simulink library "Centralized_I_Lib_Controller"  (R2024b)
(part 6 of 7)

[dq1,dq2,dq3,dq4,dq5,dq6,t10,t1001,t1002,t1003,t1004,t1005,t1006,t1007,t1009,t101,t1010,t1023,t1024,t1025,t1026,t1027,t1029,t1030,t1032,t1033,t1034,t1035,t1037,t1038,t1039,t1041,t1042,t1043,t1046,t1047,t1048,t105,t1053,t106,t1063,t1068,t1069,t107,t1070,t1071,t1073,t1074,t1075,t1076,t1077,t1078,t1079,t108,t1080,t1081,t1083,t1084,t1086,t1087,t1089,t109,t1090,t1091,t1092,t1095,t1096,t1097,t1098,t11,t110,t1100,t1103,t111,t1115,t1116,t1117,t1118,t1119,t112,t1120,t1122,t1123,t1124,t1126,t1127,t1128,t1129,t113,t1130,t1131,t1132,t1133,t1134,t114,t1148,t1149,t1150,t1151,t1152,t1153,t1155,t1156,t1157,t1158,t1159,t1160,t1162,t1163,t1164,t1166,t1169,t1170,t1171,t1172,t1173,t1174,t1179,t1180,t1182,t1183,t1186,t1187,t1188,t1189,t1191,t1192,t1193,t1194,t1195,t1196,t1198,t1199,t12,t1201,t1202,t1203,t1204,t1205,t1206,t1207,t1208,t1210,t1211,t1212,t1214,t1215,t1217,t1218,t1219,t1220,t1221,t1222,t1224,t1227,t1228,t1229,t123,t1230,t1231,t1233,t1234,t1235,t1239,t124,t1240,t1241,t1242,t1243,t1244,t1245,t1246,t1247,t125,t1250,t1251,t1252,t1253,t1254,t1256,t126,t1263,t1266,t127,t1274,t128,t1284,t1285,t1287,t1288,t1289,t129,t1290,t1291,t1293,t1295,t1296,t1297,t1298,t1299,t13,t130,t1300,t1301,t1308,t1309,t1313,t1317,t1318,t1319,t1320,t1323,t1324,t1325,t1326,t1327,t1328,t1329,t1331,t1332,t1333,t1334,t1339,t1343,t1344,t1345,t1346,t1347,t1349,t1351,t1352,t1353,t1354,t1356,t1357,t1358,t1359,t1360,t1361,t1362,t1363,t1364,t1365,t1366,t1368,t1369,t137,t1371,t1373,t1375,t1376,t1377,t1378,t1379,t1380,t1383,t1385,t1386,t1387,t1388,t1389,t1390,t1391,t1392,t1393,t1394,t1395,t1396,t1397,t1398,t1399,t140,t1405,t1406,t141,t1410,t1411,t1412,t1413,t1414,t1415,t1416,t1417,t1419,t1420,t1421,t1422,t1423,t1424,t1426,t1427,t1428,t1429,t143,t1430,t1431,t1432,t1433,t1434,t1435,t1438,t1439,t1440,t1441,t1442,t1443,t1445,t1446,t1448,t1450,t1452,t1453,t1455,t1456,t1457,t1458,t1459,t1460,t1461,t1462,t1463,t1464,t1465,t1466,t1467,t1468,t1469,t1470,t1473,t1477,t1479,t1480,t1481,t1482,t1484,t1488,t1490,t1491,t1492,t1493,t1494,t1495,t1496,t1500,t1505,t1507,t1508,t1510,t1511,t1512,t1513,t1516,t1517,t1518,t1519,t1522,t1523,t1524,t1525,t1526,t1528,t1541,t1542,t1543,t1545,t1546,t1547,t1548,t1549,t1551,t1552,t1553,t1554,t1555,t1556,t1557,t1558,t1559,t1560,t1571,t1572,t1573,t1575,t1576,t1577,t1578,t1579,t1580,t1581,t1582,t1583,t1584,t1585,t1586,t1587,t159,t1592,t1594,t1595,t1596,t1606,t1609,t1610,t1611,t1613,t1615,t1619,t162,t1620,t163,t1636,t1637,t1639,t164,t1641,t1642,t1643,t1644,t1645,t1646,t165,t1653,t1655,t1656,t1659,t166,t1660,t1661,t1662,t1663,t1664,t1665,t1666,t1668,t1669,t167,t1670,t1671,t1672,t1673,t1675,t1676,t1677,t1678,t1679,t168,t1680,t1681,t1682,t1684,t1685,t1686,t1687,t1688,t1689,t1690,t1691,t1692,t1693,t1694,t1696,t1697,t1698,t1700,t1701,t1702,t1703,t1705,t1706,t1707,t1709,t1710,t1711,t1713,t1716,t1717,t1718,t1719,t1720,t1721,t1723,t1726,t1727,t1728,t1730,t1732,t1735,t1739,t1744,t1745,t1749,t1750,t1751,t1752,t1753,t1754,t1755,t1756,t1758,t1759,t1760,t1761,t1762,t1763,t1764,t1766,t1768,t177,t1771,t1772,t1773,t1776,t1777,t1778,t1779,t178,t1785,t1787,t1789,t179,t1790,t1795,t1796,t1799,t18,t1800,t1801,t1803,t1804,t1806,t1815,t1816,t1817,t1818,t1819,t182,t1820,t1821,t1822,t1823,t1824,t1825,t1826,t1827,t1828,t1829,t183,t1830,t1831,t1832,t1833,t1835,t1836,t1837,t1839,t184,t1840,t1841,t1842,t1843,t1844,t1845,t1847,t1848,t1849,t185,t1850,t1851,t1852,t1853,t1854,t1856,t1857,t1858,t186,t1860,t1861,t1864,t1865,t1866,t1867,t1868,t1869,t187,t1874,t1876,t1877,t1878,t1879,t188,t1882,t1883,t1889,t189,t1893,t1895,t1896,t1897,t1898,t1899,t19,t1900,t1901,t1902,t1903,t1904,t1905,t1906,t1907,t1908,t1909,t191,t1911,t1912,t1913,t1914,t1917,t1919,t1920,t1921,t1922,t1925,t1926,t1928,t193,t1930,t1931,t1933,t1934,t1935,t1936,t1937,t1939,t194,t1942,t1943,t1944,t1947,t1949,t195,t1955,t1958,t1959,t1962,t1964,t1966,t1973,t1991,t1992,t1993,t1994,t1995,t1996,t1997,t1998,t2,t20,t200,t2000,t2001,t2002,t2003,t2004,t2005,t2006,t2009,t2010,t2012,t2013,t2014,t2015,t2016,t2017,t2018,t202,t2020,t2021,t2023,t2024,t2025,t2027,t2028,t2029,t203,t2030,t2034,t2036,t2037,t2038,t2039,t204,t2040,t2043,t2044,t2045,t2050,t2053,t2054,t2055,t2056,t2058,t2059,t2061,t2063,t2066,t2067,t2068,t2069,t2072,t2074,t2075,t2078,t2079,t208,t2080,t2083,t2084,t2085,t2086,t2087,t2088,t2089,t2090,t2092,t2094,t2096,t2097,t21,t210,t2103,t2107,t2109,t211,t2110,t2111,t2112,t2115,t2116,t2117,t2118,t212,t2120,t2121,t2123,t2124,t2125,t2126,t2127,t2129,t2132,t2133,t2134,t2135,t2136,t2138,t2139,t214,t2140,t2141,t2147,t2148,t2149,t215,t2150,t2151,t2152,t2157,t2158,t2159,t216,t2161,t2168,t2169,t2171,t2178,t2179,t2181,t2185,t2191,t2193,t22,t2200,t2201,t2202,t2203,t2204,t2205,t2206,t2207,t2208,t2212,t2214,t2216,t2217,t2219,t2220,t2221,t2222,t2223,t2224,t2225,t2227,t2228,t2229,t2231,t2233,t2234,t2235,t2236,t2237,t2238,t2239,t224,t2245,t2246,t2247,t2248,t2250,t2252,t2254,t2258,t2259,t2262,t227,t2271,t2272,t2273,t2274,t2276,t2277,t228,t2280,t2281,t2283,t2284,t2285,t2287,t229,t2290,t2292,t2293,t2295,t230,t2303,t2304,t2305,t2307,t2308,t231,t2310,t2314,t2318,t2319,t2320,t2322,t2323,t2324,t2325,t2326,t2327,t2336,t234,t2342,t2343,t2347,t2348,t2349,t2350,t2353,t2357,t2358,t2362,t2363,t2364,t237,t2370,t2372,t2373,t2375,t2378,t2379,t2381,t2382,t2383,t2385,t2387,t2394,t2395,t2396,t2397,t2398,t2400,t2401,t2403,t2404,t2405,t2409,t2410,t2411,t2412,t2413,t2414,t2415,t2416,t2417,t2419,t242,t2421,t2422,t2423,t2425,t2426,t243,t2430,t2431,t2432,t2433,t2436,t2437,t2438,t2439,t244,t2440,t2445,t2446,t2447,t2449,t245,t2450,t2451,t2452,t2453,t2454,t2455,t2456,t2457,t2459,t246,t2462,t2463,t2464,t2465,t2466,t2467,t2469,t247,t2470,t2471,t2472,t2473,t2474,t2475,t2477,t2478,t2479,t248,t2480,t2481,t2482,t2483,t2484,t2485,t2486,t2487,t2488,t249,t2491,t2498,t2499,t25,t250,t2500,t2501,t2504,t2506,t2507,t2508,t2509,t251,t2515,t252,t2524,t2525,t2527,t2529,t253,t2531,t2536,t2542,t2543,t2546,t255,t2551,t2552,t2553,t2555,t2559,t256,t2560,t2564,t2565,t2566,t2567,t2568,t2569,t2571,t2572,t2574,t2575,t2576,t2578,t2580,t2581,t2582,t2583,t2585,t2586,t2588,t259,t2591,t2593,t2594,t2595,t2598,t2599,t26,t260,t2600,t2601,t2603,t2604,t2605,t2607,t2608,t2609,t261,t2610,t2611,t2612,t2614,t2615,t2617,t2618,t262,t2621,t2622,t2625,t2628,t2629,t263,t2632,t2634,t2641,t2643,t2644,t2645,t2646,t2648,t2649,t265,t2650,t2651,t2652,t2655,t2656,t2657,t2658,t2659,t2660,t2661,t2662,t2663,t2667,t267,t2672,t2673,t2674,t2675,t2679,t2680,t269,t2691,t2692,t2694,t2695,t2698,t27,t2700,t2701,t2702,t2703,t2705,t2711,t2712,t2713,t2714,t2715,t2716,t2718,t2719,t2720,t2721,t2722,t2725,t2726,t2727,t2729,t2730,t2732,t2733,t2734,t2735,t2736,t2738,t2739,t274,t2740,t2741,t2743,t2747,t2748,t2749,t2752,t2753,t2755,t2756,t276,t2760,t2761,t2763,t2764,t2765,t2766,t2767,t2769,t277,t2770,t2772,t278,t2782,t2783,t2784,t2785,t2786,t2789,t279,t2792,t2793,t2794,t2795,t2796,t28,t2800,t2801,t2803,t2804,t2806,t2809,t281,t2811,t2812,t2813,t2815,t2816,t2817,t2819,t2820,t2821,t2822,t2825,t2827,t2828,t2829,t283,t2830,t2832,t2833,t2834,t2836,t2837,t2839,t2840,t2843,t2844,t2848,t2849,t285,t2850,t2852,t2854,t2855,t2856,t286,t2860,t2861,t2862,t2863,t2864,t2865,t2866,t2867,t2869,t287,t2872,t2873,t2877,t2878,t288,t2880,t2882,t2887,t2888,t2890,t2892,t2894,t2895,t2899,t29,t2900,t2901,t2902,t2903,t2904,t2905,t2906,t2910,t2911,t2912,t2915,t2916,t2917,t2919,t292,t2921,t2922,t2923,t2924,t2925,t2926,t2927,t2928,t2929,t293,t2931,t2932,t2933,t2934,t2937,t2938,t2939,t2940,t2942,t2943,t2944,t2949,t295,t2950,t2951,t2952,t2953,t2954,t2956,t2957,t2959,t296,t2960,t2962,t2964,t2965,t2968,t2969,t297,t2970,t2973,t2975,t2977,t298,t2981,t2984,t2986,t2988,t2989,t299,t2990,t2991,t2992,t2993,t2995,t2996,t2997,t3,t300,t3002,t3003,t3004,t3006,t3007,t3008,t3009,t301,t3010,t3011,t3012,t3013,t3015,t3016,t3018,t3019,t3025,t3026,t3028,t303,t3030,t3033,t3034,t3035,t3037,t3039,t304,t3040,t3043,t3045,t3046,t3047,t3049,t305,t3050,t3054,t3056,t3058,t3059,t3060,t3061,t3063,t3064,t3065,t3066,t3067,t3068,t3069,t3070,t3071,t3072,t3073,t3074,t3075,t3076,t3077,t3078,t3079,t308,t3085,t3087,t3088,t3089,t309,t3090,t3091,t3092,t3094,t3095,t3096,t3097,t3098,t3099,t3100,t3101,t3102,t3104,t3106,t3108,t3109,t311,t3110,t3111,t3112,t3119,t312,t3121,t3123,t3124,t3125,t3129,t313,t3130,t3131,t3133,t3136,t3138,t3139,t314,t3144,t3146,t3147,t3148,t3149,t3150,t3152,t3153,t3154,t3159,t3164,t3170,t3173,t3174,t3177,t3180,t3181,t3185,t3186,t3187,t3188,t3189,t3192,t3193,t3194,t3195,t3198,t3200,t3201,t3202,t3203,t3204,t3205,t3206,t3207,t3208,t3209,t3210,t3211,t3212,t3213,t3214,t3215,t3216,t3217,t3218,t3219,t3220,t3222,t3223,t3224,t3225,t3226,t3227,t3228,t3231,t3232,t3233,t3234,t3235,t3236,t3237,t3238,t3239,t3242,t3245,t3246,t3247,t3249,t3250,t3252,t3253,t3254,t3255,t3256,t3258,t3260,t3262,t3265,t3269,t3270,t3271,t3273,t3274,t3275,t328,t3280,t3281,t3282,t3283,t3284,t3286,t3287,t3288,t329,t3296,t3297,t3298,t330,t3300,t3303,t3304,t3305,t3306,t3307,t3308,t331,t3315,t3316,t3318,t332,t3322,t3323,t3324,t3326,t3327,t3328,t3329,t333,t3330,t3331,t3332,t3333,t3334,t3335,t3336,t3339,t334,t3342,t3345,t3346,t3347,t3348,t3352,t3353,t3356,t3358,t3359,t336,t3361,t3362,t3363,t3364,t3365,t3366,t3367,t337,t3372,t3374,t3375,t3377,t3378,t3379,t338,t3380,t3384,t3385,t3386,t3387,t339,t3394,t3395,t3396,t3397,t3399,t3401,t3402,t3405,t341,t3410,t3411,t3412,t3413,t3414,t3416,t3419,t342,t3421,t3422,t3424,t3425,t3426,t3427,t343,t3430,t3435,t3436,t3437,t3438,t3439,t344,t3440,t3442,t3443,t3444,t3445,t3446,t3449,t345,t3452,t3453,t3454,t3455,t3456,t3458,t3459,t346,t3463,t3466,t3467,t347,t3470,t3471,t3472,t3473,t3474,t3475,t3476,t3477,t348,t3480,t3481,t3482,t3483,t3484,t3485,t3487,t3488,t3489,t349,t3491,t3492,t3493,t3494,t3496,t3498,t3499,t350,t3501,t3502,t3504,t3506,t3507,t3508,t3509,t3511,t3512,t3513,t3515,t3516,t3519,t352,t3520,t3521,t3522,t3523,t3526,t3527,t3528,t3529,t353,t3531,t3532,t3533,t3535,t3536,t3537,t3538,t354,t3541,t3542,t3543,t3544,t3545,t3548,t3549,t355,t3552,t3553,t3554,t3555,t3559,t356,t3561,t3564,t3565,t3566,t3567,t3568,t3569,t357,t3571,t3573,t3575,t3576,t3578,t3579,t358,t3582,t3586,t3587,t3588,t3590,t3591,t3592,t3593,t3596,t3598,t3599,t360,t3600,t3601,t3602,t3603,t3604,t3606,t3608,t3609,t3610,t3611,t3612,t3613,t3614,t3615,t3617,t3620,t3621,t3622,t3623,t3626,t3627,t3628,t3629,t3630,t3631,t3632,t3633,t3634,t3636,t3638,t3639,t3640,t3641,t3642,t3643,t3645,t3646,t3648,t3649,t3650,t3652,t3653,t3654,t3655,t3656,t3657,t3658,t3660,t3663,t3667,t3668,t3670,t3671,t3673,t3674,t3675,t3676,t3677,t3679,t3680,t3681,t3682,t3683,t3684,t3686,t3687,t3688,t3689,t369,t3690,t3691,t3692,t3694,t3695,t3696,t3697,t3698,t3699,t370,t3700,t3701,t3702,t3703,t3704,t3705,t3708,t3709,t3710,t3711,t3712,t3713,t3714,t3715,t3717,t3718,t3719,t372,t3720,t3721,t3722,t3723,t3724,t3725,t3726,t3727,t3728,t3729,t373,t3730,t3732,t3733,t3734,t3735,t3736,t3737,t3738,t3739,t374,t3740,t3741,t3742,t3743,t3744,t3745,t3747,t3748,t3749,t375,t3750,t3751,t3752,t3754,t3755,t3756,t3757,t3758,t3759,t376,t3760,t3763,t3764,t3765,t3766,t3767,t3768,t3769,t3770,t3771,t3772,t3774,t3775,t3776,t3777,t3778,t3780,t3781,t3782,t3785,t3786,t3787,t3789,t379,t3790,t3792,t3793,t3794,t3796,t3798,t380,t3801,t3802,t3804,t3805,t3806,t3807,t3808,t3809,t3810,t3811,t3812,t3813,t3814,t3815,t3816,t3817,t3818,t3820,t3821,t3822,t3823,t3824,t3825,t3826,t3827,t3828,t3829,t3831,t3832,t3833,t3837,t3838,t3839,t384,t3840,t3841,t3846,t3847,t3848,t3849,t3850,t3851,t3852,t3854,t3856,t3857,t386,t3860,t3861,t3862,t3863,t3864,t3865,t3868,t3869,t387,t3871,t3872,t3874,t3875,t3876,t3878,t388,t3882,t3884,t3885,t3886,t3887,t3888,t3889,t389,t3890,t3891,t3892,t3893,t3894,t3895,t3896,t3897,t3898,t3899,t3900,t3901,t3902,t3903,t3904,t3906,t3908,t3909,t3910,t3912,t3913,t3915,t3916,t3917,t3918,t3919,t3920,t3921,t3922,t3923,t3924,t3925,t3926,t3927,t3928,t393,t3930,t3931,t3932,t3935,t3936,t3939,t3941,t3944,t3945,t3946,t3947,t3948,t3949,t395,t3950,t3951,t3953,t3954,t3955,t3956,t3957,t3959,t3960,t3964,t3965,t3966,t3967,t3968,t397,t3970,t3971,t3972,t3976,t3977,t3981,t3982,t3985,t3988,t3989,t399,t3990,t3993,t3994,t3995,t3998,t3999,t4,t400,t4000,t4001,t4002,t4003,t4005,t4006,t4007,t4009,t401,t4011,t4012,t4013,t4014,t4015,t4016,t4017,t4018,t4019,t402,t4022,t4025,t4026,t4028,t4029,t4031,t4032,t4033,t4034,t4035,t4036,t4037,t404,t4041,t4042,t4043,t4044,t4046,t4047,t4048,t405,t4053,t4055,t4056,t4057,t4058,t4059,t4060,t4061,t4062,t4063,t4064,t4065,t4066,t4067,t4068,t407,t4070,t4074,t4075,t4077,t4078,t4079,t408,t4080,t4081,t4082,t4083,t4084,t4085,t4087,t4088,t4089,t4090,t4091,t4092,t4095,t4097,t4099,t410,t4103,t4104,t4105,t4109,t4113,t4115,t4116,t4118,t4119,t4120,t4121,t4122,t4123,t4125,t4126,t4127,t4129,t413,t4131,t4132,t4133,t4134,t4136,t4137,t4138,t4139,t414,t4140,t4142,t4143,t4145,t4147,t4148,t4149,t415,t4150,t4151,t4152,t4153,t4154,t4156,t4159,t416,t4161,t4162,t4165,t4168,t4171,t4172,t4174,t4175,t4176,t4178,t418,t4183,t4185,t4186,t4188,t419,t4190,t4191,t4192,t4194,t4195,t4197,t4198,t4199,t4200,t4202,t4203,t4204,t4206,t4208,t4209,t421,t4210,t4211,t4212,t4213,t4216,t4217,t4218,t4219,t4220,t4221,t4222,t4223,t4224,t4225,t4226,t4230,t4231,t4232,t4233,t4234,t4235,t4238,t4240,t4241,t4242,t4243,t4244,t4245,t4246,t4247,t4248,t4249,t425,t4250,t4251,t4252,t4255,t4256,t4257,t4258,t4259,t4260,t4261,t4262,t4263,t4264,t4265,t4268,t4269,t4270,t4271,t4274,t4275,t4276,t4277,t4278,t4279,t4280,t4282,t4283,t4284,t4286,t4287,t4288,t4292,t4294,t4295,t4296,t4300,t4301,t4305,t4308,t4309,t4310,t4311,t4312,t4313,t4316,t4317,t4318,t4319,t432,t4320,t4323,t4324,t4325,t4326,t4327,t4328,t4329,t433,t4330,t4331,t4332,t4333,t4334,t4335,t4336,t4338,t434,t4341,t4342,t4343,t4344,t4345,t4347,t435,t4350,t4352,t4354,t436,t4361,t4362,t4364,t4365,t4366,t4367,t4368,t4369,t437,t4370,t4371,t4372,t4374,t4375,t4376,t4377,t4378,t4379,t4380,t4381,t4384,t4385,t4386,t4387,t4388,t4389,t439,t4390,t4391,t4392,t4393,t4394,t4396,t4399,t440,t4400,t4402,t4403,t4405,t4406,t4407,t4408,t4409,t441,t4410,t4414,t4415,t4416,t4417,t4418,t4419,t4420,t4421,t4422,t4423,t4424,t4426,t4428,t4429,t443,t4430,t4433,t4435,t4436,t4438,t4439,t444,t4440,t4442,t4444,t4445,t4448,t4449,t4451,t4452,t4454,t4455,t4456,t4457,t4458,t4459,t446,t4463,t4466,t4469,t4470,t4471,t4473,t4474,t4475,t4476,t4477,t4478,t4479,t4482,t4483,t4484,t4487,t4488,t4493,t4495,t4496,t4497,t4498,t4499,t4503,t4505,t4507,t4508,t4511,t4512,t4513,t4514,t4515,t4516,t4517,t4518,t4519,t4520,t4521,t4526,t4528,t4529,t453,t4531,t4532,t4533,t4534,t4535,t4536,t4537,t4538,t4539,t4540,t4541,t4542,t4543,t4544,t4545,t4546,t4547,t4549,t4550,t4551,t4554,t4555,t4556,t4557,t4558,t4559,t4561,t4562,t4563,t4564,t4565,t4566,t4567,t4568,t4569,t4570,t4571,t4572,t4573,t4574,t4575,t4576,t4578,t4579,t4580,t4581,t4582,t4584,t4585,t4589,t4590,t4592,t4593,t4594,t4595,t4597,t4598,t4599,t460,t4601,t4602,t4603,t4604,t4606,t4608,t4609,t4610,t4611,t4612,t4613,t4614,t4615,t4616,t4617,t4618,t4619,t4620,t4621,t4622,t4623,t4625,t4626,t4627,t4628,t4629,t463,t4631,t4632,t4633,t4636,t4639,t4640,t4641,t4642,t4644,t4645,t4647,t4648,t4649,t465,t4650,t4651,t4652,t4653,t4655,t4656,t4658,t4660,t4661,t4664,t4665,t4666,t4669,t4670,t4671,t4672,t4673,t4674,t4675,t4676,t4679,t4683,t4685,t4686,t4691,t4692,t4694,t4695,t4697,t4698,t4699,t4702,t4704,t4706,t4710,t4712,t4713,t4714,t4717,t4718,t4719,t472,t4720,t4722,t4723,t4726,t4729,t4730,t4731,t4732,t4733,t4735,t4736,t4737,t4738,t4739,t4740,t4742,t4743,t4744,t4746,t4747,t4749,t475,t4750,t4751,t4753,t4754,t4756,t4757,t4759,t4760,t4761,t4762,t4763,t4764,t4765,t4766,t4767,t4768,t4769,t4770,t4771,t4772,t4773,t4774,t4775,t4776,t4777,t4778,t4779,t478,t4780,t4781,t4782,t4783,t4784,t4785,t4786,t4787,t4789,t4791,t4792,t4793,t4794,t4795,t4797,t4798,t4799,t48,t4800,t4801,t4802,t4804,t4805,t4806,t4807,t4808,t4811,t4812,t4813,t4814,t4815,t4816,t4817,t4818,t4819,t4820,t4821,t4822,t4823,t4824,t4825,t4826,t4827,t4828,t4829,t4830,t4831,t4832,t4833,t4835,t4837,t4838,t4840,t4841,t4842,t4844,t4845,t4846,t4847,t4849,t4850,t4851,t4852,t4853,t4854,t4855,t4856,t4857,t4858,t4859,t4860,t4861,t4862,t4863,t4864,t4865,t4867,t4868,t4869,t4870,t4872,t4873,t4874,t4875,t4876,t4879,t488,t4880,t4881,t4883,t4884,t4885,t4886,t4887,t4888,t4889,t4892,t4895,t4896,t4898,t49,t490,t4903,t4905,t4906,t4907,t4908,t4909,t491,t4910,t4911,t4912,t4913,t4914,t4915,t4916,t4917,t4918,t4919,t4920,t4921,t4923,t4924,t4925,t4926,t4927,t4928,t4929,t4930,t4931,t4932,t4933,t4934,t4935,t4937,t4938,t494,t4940,t4942,t4943,t4946,t4948,t4949,t4950,t4953,t4955,t4957,t4958,t496,t4961,t4962,t4964,t4965,t4967,t4968,t497,t4970,t4971,t4972,t4973,t4975,t4976,t4977,t4978,t4979,t498,t4980,t4983,t4984,t4985,t4987,t4988,t499,t4990,t4991,t4992,t4995,t4996,t4998,t5,t50,t500,t5000,t5001,t5003,t5006,t5007,t5009,t501,t5010,t5012,t5014,t5015,t5016,t502,t5020,t5022,t5024,t5025,t5026,t5027,t5030,t5032,t5033,t5034,t5035,t5036,t5038,t5039,t504,t5041,t5042,t5043,t5044,t5045,t5046,t5047,t5048,t505,t5051,t5052,t5054,t5055,t5056,t5058,t5059,t5060,t5061,t5062,t5063,t5064,t5065,t5066,t5067,t5068,t5069,t5070,t5071,t5072,t5073,t5074,t5075,t5076,t5077,t5079,t508,t5080,t5081,t5082,t5083,t5084,t5085,t5086,t5087,t5089,t509,t5090,t5091,t5094,t5095,t5097,t5099,t51,t510,t5100,t5101,t5102,t5105,t5108,t5109,t511,t5111,t5114,t5115,t5116,t5117,t5118,t5119,t512,t5120,t5121,t5122,t5125,t5126,t5127,t5129,t5131,t5132,t5133,t5135,t5136,t5137,t5138,t5139,t514,t5140,t5141,t5143,t5144,t5145,t5146,t5147,t5148,t5149,t515,t5150,t5151,t5153,t5154,t5156,t5158,t516,t5161,t5163,t5164,t5165,t5166,t5167,t5168,t5169,t517,t5170,t5173,t5174,t5176,t5179,t518,t5180,t5181,t5185,t5186,t5187,t5188,t5189,t5190,t5191,t5193,t5194,t5195,t5196,t5200,t5202,t5203,t5207,t5208,t5209,t521,t5210,t5213,t5215,t5216,t5218,t5219,t5221,t5222,t5223,t5224,t5225,t5227,t5229,t523,t5231,t5235,t5236,t5239,t524,t5241,t5242,t5243,t5244,t5245,t5246,t5247,t5250,t5251,t5252,t5253,t5257,t5258,t5259,t5263,t5264,t5265,t5266,t5269,t527,t5274,t5276,t5277,t5278,t5279,t528,t5280,t5281,t5283,t5284,t5285,t5288,t5289,t529,t5290,t5291,t5292,t5293,t5294,t5295,t5296,t5297,t5298,t5299,t53,t530,t5300,t5301,t5302,t5303,t5304,t5305,t5306,t5307,t5308,t5309,t531,t5310,t5312,t5317,t5319,t5322,t5324,t5325,t5326,t5328,t5329,t5330,t5332,t5333,t5334,t5336,t5338,t5339,t534,t5340,t5341,t5342,t5343,t5344,t5345,t5348,t5349,t535,t5350,t5353,t5354,t5355,t5356,t5357,t5358,t5359,t536,t5360,t5361,t5362,t5363,t5364,t5365,t5366,t5369,t5370,t5371,t5372,t5374,t5375,t5376,t5377,t5380,t5382,t5383,t5384,t5385,t5386,t5387,t5388,t5389,t539,t5390,t5391,t5392,t5393,t5394,t5395,t5396,t5397,t5398,t5399,t54,t540,t5400,t5401,t5402,t5403,t5405,t5406,t5407,t5408,t5409,t5410,t5411,t5412,t5413,t5414,t5415,t5416,t5417,t5418,t5419,t542,t5420,t5421,t5422,t5423,t5424,t5425,t5426,t5427,t5428,t5429,t543,t5431,t5432,t5433,t5435,t5436,t5439,t5441,t5442,t5444,t5445,t5446,t5447,t5448,t5449,t5450,t5451,t5452,t5453,t5454,t5455,t5456,t5457,t5458,t5459,t5460,t5461,t5465,t5467,t5468,t5469,t547,t5471,t5472,t5473,t5474,t5475,t5476,t5477,t5478,t548,t5480,t5482,t5483,t5484,t5486,t5490,t5491,t5492,t5493,t5494,t5495,t5496,t5497,t5498,t5499,t55,t5500,t5501,t5502,t5503,t5504,t5505,t5506,t5507,t5508,t5509,t5510,t5511,t5512,t5513,t5514,t5517,t5518,t5519,t5522,t5526,t5527,t5528,t5529,t553,t5530,t5531,t5532,t5533,t5534,t5536,t5537,t5538,t5539,t5540,t5542,t5543,t5544,t5545,t5546,t5547,t5548,t5549,t555,t5550,t5551,t5552,t5553,t5554,t5556,t5557,t5559,t556,t5561,t5562,t5563,t5564,t557,t5573,t5574,t5575,t5576,t5577,t5578,t5579,t558,t5581,t5582,t5583,t5584,t5586,t5587,t5588,t5589,t559,t5590,t5591,t5592,t5593,t5594,t5595,t5596,t5597,t5598,t5599,t56,t560,t5600,t5601,t5602,t5603,t5604,t5605,t5606,t5607,t5608,t5609,t561,t5611,t5612,t5613,t5614,t5615,t5616,t5617,t5618,t5619,t562,t5620,t5621,t5622,t5625,t5627,t5628,t5629,t5630,t5631,t5632,t5634,t5635,t5636,t5637,t5638,t5639,t5644,t5646,t5647,t5648,t5649,t565,t5650,t5651,t5652,t5653,t5654,t5656,t5657,t5658,t5659,t566,t5660,t5661,t5662,t5663,t5664,t5665,t5670,t5671,t5673,t5674,t5675,t5676,t5677,t5678,t5679,t5680,t5681,t5683,t5684,t5685,t5686,t569,t5690,t5692,t5696,t5697,t5698,t5699,t57,t5701,t5702,t5703,t5704,t5705,t5706,t5710,t5711,t5713,t5715,t5716,t5717,t5718,t5719,t5720,t5722,t5723,t5724,t5725,t5726,t5727,t5728,t5729,t5730,t5731,t5732,t5733,t5734,t5735,t5736,t5737,t5741,t5744,t5745,t5747,t5748,t5749,t5750,t5752,t5753,t5755,t5756,t5757,t5759,t5761,t5762,t5763,t5764,t5766,t5767,t5770,t5771,t5773,t5774,t5775,t5776,t5777,t5778,t5779,t5780,t5781,t5783,t5784,t5785,t5786,t5788,t5789,t5792,t5796,t5797,t58,t5800,t5801,t5802,t5803,t5804,t5805,t5806,t5807,t5808,t5809,t5810,t5811,t5812,t5813,t5814,t5815,t5816,t5817,t5818,t5819,t5820,t5822,t5823,t5824,t5825,t5826,t5827,t5828,t5829,t5831,t5832,t5833,t5835,t5836,t5837,t5838,t5840,t5841,t5842,t5843,t5844,t5845,t5847,t5849,t5850,t5851,t5853,t5854,t5855,t5857,t5859,t5860,t5861,t5862,t5865,t5866,t5867,t5868,t5870,t5871,t5873,t5876,t5877,t5878,t5879,t5882,t5883,t5884,t5886,t5888,t5890,t5891,t5892,t5893,t5895,t5896,t5897,t5898,t5899,t5901,t5903,t5905,t5906,t5907,t5908,t5909,t5910,t5911,t5912,t5913,t5914,t5916,t5917,t5919,t5923,t5924,t5928,t5930,t5931,t5933,t5934,t5935,t5936,t5937,t5939,t594,t5942,t5944,t5945,t5946,t5947,t5949,t595,t5950,t5952,t5953,t5954,t5955,t5956,t5958,t5959,t596,t5960,t5961,t5962,t5963,t5964,t5965,t5966,t5967,t5968,t5969,t597,t5970,t5971,t5972,t5973,t5974,t5975,t5976,t5977,t5978,t5979,t598,t5980,t5982,t5983,t5984,t5985,t5986,t5987,t5988,t5989,t599,t5990,t5991,t5992,t5993,t5994,t5995,t5997,t5998,t5999,t6,t60,t600,t6000,t6001,t6002,t6003,t6004,t6005,t6006,t6007,t6008,t6009,t601,t6010,t6011,t6014,t6015,t6016,t6017,t6019,t602,t6020,t6021,t6022,t6023,t6024,t6025,t6026,t6027,t6028,t6029,t6030,t6031,t6033,t6038,t6039,t6042,t6043,t6044,t6045,t6046,t6047,t6048,t6049,t605,t6050,t6051,t6052,t6053,t6054,t6055,t6056,t6057,t6058,t6059,t606,t6060,t6061,t6062,t6063,t6065,t6066,t6067,t6069,t6070,t6071,t6072,t6073,t6075,t6076,t6077,t6078,t608,t6081,t6082,t6084,t6085,t6086,t6087,t6089,t609,t6090,t6091,t6092,t6093,t6094,t6096,t6097,t6098,t6099,t61,t610,t6100,t6101,t6106,t6108,t6109,t611,t6111,t6112,t6115,t6116,t6117,t6118,t6119,t6120,t6121,t6123,t6124,t6125,t6126,t6127,t6128,t6129,t6130,t6131,t6132,t6134,t6135,t6136,t6137,t6138,t6139,t614,t6140,t6141,t6145,t6146,t6147,t6148,t6149,t6150,t6151,t6152,t6153,t6154,t6155,t6156,t6157,t6159,t616,t6160,t6161,t6162,t6163,t6164,t6165,t6166,t6167,t617,t6178,t6179,t618,t6180,t6181,t6182,t6183,t6184,t6185,t6186,t6187,t6188,t6189,t619,t6190,t6191,t6192,t6193,t6195,t6196,t6197,t62,t620,t6200,t6201,t6203,t6204,t6206,t6207,t6210,t6211,t6213,t6214,t6216,t6218,t6219,t622,t6222,t6224,t6225,t6226,t6229,t6231,t6232,t6234,t6235,t6236,t6237,t6239,t6241,t6242,t6244,t6247,t6248,t6249,t625,t6252,t6253,t6254,t6255,t6256,t6257,t6258,t626,t6260,t6261,t6262,t6263,t6264,t6265,t6266,t6267,t6268,t6269,t6270,t6271,t6272,t6273,t6274,t6275,t6276,t6277,t6278,t6279,t6280,t6281,t6282,t6283,t6284,t6286,t6288,t6290,t6293,t6294,t6295,t6296,t6298,t6299,t63,t6300,t6301,t6302,t6303,t6304,t6305,t6306,t6307,t6312,t6313,t6315,t6316,t6317,t6318,t6321,t6322,t6323,t6327,t6328,t6332,t6334,t6335,t6337,t6339,t634,t6340,t6341,t6342,t6343,t6344,t6345,t6346,t6349,t635,t6350,t6351,t6352,t6353,t6354,t6355,t6356,t6357,t6359,t636,t6360,t6362,t6363,t6364,t6365,t6366,t6367,t6368,t6369,t637,t6370,t6371,t6372,t6373,t6375,t6376,t6377,t6379,t638,t6383,t6385,t6386,t6387,t6388,t6389,t639,t6390,t6391,t6395,t6397,t6399,t640,t6400,t6401,t6403,t6404,t6405,t6406,t6407,t641,t6411,t6412,t6417,t6418,t6421,t6422,t6423,t6424,t6425,t6426,t6427,t6429,t643,t6431,t6434,t6435,t6436,t6437,t6438,t6439,t6440,t6441,t6442,t6443,t6444,t6445,t6446,t6447,t645,t6452,t6453,t6454,t6455,t6456,t6457,t6458,t6460,t6461,t6465,t6467,t6468,t6469,t647,t6470,t6472,t6473,t6474,t6475,t6481,t6483,t6484,t6485,t6486,t6487,t6488,t6489,t649,t6490,t6491,t6492,t6493,t6498,t6499,t650,t6500,t6501,t6502,t6503,t6504,t6509,t651,t6510,t6513,t6516,t652,t6520,t6521,t6522,t6523,t6525,t6526,t6527,t6528,t6529,t653,t6530,t6531,t6532,t6533,t6534,t6536,t6537,t6538,t6539,t6540,t6541,t6542,t6543,t6544,t6545,t6549,t6557,t6558,t6559,t656,t6560,t6561,t6562,t6563,t6564,t6566,t6569,t657,t6570,t6574,t6575,t6579,t658,t6582,t6583,t6584,t6585,t659,t6591,t6592,t6594,t6595,t6596,t6597,t6599,t660,t6600,t6601,t6602,t6603,t6604,t6605,t6606,t6607,t6608,t6609,t661,t6610,t6611,t6612,t6613,t6616,t6618,t6619,t662,t6621,t6623,t6624,t6625,t6628,t6629,t663,t6632,t6634,t6635,t6636,t6637,t6639,t664,t6640,t6641,t6642,t6643,t6644,t6645,t6646,t6648,t6649,t6652,t6654,t6655,t6657,t6658,t6659,t666,t6661,t6662,t6663,t6664,t6665,t6667,t6668,t6669,t667,t6670,t6675,t6678,t6679,t6680,t6681,t6686,t6687,t6689,t6692,t6693,t6694,t6695,t6696,t6697,t6698,t6699,t670,t6700,t6702,t6703,t6704,t6705,t6706,t6711,t6712,t6714,t6715,t6717,t6718,t6719,t6720,t6721,t6722,t6725,t6727,t6728,t6733,t6734,t6735,t6736,t6738,t6739,t6740,t6741,t6742,t6743,t6744,t6746,t6747,t6749,t675,t6750,t6754,t6755,t6757,t6758,t6759,t676,t6760,t6763,t6764,t6766,t6767,t677,t6770,t6771,t6772,t6775,t6776,t678,t6782,t6783,t6784,t6786,t6789,t679,t6790,t6796,t6799,t680,t6800,t6804,t6805,t6806,t6807,t6808,t6809,t681,t6811,t6813,t6814,t6825,t6826,t6827,t6829,t683,t6830,t6831,t6834,t6838,t684,t6843,t685,t6851,t6853,t6856,t6857,t686,t6860,t6862,t6863,t6864,t6865,t6866,t6869,t687,t6870,t6871,t6872,t6876,t6879,t688,t6880,t6881,t6882,t6883,t6884,t6885,t6886,t6898,t690,t6902,t6903,t6905,t6906,t691,t6910,t6911,t6913,t6914,t6919,t692,t6920,t6921,t6925,t6926,t6927,t693,t6935,t6936,t6937,t6938,t6944,t6945,t6946,t6947,t6948,t6949,t6950,t6951,t6952,t6953,t6954,t6955,t6956,t696,t6966,t6967,t699,t6998,t6999,t7,t700,t7010,t7011,t7019,t702,t7020,t7023,t7026,t7027,t7028,t703,t7031,t7032,t7035,t7042,t7043,t7044,t7050,t7051,t7052,t706,t7061,t7062,t7063,t7064,t7065,t7066,t708,t7122,t7123,t7127,t7128,t7129,t7168,t7170,t7174,t7176,t7200,t7201,t7205,t7206,t7209,t721,t7210,t7212,t7213,t7224,t7225,t7229,t7230,t724,t728,t7286,t7297,t7298,t7299,t7300,t7301,t7302,t7303,t7304,t7305,t7307,t731,t7311,t7312,t7314,t7315,t7323,t7327,t7328,t7329,t7334,t7346,t7347,t735,t7353,t7357,t736,t7361,t7362,t7363,t7365,t7366,t7367,t7368,t7369,t737,t7370,t7371,t7372,t7378,t738,t7393,t7394,t7395,t7396,t7397,t7398,t7399,t740,t7400,t7401,t7402,t7403,t7404,t7405,t7406,t7410,t7412,t7413,t7417,t7420,t7422,t7423,t7425,t7428,t7429,t7430,t7433,t7434,t7438,t7442,t7459,t746,t7463,t7464,t747,t748,t7482,t752,t754,t7557,t756,t7564,t758,t759,t7600,t7602,t761,t763,t764,t7659,t766,t767,t768,t771,t772,t7721,t7725,t7727,t7729,t776,t7764,t781,t782,t7897,t7902,t793,t795,t7966,t798,t7999,t8,t8021,t8038,t8046,t823,t826,t827,t828,t829,t832,t833,t834,t835,t836,t837,t838,t839,t84,t842,t844,t847,t848,t849,t85,t850,t852,t854,t858,t859,t86,t861,t864,t868,t87,t879,t884,t885,t888,t889,t890,t891,t892,t893,t894,t896,t897,t898,t899,t9,t90,t900,t901,t902,t903,t904,t905,t906,t907,t909,t911,t912,t913,t914,t915,t916,t917,t918,t919,t92,t921,t929,t930,t931,t932,t933,t934,t936,t937,t938,t940,t941,t943,t944,t945,t947,t949,t950,t951,t952,t953,t954,t956,t957,t964,t965,t966,t967,t968,t969,t97,t970,t972,t973,t974,t975,t976,t977,t978,t98,t981,t982,t984,t986,t987,t988,t99,t990,t991,t992,t993,t994,t996,t997,t999] = ct{:};
t7466 = t2.*t6914.*(t296+t369+t397+t404-t562+t728+t738-t768+t1301+t1500-(t12.*t101)./1.0e+1-(t12.*t106)./1.0e+1).*(-3.0./2.0);
t7467 = t2.*t6914.*(t296+t369+t397+t404-t562+t728+t738-t768+t1301+t1500-(t12.*t101)./1.0e+1-(t12.*t106)./1.0e+1).*(3.0./2.0);
t7469 = (t7011.*t7362)./2.0;
t7470 = (t7010.*t7363)./2.0;
t7474 = t6999.*(t296+t369+t397+t404-t562+t728+t738-t768+t1301+t1500-(t12.*t101)./1.0e+1-(t12.*t106)./1.0e+1).*(-1.0./2.0);
t7475 = t6998.*(t304+t372+t405+t418-t566+t740+t748-t782+t1309+t1505-t12.*t101.*(3.0./1.0e+1)-t12.*t106.*(3.0./1.0e+1)).*(-1.0./2.0);
t7478 = (t6998.*(t304+t372+t405+t418-t566+t740+t748-t782+t1309+t1505-t12.*t101.*(3.0./1.0e+1)-t12.*t106.*(3.0./1.0e+1)))./2.0;
t7479 = t7020.*(t191.*(2.0./5.0)+t297+t413+t463+t504-t766-t850-t868+t1046+t1300+(t12.*t84)./1.0e+1-(t48.*t128)./1.0e+1).*(-1.0./2.0);
t7480 = t7019.*(t191.*(6.0./5.0)+t305+t425+t478+t505-t781-t793-t861-t879+t1308+t12.*t84.*(3.0./1.0e+1)-t48.*t128.*(3.0./1.0e+1)).*(-1.0./2.0);
t7481 = (t7019.*(t191.*(6.0./5.0)+t305+t425+t478+t505-t781-t793-t861-t879+t1308+t12.*t84.*(3.0./1.0e+1)-t48.*t128.*(3.0./1.0e+1)))./2.0;
t7494 = (t3.*t4.*t7482)./2.0;
t7525 = (t690.*t7482)./2.0;
t7529 = (t7225.*t7362)./2.0;
t7530 = (t7224.*t7363)./2.0;
t7532 = t7213.*(t296+t369+t397+t404-t562+t728+t738-t768+t1301+t1500-(t12.*t101)./1.0e+1-(t12.*t106)./1.0e+1).*(-1.0./2.0);
t7534 = t7210.*(t191.*(2.0./5.0)+t297+t413+t463+t504-t766-t850-t868+t1046+t1300+(t12.*t84)./1.0e+1-(t48.*t128)./1.0e+1).*(-1.0./2.0);
t7535 = t7209.*(t191.*(6.0./5.0)+t305+t425+t478+t505-t781-t793-t861-t879+t1308+t12.*t84.*(3.0./1.0e+1)-t48.*t128.*(3.0./1.0e+1)).*(-1.0./2.0);
t7541 = (t7212.*(t304+t372+t405+t418-t566+t740+t748-t782+t1309+t1505-t12.*t101.*(3.0./1.0e+1)-t12.*t106.*(3.0./1.0e+1)))./2.0;
t7542 = (t7210.*(t191.*(2.0./5.0)+t297+t413+t463+t504-t766-t850-t868+t1046+t1300+(t12.*t84)./1.0e+1-(t48.*t128)./1.0e+1))./2.0;
t7575 = (t3709.*t7557)./2.0;
t7578 = (t3755.*t7564)./2.0;
t7652 = (t688.*t7600)./2.0;
t7658 = (t1250.*t7602)./2.0;
t7663 = t521+t1721+t1723+t1966+t2239+t2277+t2281+t2459+t2698+t2761+t2770+t2924+t3300+t3634+t3650+t3790;
t7672 = (t687.*t7659)./2.0;
t7678 = (t2027.*t7659)./2.0;
t7686 = (t3060.*t7659)./2.0;
t7722 = dq2.*t7721;
t7754 = (t688.*t7729)./2.0;
t7757 = (t1250.*t7727)./2.0;
t7765 = (t3709.*t7729)./2.0;
t7766 = (t3755.*t7727)./2.0;
t8002 = dq1.*t7999;
t8051 = dq1.*t8046;
t8117 = dq1.*(t1609+t1619+t2103+t2157+t2348+t2401+t2527+t2536+t2574+t2672+t2764+t2772+t2832+t3147+t3366+t3438+t3467+t3481+t3488+t3663+t3807+t3831+t3970+t4084+t4183+t4233+t4391+t4419+t4574+t4633+t4817+t5039+t5094+t5136+t5187+t5215+t5223+t5389+t5449+t5498+t5510+t5609+t5676+t5722+t5729+t5910+t6055+t6091+t6340+t11.*t3073+t9.*t20.*t2222+t11.*t112.*t2324+t9.*t13.*t3214-t7.*t9.*t13.*t20.*5.5078125e-3+t9.*t20.*t21.*t2222-t7.*t9.*t13.*t20.*t21.*5.5078125e-3);
t2971 = -t2712;
t2972 = -t2714;
t3001 = -t2722;
t4101 = -t3804;
t4102 = -t3805;
t4169 = -t3816;
t4170 = -t3818;
t4214 = -t3847;
t4215 = -t3849;
t4596 = t3.*t3891;
t4643 = t12.*t3890;
t4646 = t12.*t3892;
t4667 = t21.*t3119;
t4668 = t18.*t3124;
t4689 = -t4255;
t4701 = -t4270;
t4982 = t19.*t3424;
t5331 = t19.*t4013;
t5430 = t54.*t3893;
t5565 = t19.*t3890;
t5566 = t18.*t3891;
t5567 = t21.*t3890;
t5568 = t20.*t3891;
t5569 = t19.*t3892;
t5570 = t18.*t3893;
t5572 = t20.*t3893;
t5623 = t20.*t3917;
t5641 = t21.*t3944;
t5642 = t21.*t3945;
t5682 = t12.*t4888;
t5758 = t19.*t4436;
t5881 = t19.*t4149;
t6036 = t99.*t3917;
t6068 = t21.*t4845;
t6114 = t18.*t4537;
t6168 = t10.*t20.*t3890;
t6170 = t18.*t4645;
t6172 = t20.*t4645;
t6173 = t56.*t4846;
t6308 = t18.*t4948;
t6309 = t26.*t4888;
t6333 = t18.*t5015;
t6358 = t6.*t5970;
t6378 = t18.*t5118;
t6398 = t19.*t5148;
t6448 = t26.*t5578;
t6449 = t27.*t5576;
t6450 = t27.*t5577;
t6451 = t18.*t5632;
t6459 = -t6280;
t6462 = t18.*t5330;
t6464 = -t6286;
t6466 = -t6288;
t6479 = t19.*t5374;
t6494 = t20.*t5427;
t6497 = t25.*t5375;
t6505 = t125.*t4845;
t6517 = t18.*t5490;
t6555 = t21.*t5574;
t6576 = t10.*t20.*t4886;
t6580 = t21.*t5699;
t6586 = t10.*t20.*t4946;
t6638 = t19.*t5956;
t6647 = t19.*t5998;
t6650 = t21.*t6014;
t6651 = t20.*t6015;
t6685 = t18.*t6197;
t6701 = t3.*t19.*t5970;
t6716 = t18.*t6637;
t6726 = t1399+t3925;
t6732 = t1606+t4256;
t6773 = t1955+t5818;
t6774 = t1973+t5828;
t6777 = t690.*t6643;
t6779 = t6.*t690.*t4014.*1.0675e-2;
t6793 = -t6782;
t6794 = t3924+t4665;
t6795 = t3201+t5477;
t6798 = t3957+t5829;
t6817 = -t6804;
t6821 = t3202+t6698;
t6823 = t4014.*t6569;
t6824 = t3955+t6591;
t6839 = t3709.*t6643;
t6840 = t3755.*t6643;
t6841 = t6.*t3709.*t4014.*1.0675e-2;
t6842 = t6.*t3755.*t4014.*1.0675e-2;
t6845 = t3606+t6714;
t6849 = t4269+t6661;
t6867 = -t3026.*(t1387-t3956);
t6868 = t416+t555+t2716+t2722;
t6874 = -t6864;
t6875 = -t6720.*(t97-t1942);
t6877 = t12.*t690.*t6740.*1.35e-3;
t6878 = t4014.*t6728;
t6887 = -t6869;
t6889 = t6.*t690.*t6741.*1.0675e-2;
t6896 = (t97-t1942).*(t1387-t3956);
t6897 = -t12.*t3755.*(t1387-t3956);
t6900 = -t6882;
t6901 = -t6883;
t6904 = -t6886;
t6922 = -t6913;
t6933 = t3756.*(t1777-t5476);
t6939 = (t189-t2612).*(t1387-t3956);
t6940 = (t97-t1942).*(t1761-t5472);
t6941 = (t193-t2663).*(t1387-t3956);
t6942 = (t97-t1942).*(t1777-t5476);
t6960 = t6276.*t6740;
t6965 = -t1705.*(t3923-t6597);
t6972 = -t6950;
t6973 = -t6952;
t6974 = -t6954;
t6975 = -t6955;
t6976 = -t6956;
t6977 = t6456.*t6740;
t6983 = t6569.*t6741;
t6985 = t6570.*t6741;
t6987 = t12.*t3709.*t6740.*1.35e-3;
t6988 = t165+t299+t419+t472+t2307+t2447;
t6989 = t12.*t3755.*t6740.*1.35e-3;
t6990 = -t6717.*(t1387-t3956);
t6991 = -t6718.*(t1387-t3956);
t7000 = t6.*t3709.*t6741.*1.0675e-2;
t7001 = t6.*t3755.*t6741.*1.0675e-2;
t7012 = t6151.*t6786;
t7016 = t6100.*t6786;
t7021 = t1663.*(t3626-t6712);
t7022 = t2028.*(t3923-t6597);
t7037 = t6720.*t6740;
t7048 = t6717.*t6760;
t7049 = t6718.*t6760;
t7069 = t3026.*(t3923-t6597);
t7070 = t6728.*t6741;
t7074 = t3061.*(t3923-t6597);
t7083 = t6720.*(t1928-t4165);
t7090 = (t1387-t3956).*(t1552-t4983);
t7093 = (t1387-t3956).*(t1928-t4165);
t7094 = (t97-t1942).*(t3923-t6597);
t7095 = (t126-t1522).*(t3626-t6712);
t7097 = -t6741.*(t1592-t4271);
t7101 = t3756.*(t3242-t6692);
t7102 = -t3756.*(t3626-t6712);
t7115 = -t6.*t3755.*(t3626-t6712);
t7116 = (t1592-t4271).*(t1552-t4983);
t7117 = t12.*t3709.*(t3923-t6597);
t7119 = t6728.*(t1552-t4983);
t7130 = t6740.*t6749;
t7134 = -t6740.*(t1777-t5476);
t7136 = t6740.*t6757;
t7137 = t6740.*t6760;
t7138 = t6741.*t6760;
t7152 = (t189-t2612).*(t3923-t6597);
t7153 = (t1928-t4165).*(t1761-t5472);
t7155 = (t1928-t4165).*(t1777-t5476);
t7156 = (t193-t2663).*(t3923-t6597);
t7164 = t6740.*t6786;
t7165 = t6741.*t6786;
t7166 = t6741.*t6789;
t7167 = t6741.*t6790;
t7169 = t276+t277+t616+t6281+t6465;
t7171 = t269+t446+t562+t6282+t6458;
t7185 = -t6717.*(t3923-t6597);
t7186 = -t6718.*(t3923-t6597);
t7216 = (t1939-t2220).*(t3626-t6712);
t7217 = (t1551-t2621).*(t3626-t6712);
t7220 = t2272+t2462+t6280+t6286;
t7221 = t2274+t2463+t6283+t6288;
t7250 = -t6740.*(t3626-t6712);
t7253 = (t1552-t4983).*(t3923-t6597);
t7254 = (t1928-t4165).*(t3242-t6692);
t7256 = (t1928-t4165).*(t3923-t6597);
t7272 = (t1552-t4983).*(t3626-t6712);
t7275 = (t1928-t4165).*(t3626-t6712);
t7287 = t297+t540+t2713+t2719+t3180+t3515;
t7313 = -t7312;
t7316 = -t7314;
t7332 = t285+t286+t379+t617+t622+t859+t6284+t6467;
t7335 = -t7328;
t7341 = t293+t370+t842+t2712+t2718+t5819+t6098;
t7344 = t305+t505+t543+t1048+t2715+t2721+t3181+t3516;
t7348 = -t7347;
t7358 = -t7353;
t7407 = -t7404;
t7408 = t7402./2.0;
t7409 = -t7406;
t7411 = -t7410;
t7415 = t243+t301+t374+t410+t414+t848+t921+t2714+t2720+t5820+t6099;
t7426 = t6733+t6921+t6945;
t7441 = dq3.*t7434;
t7446 = t2.*t7019.*t7299.*(3.0./2.0);
t7447 = t8.*t7026.*t7299.*(3.0./2.0);
t7457 = t2.*t7200.*t7299.*(3.0./2.0);
t7460 = t8.*t7299.*(t208.*(2.0./5.0)-t295-t402-t736+t772+t1274+(t12.*t105)./1.0e+1-(t12.*t200)./1.0e+1).*(3.0./2.0);
t7461 = -t7459;
t7465 = -t7463;
t7471 = -t7470;
t7472 = (t7027.*t7370)./2.0;
t7473 = (t7026.*t7372)./2.0;
t7518 = (t7206.*t7370)./2.0;
t7519 = (t7205.*t7372)./2.0;
t7526 = t964+t1889+t2058+t2233+t2262+t2572+t3216+t3252+t3356+t3636+t3718+t4616;
t7537 = -t7529;
t7579 = -t7578;
t7595 = t1191+t1889+t2058+t2066+t2262+t2425+t2860+t3063+t3216+t3252+t3356+t3444+t3636+t4616;
t7654 = t5454+t6721+t6814+t6827+t6876+t6881;
t7655 = -t7652;
t7660 = -t7658;
t7673 = (t1251.*t7663)./2.0;
t7675 = (t1662.*t7663)./2.0;
t7687 = -t7686;
t7690 = (t3754.*t7663)./2.0;
t7756 = -t7754;
t7769 = -t7766;
t7793 = t1169+t1869+t2150+t2222+t2342+t2652+t2849+t2997+t3090+t3375+t3541+t3555+t3579+t3871+t4012+t4161+t4378+t4436+t5016;
t8050 = t954+t1410+t1861+t2040+t2191+t2214+t2258+t2372+t2385+t2617+t2646+t2680+t2816+t2916+t3076+t3189+t3288+t3352+t3374+t3615+t3827+t3869+t3915+t4259+t4312+t4372+t4396+t4400+t4558+t4717+t4825+t4926+t4931+t5167+t5395+t5451+t5914;
t8090 = t1164+t1653+t1861+t2040+t2191+t2258+t2385+t2396+t2416+t2646+t2680+t2915+t2916+t3028+t3189+t3288+t3352+t3437+t3466+t3615+t3732+t3827+t3869+t3915+t4028+t4259+t4312+t4372+t4396+t4400+t4445+t4497+t4558+t4717+t4926+t4931+t5167+t5395+t5451+t5914;
t8126 = t1609+t1803+t2103+t2169+t2181+t2336+t2501+t2515+t2574+t2600+t2783+t2789+t2793+t2942+t3108+t3121+t3154+t3414+t3467+t3499+t3576+t3763+t3878+t4122+t4127+t4151+t4186+t4206+t4279+t4318+t4338+t4402+t4422+t4440+t4544+t4585+t4628+t4706+t4723+t4732+t4806+t4943+t5009+t5052+t5083+t5111+t5154+t5196+t5245+t5325+t5554+t5594+t5611+t5750+t5796+t5993+t6028+t6159+t6503;
t8129 = t162+t184+t188+t328+t333+t342+t345+t348+t515+t611+t645+t656+t675+t761+t896+t951+t965+t996+t1156+t1224+t1354+t1512+t2092+t2121+t2149+t2370+t2465+t2506+t2564+t2599+t2749+t2840+t2882+t3015+t3054+t3089+t3123+t3318+t3372+t3380+t3452+t3453+t3536+t3537+t3561+t3582+t3765+t3768+t3823+t3995+t4041+t4077+t4136+t4153+t4251+t4300+t4342+t4433+t4498+t4599+t4642+t4660+t4881+t5003+t5045+t5090+t5114+t5387+t5431+t5562+t5812+t5855+t6351;
t8130 = t256+t388+t508+t835+t892+t903+t932+t952+t977+t1029+t1070+t1091+t1119+t1134+t1155+t1202+t1297+t1558+t1560+t1831+t2030+t2310+t2567+t2618+t2675+t2736+t2766+t2827+t2867+t2962+t3069+t3097+t3188+t3304+t3358+t3401+t3459+t3528+t3622+t3660+t3696+t3713+t3851+t4194+t4288+t4296+t4394+t4414+t4482+t4563+t4580+t4598+t4602+t4821+t4827+t4867+t4928+t4938+t4975+t5076+t5089+t5139+t5236+t5383+t5432+t5542+t5813+t5945+t6045+t6273;
t8184 = t1610+t1611+t1991+t2158+t2159+t2252+t2349+t2350+t2542+t2575+t2576+t2673+t2834+t2855+t2944+t3035+t3112+t3146+t3148+t3164+t3282+t3339+t3367+t3487+t3489+t3564+t3569+t3642+t3743+t3832+t3833+t3927+t3960+t3971+t4065+t4234+t4235+t4274+t4392+t4421+t4516+t4576+t4626+t4666+t4714+t4800+t4808+t4916+t5006+t5007+t5068+t5132+t5137+t5186+t5188+t5216+t5218+t5361+t5391+t5509+t5511+t5538+t5548+t5606+t5650+t5653+t5662+t5713+t5717+t5723+t5727+t5731+t5792+t5857+t5912+t6023+t6059+t6090+t6108+t6155+t6304+t6318+t6341+t6399+t6498+t6623;
t8202 = t1789+t1790+t2123+t2158+t2159+t2252+t2349+t2350+t2542+t2595+t2673+t2855+t2872+t2894+t2895+t2944+t3146+t3148+t3164+t3282+t3339+t3482+t3487+t3489+t3564+t3569+t3642+t3760+t3832+t3833+t3927+t3960+t3971+t3999+t4002+t4053+t4065+t4234+t4235+t4274+t4392+t4487+t4516+t4576+t4626+t4666+t4760+t4800+t4808+t4842+t4865+t4916+t5006+t5007+t5068+t5132+t5137+t5186+t5188+t5216+t5218+t5251+t5283+t5361+t5391+t5509+t5511+t5538+t5548+t5650+t5653+t5662+t5713+t5717+t5723+t5727+t5731+t5792+t5857+t5912+t6023+t6059+t6090+t6108+t6155+t6304+t6318+t6341+t6399+t6498+t6623;
t6142 = t20.*t4596;
t6169 = t19.*t4643;
t6175 = t19.*t4646;
t6176 = t6.*t5623;
t6319 = t18.*t4982;
t6546 = t20.*t5565;
t6547 = t20.*t5566;
t6548 = t18.*t5569;
t6588 = t18.*t5758;
t6589 = t26.*t5682;
t6614 = t18.*t5881;
t6673 = t20.*t6170;
t6674 = t18.*t6173;
t6682 = t10.*t27.*t5567;
t6690 = t18.*t6398;
t6710 = t19.*t20.*t5570;
t6792 = -t6777;
t6797 = t4701+t5051;
t6810 = t6.*t690.*t6732;
t6822 = t1663.*t6732;
t6859 = t4689+t6663;
t6890 = t4014.*t6732;
t6891 = -t6732.*(t126-t1522);
t6908 = t6.*t3709.*t6732;
t6909 = t6.*t3755.*t6732;
t6924 = t3710.*t6774;
t6928 = t6100.*t6732;
t6929 = t4014.*t6773;
t6930 = t3710.*t6773;
t6931 = t6151.*t6732;
t6932 = t4014.*t6774;
t6934 = t12.*t690.*t6821;
t6959 = t1705.*t6821;
t6961 = t6.*t690.*t6849;
t6978 = t3756.*t6794;
t6979 = t3756.*t6795;
t6981 = t2028.*t6821;
t6982 = t1663.*t6849;
t6984 = t1664.*t6849;
t7002 = -t6794.*(t97-t1942);
t7003 = -t6795.*(t97-t1942);
t7013 = -t7000;
t7018 = t4014.*t6798;
t7025 = t3710.*t6798;
t7029 = t137+t281+t380+t416+t2716+t3001;
t7033 = -t6732.*(t1939-t2220);
t7034 = -t6732.*(t1551-t2621);
t7036 = t3026.*t6821;
t7039 = t3061.*t6821;
t7054 = t6726.*t6740;
t7056 = -t7037;
t7057 = t3710.*t6821;
t7059 = t3756.*t6821;
t7060 = t3756.*t6824;
t7075 = t12.*t3709.*t6821;
t7077 = t6732.*t6740;
t7078 = t12.*t3755.*t6821;
t7080 = t6732.*t6741;
t7081 = t4014.*t6849;
t7082 = t3710.*t6845;
t7086 = t3710.*t6849;
t7088 = t3756.*t6849;
t7089 = t3757.*t6849;
t7100 = -t7070;
t7105 = t6.*t3709.*t6849;
t7108 = t6.*t3755.*t6849;
t7109 = -t6732.*(t1928-t4165);
t7111 = t6849.*(t126-t1522);
t7118 = -t7095;
t7124 = t3755.*t6868;
t7131 = t3709.*t6868;
t7135 = -t7116;
t7143 = t6100.*t6849;
t7144 = t6741.*t6773;
t7146 = t6741.*t6774;
t7147 = t6151.*t6849;
t7163 = -t6774.*(t1552-t4983);
t7173 = -t7164;
t7178 = -t7167;
t7179 = t292+t539+t706+t721+t3801+t4101;
t7180 = t6740.*t6794;
t7181 = t6740.*t6795;
t7182 = t6717.*t6821;
t7183 = t6718.*t6821;
t7184 = t234+t548+t724+t776+t3815+t4214;
t7193 = -t6794.*(t1928-t4165);
t7194 = -t6795.*(t1928-t4165);
t7199 = t6741.*t6798;
t7207 = -t6849.*(t1939-t2220);
t7208 = -t6849.*(t1551-t2621);
t7222 = t2718+t2971+t5819+t5826;
t7223 = t2720+t2972+t5820+t5827;
t7226 = t6740.*t6821;
t7227 = t6740.*t6824;
t7228 = t6741.*t6821;
t7231 = t6798.*(t1552-t4983);
t7232 = -t7217;
t7233 = t3709.*t6988;
t7235 = t3755.*t6988;
t7243 = t6740.*t6849;
t7244 = t6741.*t6845;
t7246 = t6741.*t6849;
t7263 = -t6845.*(t1552-t4983);
t7267 = -t6849.*(t1928-t4165);
t7276 = -t7256;
t7278 = t690.*t7169;
t7281 = t690.*t7171;
t7285 = -t7275;
t7291 = t278+t764+t2271+t2303+t3848+t4169;
t7306 = t690.*t7220;
t7317 = t690.*t7287;
t7331 = t375+t618+t849+t7169;
t7336 = t242+t300+t407+t542+t708+t731+t1047+t3802+t4102;
t7337 = t237+t259+t465+t553+t737+t795+t1103+t3817+t4215;
t7340 = t393+t395+t547+t2272+t2304+t6286+t6459;
t7342 = t504+t1043+t7287;
t7345 = t287+t625+t771+t858+t2273+t2305+t3850+t4170;
t7349 = t4.*t49.*t7341;
t7373 = t690.*t7341;
t7384 = t1252.*t7341;
t7385 = t1253.*t7341;
t7414 = t168+t400+t401+t919+t7341;
t7416 = t159+t274+t279+t373+t620+t763+t844+t2445+t2462+t6280+t6464;
t7419 = t227+t283+t288+t376+t626+t767+t854+t2446+t2463+t6283+t6466;
t7431 = t3.*t7426;
t7432 = t9.*t7426;
t7443 = t4.*t49.*t7426;
t7449 = -t7446;
t7450 = t690.*t7426;
t7451 = t1252.*t7426;
t7452 = t1253.*t7426;
t7477 = -t7472;
t7500 = -t9.*(-t6799+t7137+t6786.*(t1552-t4983));
t7505 = t3.*(-t6799+t7137+t6786.*(t1552-t4983));
t7507 = t1661.*(-t6799+t6740.*(t1387-t3956)+t6732.*(t1552-t4983)).*(-1.0./2.0);
t7511 = t9.*(t6813+t7165+t6760.*(t1928-t4165));
t7513 = (t1662.*(-t6799+t6740.*(t1387-t3956)+t6732.*(t1552-t4983)))./2.0;
t7516 = t3.*t10.*(t6813+t7165+t6760.*(t1928-t4165));
t7524 = -t7518;
t7536 = t4.*t49.*(t6813+t7165+t6760.*(t1928-t4165));
t7547 = t1661.*(-t6862+t6821.*(t97-t1942)+t4014.*(t3626-t6712)).*(-1.0./2.0);
t7549 = t3754.*(-t6799+t6740.*(t1387-t3956)+t6732.*(t1552-t4983)).*(-1.0./2.0);
t7550 = (t1662.*(-t6862+t6821.*(t97-t1942)+t4014.*(t3626-t6712)))./2.0;
t7554 = -t690.*(-t6799+t7137+t6786.*(t1552-t4983));
t7555 = -t690.*(t6813+t7165+t6760.*(t1928-t4165));
t7559 = -t1253.*(-t6799+t7137+t6786.*(t1552-t4983));
t7566 = t1253.*(t6813+t7165+t6760.*(t1928-t4165));
t7571 = t3754.*(-t6862+t6821.*(t97-t1942)+t4014.*(t3626-t6712)).*(-1.0./2.0);
t7589 = -t2.*t3.*(t6949+t6821.*(t1928-t4165)+t6741.*(t3626-t6712));
t7590 = -t2.*t9.*(t6949+t6821.*(t1928-t4165)+t6741.*(t3626-t6712));
t7594 = -t8.*t9.*(t6947+t6849.*(t1552-t4983)+t6740.*(t3923-t6597));
t7596 = -t3.*t48.*(t6949+t6821.*(t1928-t4165)+t6741.*(t3626-t6712));
t7597 = -t3.*t53.*(t6947+t6849.*(t1552-t4983)+t6740.*(t3923-t6597));
t7598 = t3.*t8.*(t6949+t6821.*(t1928-t4165)+t6741.*(t3626-t6712));
t7599 = dq3.*t7595;
t7601 = t6919+t6920+t6972+t6973;
t7607 = -t687.*(t6947+t6849.*(t1552-t4983)+t6740.*(t3923-t6597));
t7608 = -t688.*(t6947+t6849.*(t1552-t4983)+t6740.*(t3923-t6597));
t7620 = -t1250.*(t6949+t6821.*(t1928-t4165)+t6741.*(t3626-t6712));
t7621 = -t1251.*(t6949+t6821.*(t1928-t4165)+t6741.*(t3626-t6712));
t7634 = -t1703.*(t6947+t6849.*(t1552-t4983)+t6740.*(t3923-t6597));
t7636 = t1662.*(t6949+t6821.*(t1928-t4165)+t6741.*(t3626-t6712));
t7644 = -t3060.*(t6947+t6849.*(t1552-t4983)+t6740.*(t3923-t6597));
t7649 = -t3754.*(t6949+t6821.*(t1928-t4165)+t6741.*(t3626-t6712));
t7651 = -t3755.*(t6949+t6821.*(t1928-t4165)+t6741.*(t3626-t6712));
t7656 = t3709.*(t6949+t6821.*(t1928-t4165)+t6741.*(t3626-t6712));
t7657 = t3755.*(t6947+t6849.*(t1552-t4983)+t6740.*(t3923-t6597));
t7661 = t9.*t7654;
t7664 = t3.*t4.*t7654;
t7667 = t690.*t7654;
t7674 = t6739+t6747+t6811+t6851+t6865+t6900;
t7735 = t6738+t6746+t6922+t6926+t6951+t6953;
t7751 = -t690.*(t7138-t7166+t7176+t6757.*(t1928-t4165));
t7788 = -t3.*t4.*(t6796-t6808-t6936+t6967-t6985+t6276.*(t1928-t4165));
t7790 = t9.*(t6796-t6808-t6936+t6967-t6985+t6276.*(t1928-t4165));
t7795 = t9.*(t6725+t6783+t6977+t7035-t7048+t7122);
t7802 = dq3.*t7793;
t7807 = t3.*t4.*(t6727+t6793+t6983+t7023-t7049+t7123);
t7810 = t3.*t4.*(t6800+t6805+t6935-t6960-t6966+t6570.*(t1552-t4983));
t7825 = -t690.*(t6725+t6783+t6977+t7035-t7048+t7122);
t7827 = t690.*(t6796-t6808-t6936+t6967-t6985+t6276.*(t1928-t4165));
t7833 = -t690.*(t6727+t6793+t6983+t7023-t7049+t7123);
t7872 = t9.*(t6766+t6817+t7016-t7130+t6760.*(t189-t2612)+t6790.*(t1552-t4983));
t7877 = t3.*t4.*(t6766+t6817+t7016-t7130+t6760.*(t189-t2612)+t6790.*(t1552-t4983));
t7904 = -t2.*t3.*(-t6825-t6879+t6821.*(t189-t2612)+t6773.*(t1552-t4983)+t6740.*(t1761-t5472)+t6100.*(t3626-t6712));
t7914 = t688.*(-t6825-t6879+t6821.*(t189-t2612)+t6773.*(t1552-t4983)+t6740.*(t1761-t5472)+t6100.*(t3626-t6712));
t7924 = -t3709.*(-t6825-t6879+t6821.*(t189-t2612)+t6773.*(t1552-t4983)+t6740.*(t1761-t5472)+t6100.*(t3626-t6712));
t7961 = -t2.*t3.*(t6947+t6949+t6821.*(t1928-t4165)+t6849.*(t1552-t4983)+t6741.*(t3626-t6712)+t6740.*(t3923-t6597));
t7962 = -t3.*t8.*(t6947+t6949+t6821.*(t1928-t4165)+t6849.*(t1552-t4983)+t6741.*(t3626-t6712)+t6740.*(t3923-t6597));
t7971 = t1250.*(t6947+t6949+t6821.*(t1928-t4165)+t6849.*(t1552-t4983)+t6741.*(t3626-t6712)+t6740.*(t3923-t6597));
t7976 = -t3709.*(t6947+t6949+t6821.*(t1928-t4165)+t6849.*(t1552-t4983)+t6741.*(t3626-t6712)+t6740.*(t3923-t6597));
t7983 = t3755.*(t6947+t6949+t6821.*(t1928-t4165)+t6849.*(t1552-t4983)+t6741.*(t3626-t6712)+t6740.*(t3923-t6597));
t8052 = dq2.*t8050;
t8096 = t1867+t2500+t2650+t2782+t2865+t2929+t2995+t3096+t3124+t3385+t3501+t3509+t3865+t3951+t4017+t4126+t4133+t4174+t4376+t4613+t4627+t4730+t4771+t4864+t4948+t5115+t5119+t5195+t5330+t5448+t5503+t5556+t5593+t5638+t5706+t5758+t5788+t5892+t6334+t7396;
t8182 = t534+t597+t643+t679+t699+t823+t975+t987+t991+t1187+t1233+t1240+t1246+t1289+t1296+t1363+t1458+t1554+t1689+t1822+t1864+t1935+t2063+t2378+t2382+t2509+t2643+t2786+t2926+t2986+t2989+t3102+t3153+t3204+t3205+t3246+t3473+t3494+t3521+t3571+t3573+t3686+t3828+t3910+t3947+t4139+t4156+t4209+t4242+t4364+t4366+t4451+t4531+t4537+t4632+t4664+t4750+t4767+t4769+t4854+t4908+t4933+t5012+t5015+t5058+t5118+t5140+t5194+t5202+t5396+t5471+t5484+t5531+t5563+t5568+t5597+t5618+t5632+t5673+t5702+t5780+t5928+t5968+t6148+t6172+t6190+t6197+t6359+t6397+t6636+t6743;
t8206 = dq1.*t8202;
t8231 = t177+t343+t347+t433+t502+t561+t937+t978+t990+t1069+t1071+t1097+t1126+t1151+t1152+t1206+t1290+t1298+t1324+t1356+t1391+t1396+t1413+t1421+t1463+t1482+t1559+t1594+t1693+t1763+t1895+t1907+t1925+t2436+t2449+t2470+t2472+t2475+t2498+t2667+t2674+t3034+t3064+t3094+t3185+t3233+t3253+t3274+t3362+t3455+t3632+t3649+t3695+t3699+t3723+t3724+t3758+t3786+t3917+t3988+t4015+t4042+t4064+t4113+t4116+t4171+t4191+t4197+t4386+t4393+t4438+t4483+t4555+t4567+t4713+t4719+t4761+t4862+t4906+t4927+t5000+t5126+t5135+t5138+t5173+t5281+t5305+t5333+t5336+t5386+t5400+t5428+t5458+t5468+t5502+t5540+t5649+t5660+t5785+t5853+t5867+t5970+t5986+t6049+t6068+t6077+t6165+t6315+t6605+t6735;
t8232 = t601+t899+t941+t1160+t1192+t1214+t1288+t1328+t1353+t1362+t1414+t1428+t1431+t1461+t1580+t1677+t1682+t1688+t1698+t1718+t1795+t1817+t1843+t1858+t1897+t1912+t1934+t2005+t2021+t2025+t2037+t2050+t2135+t2410+t2581+t2656+t2658+t2711+t2902+t2950+t3003+t3211+t3218+t3322+t3347+t3427+t3493+t3512+t3611+t3643+t3654+t3771+t3886+t3895+t3954+t3966+t4082+t4120+t4213+t4257+t4283+t4326+t4458+t4534+t4651+t4746+t4779+t4781+t4783+t4853+t4870+t4874+t4884+t4923+t5022+t5033+t5102+t5165+t5297+t5299+t5324+t5362+t5363+t5409+t5414+t5415+t5444+t5483+t5491+t5530+t5574+t5596+t5677+t5680+t5718+t5748+t5779+t5789+t5838+t5898+t5960+t5972+t5984+t6011+t6050+t6057+t6123+t6137+t6181+t6189+t6206+t6249+t6260+t6271+t6322+t6343+t6367+t6387+t6406+t6439+t6444+t6450+t6468+t6472+t6474+t6504+t6559+t6601+t6641+t6652+t6654;
t8239 = t314+t491+t559+t601+t602+t662+t666+t909+t941+t970+t1116+t1124+t1148+t1217+t1353+t1438+t1448+t1455+t1510+t1575+t1582+t1636+t1655+t1665+t1668+t1700+t1709+t1728+t1766+t1830+t1849+t1852+t1893+t1992+t2010+t2020+t2025+t2037+t2080+t2139+t2204+t2357+t2381+t2454+t2607+t2658+t2691+t2702+t2755+t2800+t2837+t2873+t2902+t2937+t2969+t2984+t3009+t3133+t3218+t3245+t3281+t3306+t3315+t3347+t3427+t3456+t3611+t3631+t3673+t3688+t3742+t3749+t3810+t3811+t3846+t3895+t3928+t3976+t4003+t4022+t4058+t4087+t4240+t4268+t4275+t4326+t4328+t4424+t4463+t4470+t4488+t4513+t4543+t4561+t4572+t4593+t4622+t4651+t4783+t4835+t4837+t4911+t4913+t4968+t4976+t4978+t4991+t4998+t5024+t5027+t5077+t5129+t5165+t5222+t5227+t5264+t5274+t5276+t5285+t5338+t5339+t5370+t5456+t5496+t5605+t5625+t5654+t5728+t5744+t5752+t5802+t5825+t5844+t5849+t5877+t5939+t5958+t5960+t5994+t5997+t6024+t6031+t6053+t6065+t6075+t6084+t6085+t6118+t6121+t6200+t6210+t6232+t6239+t6247+t6279+t6290+t6295+t6301+t6345+t6362+t6371+t6431+t6453+t6479+t6489+t6536+t6555+t6566+t6584+t6694;
t6676 = t18.*t6175;
t6707 = t21.*t6546;
t7017 = t4014.*t6797;
t7024 = t3710.*t6797;
t7055 = -t7036;
t7104 = t3710.*t6859;
t7107 = -t7077;
t7110 = -t7082;
t7113 = -t7089;
t7125 = -t7105;
t7132 = t7124.*3.0;
t7141 = t7131.*3.0;
t7188 = t1661.*t7029;
t7189 = t1662.*t7029;
t7190 = t1703.*t7029;
t7191 = -t7181;
t7192 = -t7183;
t7198 = t6741.*t6797;
t7203 = t2027.*t7029;
t7238 = t3060.*t7029;
t7239 = t7233.*3.0;
t7241 = t7235.*3.0;
t7251 = -t7235;
t7257 = t6741.*t6859;
t7258 = t3709.*t7029;
t7259 = t3754.*t7029;
t7260 = t3755.*t7029;
t7265 = -t7243;
t7266 = -t7244;
t7268 = -t7246;
t7282 = t7278.*3.0;
t7283 = t690.*t7179;
t7284 = t6859.*(t1552-t4983);
t7288 = t7281.*3.0;
t7289 = t690.*t7184;
t7292 = -t7281;
t7308 = t690.*t7222;
t7309 = t7306.*3.0;
t7318 = t690.*t7291;
t7319 = t7317.*3.0;
t7320 = -t7317;
t7330 = t167+t399+t1042+t7179;
t7333 = t179+t453+t1100+t7184;
t7343 = t619+t847+t7291;
tau = ft_13({dq1,dq2,dq3,dq4,dq5,dq6,t10,t1001,t1002,t1003,t1004,t1005,t1006,t1007,t1009,t101,t1010,t1023,t1024,t1025,t1026,t1027,t1030,t1032,t1033,t1034,t1035,t1037,t1038,t1039,t1041,t1046,t105,t1053,t106,t1063,t1068,t107,t1073,t1074,t1075,t1076,t1077,t1078,t1079,t108,t1080,t1081,t1083,t1084,t1086,t1087,t1089,t109,t1090,t1092,t1095,t1096,t1097,t1098,t11,t110,t111,t1115,t1117,t1118,t112,t1120,t1122,t1123,t1127,t1128,t1129,t113,t1130,t1131,t1132,t1133,t114,t1149,t1150,t1153,t1156,t1157,t1158,t1159,t1162,t1163,t1166,t1170,t1171,t1172,t1173,t1174,t1179,t1180,t1182,t1183,t1186,t1188,t1189,t1193,t1194,t1195,t1196,t1198,t1199,t12,t1201,t1203,t1204,t1205,t1207,t1208,t1210,t1211,t1212,t1215,t1218,t1219,t1220,t1221,t1222,t1227,t1228,t1229,t123,t1230,t1231,t1234,t1235,t1239,t124,t1241,t1242,t1243,t1244,t1245,t1247,t125,t1250,t1251,t1252,t1253,t1254,t1256,t126,t1263,t1266,t127,t1274,t128,t1284,t1285,t1287,t129,t1291,t1293,t1295,t1298,t1299,t13,t130,t1300,t1301,t1308,t1309,t1313,t1317,t1318,t1319,t1320,t1323,t1325,t1326,t1327,t1329,t1331,t1332,t1333,t1334,t1339,t1343,t1344,t1345,t1346,t1347,t1349,t1351,t1352,t1354,t1357,t1358,t1359,t1360,t1361,t1364,t1365,t1366,t1368,t1369,t1371,t1373,t1375,t1376,t1377,t1378,t1379,t1380,t1383,t1385,t1386,t1387,t1388,t1389,t1390,t1392,t1393,t1394,t1395,t1397,t1398,t140,t1405,t1406,t141,t1411,t1412,t1415,t1416,t1417,t1419,t1420,t1422,t1423,t1424,t1426,t1427,t1429,t143,t1430,t1432,t1433,t1434,t1435,t1439,t1440,t1441,t1442,t1443,t1445,t1446,t1450,t1452,t1453,t1456,t1457,t1459,t1460,t1462,t1464,t1465,t1466,t1467,t1468,t1469,t1470,t1473,t1477,t1479,t1480,t1481,t1482,t1484,t1488,t1490,t1491,t1492,t1493,t1494,t1495,t1496,t1500,t1505,t1507,t1508,t1511,t1513,t1516,t1517,t1518,t1519,t1522,t1523,t1524,t1525,t1526,t1528,t1541,t1542,t1543,t1545,t1546,t1547,t1548,t1549,t1552,t1553,t1555,t1556,t1557,t1571,t1572,t1573,t1576,t1577,t1578,t1579,t1581,t1583,t1584,t1585,t1586,t1587,t1592,t1594,t1595,t1596,t1609,t1613,t1615,t1619,t1620,t163,t1637,t1639,t164,t1641,t1642,t1643,t1644,t1645,t1646,t1656,t1659,t166,t1660,t1661,t1662,t1663,t1664,t1666,t1669,t1670,t1671,t1672,t1673,t1675,t1676,t1678,t1679,t1680,t1681,t1684,t1685,t1686,t1687,t1690,t1691,t1692,t1694,t1696,t1697,t1701,t1702,t1703,t1706,t1707,t1710,t1711,t1713,t1716,t1717,t1719,t1720,t1726,t1727,t1730,t1732,t1735,t1739,t1744,t1745,t1749,t1750,t1751,t1752,t1753,t1754,t1755,t1756,t1758,t1759,t1760,t1761,t1762,t1763,t1764,t1768,t1771,t1772,t1773,t1776,t1778,t1779,t178,t1785,t1787,t1796,t1799,t18,t1800,t1801,t1803,t1804,t1806,t1815,t1816,t1818,t1819,t182,t1820,t1821,t1823,t1824,t1825,t1826,t1827,t1828,t1829,t183,t1832,t1833,t1835,t1836,t1837,t1839,t1840,t1841,t1842,t1844,t1845,t1847,t1848,t185,t1850,t1851,t1853,t1854,t1856,t1857,t186,t1860,t1865,t1866,t1868,t1869,t187,t1874,t1876,t1877,t1878,t1879,t1882,t1883,t189,t1895,t1896,t1898,t1899,t19,t1900,t1901,t1902,t1903,t1904,t1905,t1906,t1908,t1909,t191,t1911,t1913,t1914,t1917,t1919,t1920,t1921,t1922,t1925,t1926,t1928,t193,t1930,t1931,t1933,t1936,t1937,t194,t1942,t1943,t1944,t1947,t1949,t195,t1958,t1959,t1962,t1964,t1993,t1994,t1995,t1996,t1997,t1998,t2,t20,t200,t2000,t2001,t2002,t2003,t2004,t2006,t2009,t2012,t2013,t2014,t2015,t2016,t2017,t2018,t202,t2023,t2024,t2027,t2028,t2029,t203,t2034,t2036,t2038,t2039,t204,t2043,t2044,t2045,t2053,t2054,t2055,t2056,t2059,t2061,t2067,t2068,t2069,t2072,t2074,t2075,t2078,t2079,t208,t2083,t2084,t2085,t2086,t2087,t2088,t2089,t2090,t2094,t2096,t2097,t21,t210,t2103,t2107,t2109,t211,t2110,t2111,t2112,t2115,t2116,t2117,t2118,t212,t2120,t2124,t2125,t2126,t2127,t2129,t2132,t2133,t2134,t2136,t2138,t214,t2140,t2141,t2147,t2148,t215,t2151,t2152,t2157,t216,t2161,t2168,t2171,t2178,t2179,t2185,t2193,t22,t2200,t2201,t2202,t2203,t2205,t2206,t2207,t2208,t2212,t2216,t2217,t2219,t2221,t2222,t2223,t2224,t2225,t2227,t2228,t2229,t2231,t2234,t2235,t2236,t2237,t2238,t224,t2245,t2246,t2247,t2248,t2250,t2254,t2259,t2276,t228,t2280,t2283,t2284,t2285,t2287,t229,t2290,t2292,t2293,t2295,t230,t2308,t231,t2314,t2318,t2319,t2320,t2322,t2323,t2324,t2325,t2326,t2327,t2343,t2347,t2348,t2353,t2358,t2362,t2363,t2364,t2373,t2375,t2379,t2383,t2387,t2394,t2395,t2397,t2398,t2400,t2401,t2403,t2404,t2405,t2409,t2411,t2412,t2413,t2414,t2415,t2417,t2419,t2421,t2422,t2423,t2426,t2430,t2431,t2432,t2433,t2437,t2438,t2439,t244,t2440,t245,t2450,t2451,t2452,t2453,t2455,t2456,t2457,t246,t2464,t2466,t2467,t2469,t247,t2471,t2472,t2473,t2474,t2477,t2478,t2479,t248,t2480,t2481,t2482,t2483,t2484,t2485,t2486,t2487,t2488,t249,t2491,t2499,t250,t2504,t2507,t2508,t251,t252,t2524,t2525,t2527,t2529,t253,t2531,t2536,t2543,t2546,t255,t2551,t2552,t2553,t2555,t2559,t2560,t2565,t2566,t2568,t2569,t2571,t2574,t2578,t2580,t2582,t2583,t2585,t2586,t2588,t2591,t2593,t2594,t2598,t260,t2601,t2603,t2604,t2605,t2608,t2609,t261,t2610,t2611,t2612,t2614,t2615,t262,t2622,t2625,t2628,t2629,t263,t2632,t2634,t2641,t2644,t2645,t2648,t2649,t265,t2651,t2655,t2657,t2659,t2660,t2661,t2662,t2663,t267,t2672,t2679,t2692,t2694,t2695,t2700,t2701,t2703,t2705,t2725,t2726,t2727,t2729,t2730,t2732,t2733,t2734,t2735,t2738,t2739,t2740,t2741,t2743,t2747,t2748,t2752,t2753,t2756,t2760,t2763,t2764,t2765,t2767,t2769,t2772,t2784,t2785,t2792,t2794,t2795,t2796,t28,t2801,t2803,t2804,t2806,t2809,t2811,t2812,t2813,t2815,t2817,t2819,t2820,t2821,t2822,t2825,t2828,t2829,t2830,t2832,t2833,t2836,t2839,t2843,t2844,t2848,t2850,t2852,t2854,t2856,t2861,t2862,t2863,t2864,t2866,t2869,t2877,t2878,t2880,t2887,t2888,t2890,t2892,t2899,t29,t2900,t2901,t2903,t2904,t2905,t2906,t2910,t2911,t2912,t2917,t2919,t2921,t2922,t2923,t2925,t2927,t2928,t2931,t2932,t2933,t2934,t2938,t2939,t2940,t2943,t2949,t295,t2951,t2952,t2953,t2954,t2956,t2957,t2959,t296,t2960,t2964,t2965,t2968,t297,t2970,t2973,t2975,t2977,t298,t2981,t2988,t2990,t2991,t2992,t2993,t2996,t3,t3002,t3004,t3006,t3007,t3008,t3010,t3011,t3012,t3013,t3016,t3018,t3019,t3025,t3026,t303,t3030,t3033,t3037,t3039,t304,t3040,t3043,t3045,t3046,t3047,t3049,t305,t3050,t3056,t3058,t3059,t3060,t3065,t3066,t3067,t3068,t3070,t3071,t3072,t3073,t3074,t3075,t3077,t3078,t3079,t308,t3085,t3087,t3088,t309,t3091,t3092,t3095,t3098,t3099,t3100,t3101,t3104,t3106,t3109,t311,t3110,t3111,t3119,t312,t3125,t3129,t313,t3130,t3131,t3136,t3138,t3139,t3144,t3147,t3149,t3150,t3152,t3159,t3170,t3173,t3174,t3177,t3186,t3187,t3192,t3193,t3194,t3195,t3198,t3200,t3203,t3206,t3207,t3208,t3209,t3210,t3211,t3212,t3213,t3214,t3215,t3217,t3219,t3220,t3222,t3223,t3224,t3225,t3226,t3227,t3228,t3231,t3232,t3233,t3234,t3235,t3236,t3237,t3238,t3239,t3242,t3247,t3249,t3250,t3253,t3254,t3255,t3256,t3258,t3260,t3262,t3265,t3269,t3270,t3271,t3273,t3274,t3275,t3280,t3283,t3284,t3286,t3287,t329,t3296,t3297,t3298,t330,t3303,t3305,t3307,t3308,t331,t3316,t332,t3323,t3324,t3326,t3327,t3328,t3329,t3330,t3331,t3332,t3333,t3334,t3335,t3336,t334,t3342,t3345,t3346,t3348,t3353,t3359,t336,t3361,t3363,t3364,t3365,t3366,t337,t3377,t3378,t3379,t338,t3384,t3386,t3387,t339,t3394,t3395,t3396,t3397,t3399,t3402,t3405,t341,t3410,t3411,t3412,t3413,t3416,t3419,t342,t3421,t3422,t3424,t3425,t3426,t3430,t3435,t3436,t3438,t3439,t344,t3440,t3442,t3443,t3444,t3445,t3446,t3449,t3454,t3458,t346,t3463,t3467,t3470,t3471,t3472,t3474,t3475,t3476,t3477,t348,t3480,t3481,t3483,t3484,t3485,t3488,t349,t3491,t3492,t3496,t3498,t350,t3502,t3504,t3506,t3507,t3508,t3511,t3513,t3519,t352,t3520,t3522,t3523,t3526,t3527,t3529,t353,t3531,t3532,t3533,t3535,t3538,t354,t3542,t3543,t3544,t3545,t3548,t3549,t355,t3552,t3553,t3554,t3559,t356,t3565,t3566,t3567,t3568,t357,t3575,t3578,t358,t3586,t3587,t3588,t3590,t3591,t3592,t3593,t3596,t3598,t3599,t360,t3600,t3601,t3602,t3603,t3604,t3608,t3609,t3610,t3612,t3613,t3614,t3617,t3620,t3621,t3623,t3626,t3627,t3628,t3629,t3630,t3633,t3638,t3639,t3640,t3641,t3645,t3646,t3648,t3652,t3653,t3655,t3656,t3657,t3658,t3663,t3667,t3668,t3670,t3671,t3674,t3675,t3676,t3677,t3679,t3680,t3681,t3682,t3683,t3684,t3687,t3689,t369,t3690,t3691,t3692,t3694,t3697,t3698,t370,t3700,t3701,t3702,t3703,t3704,t3705,t3708,t3709,t3710,t3711,t3712,t3713,t3714,t3715,t3717,t3719,t372,t3720,t3721,t3722,t3725,t3726,t3727,t3728,t3729,t3730,t3733,t3734,t3735,t3736,t3737,t3738,t3739,t374,t3740,t3741,t3744,t3745,t3747,t3748,t3750,t3751,t3752,t3754,t3755,t3756,t3757,t3759,t3764,t3766,t3767,t3769,t3770,t3772,t3774,t3775,t3776,t3777,t3778,t3780,t3781,t3782,t3785,t3787,t3789,t3792,t3793,t3794,t3796,t3798,t3806,t3807,t3808,t3809,t3812,t3813,t3814,t3820,t3821,t3822,t3824,t3825,t3826,t3829,t3831,t3837,t3838,t3839,t384,t3840,t3841,t3852,t3854,t3856,t3857,t386,t3860,t3861,t3862,t3863,t3864,t3868,t387,t3872,t3874,t3875,t3876,t3882,t3884,t3885,t3887,t3888,t3889,t389,t3892,t3894,t3896,t3897,t3898,t3899,t3900,t3901,t3902,t3903,t3904,t3906,t3908,t3909,t3912,t3913,t3916,t3918,t3919,t3920,t3921,t3922,t3923,t3926,t3930,t3931,t3932,t3935,t3936,t3939,t3941,t3944,t3945,t3946,t3948,t3949,t3950,t3953,t3956,t3959,t3964,t3965,t3967,t3968,t397,t3970,t3972,t3977,t3981,t3982,t3985,t3989,t3990,t3993,t3994,t3998,t4,t4000,t4001,t4005,t4006,t4007,t4009,t401,t4011,t4013,t4014,t4016,t4018,t4019,t402,t4025,t4026,t4029,t4031,t4032,t4033,t4034,t4035,t4036,t4037,t404,t4043,t4044,t4046,t4047,t4048,t405,t4055,t4056,t4057,t4059,t4060,t4061,t4062,t4063,t4066,t4067,t4068,t4070,t4074,t4075,t4078,t4079,t408,t4080,t4081,t4083,t4084,t4085,t4088,t4089,t4090,t4091,t4092,t4095,t4097,t4099,t4103,t4104,t4105,t4109,t4115,t4118,t4119,t4121,t4123,t4125,t4129,t413,t4131,t4132,t4134,t4137,t4138,t414,t4140,t4142,t4143,t4145,t4147,t4148,t4149,t415,t4150,t4152,t4154,t4159,t4162,t4165,t4168,t4172,t4175,t4176,t4178,t418,t4183,t4185,t4188,t4190,t4192,t4195,t4198,t4199,t4200,t4202,t4203,t4204,t4208,t421,t4210,t4211,t4212,t4216,t4217,t4218,t4219,t4220,t4221,t4222,t4223,t4224,t4225,t4226,t4230,t4231,t4232,t4233,t4238,t4241,t4243,t4244,t4245,t4246,t4247,t4248,t4249,t425,t4250,t4252,t4258,t4260,t4261,t4262,t4263,t4264,t4265,t4271,t4276,t4277,t4278,t4280,t4282,t4284,t4286,t4287,t4292,t4294,t4295,t4301,t4305,t4308,t4309,t4310,t4311,t4313,t4316,t4317,t4319,t432,t4320,t4323,t4324,t4325,t4327,t4329,t4330,t4331,t4332,t4333,t4334,t4335,t4336,t434,t4341,t4343,t4344,t4345,t4347,t435,t4350,t4352,t4354,t436,t4361,t4362,t4365,t4367,t4368,t4369,t437,t4370,t4371,t4374,t4375,t4377,t4379,t4380,t4381,t4384,t4385,t4387,t4388,t4389,t439,t4390,t4391,t4399,t440,t4403,t4405,t4406,t4407,t4408,t4409,t441,t4410,t4415,t4416,t4417,t4418,t4419,t4420,t4423,t4426,t4428,t4429,t443,t4430,t4435,t4439,t444,t4442,t4444,t4448,t4449,t4452,t4454,t4455,t4456,t4457,t4459,t4466,t4469,t4471,t4473,t4474,t4475,t4476,t4477,t4478,t4479,t4484,t4493,t4495,t4496,t4499,t4503,t4505,t4507,t4508,t4511,t4512,t4514,t4515,t4517,t4518,t4519,t4520,t4521,t4526,t4528,t4529,t4532,t4533,t4535,t4536,t4538,t4539,t4540,t4541,t4542,t4545,t4546,t4547,t4549,t4550,t4551,t4554,t4556,t4557,t4559,t4562,t4564,t4565,t4566,t4568,t4569,t4570,t4571,t4573,t4574,t4575,t4578,t4579,t4581,t4582,t4584,t4589,t4590,t4592,t4594,t4595,t4597,t460,t4601,t4603,t4604,t4606,t4608,t4609,t4610,t4611,t4612,t4614,t4615,t4617,t4618,t4619,t4620,t4621,t4623,t4625,t4629,t463,t4631,t4633,t4636,t4639,t4640,t4641,t4644,t4646,t4647,t4648,t4649,t4650,t4652,t4653,t4655,t4656,t4658,t4661,t4667,t4668,t4669,t4670,t4671,t4672,t4673,t4674,t4675,t4676,t4679,t4683,t4685,t4686,t4691,t4692,t4694,t4695,t4697,t4698,t4699,t4702,t4704,t4710,t4712,t4718,t4720,t4722,t4726,t4729,t4731,t4733,t4735,t4736,t4737,t4738,t4739,t4740,t4742,t4743,t4744,t4747,t4749,t475,t4751,t4753,t4754,t4756,t4757,t4759,t4762,t4763,t4764,t4765,t4766,t4768,t4770,t4772,t4773,t4774,t4775,t4776,t4777,t4778,t478,t4780,t4782,t4784,t4785,t4786,t4787,t4789,t4791,t4792,t4793,t4794,t4795,t4797,t4798,t4799,t48,t4801,t4802,t4804,t4805,t4807,t4811,t4812,t4813,t4814,t4815,t4816,t4817,t4818,t4819,t4820,t4822,t4823,t4824,t4826,t4828,t4829,t4830,t4831,t4832,t4833,t4838,t4840,t4841,t4844,t4847,t4849,t4850,t4851,t4852,t4855,t4856,t4857,t4858,t4859,t4860,t4861,t4863,t4868,t4869,t4872,t4873,t4875,t4876,t4879,t488,t4880,t4883,t4885,t4887,t4888,t4889,t4892,t4895,t4896,t4898,t49,t490,t4903,t4905,t4907,t4909,t4910,t4912,t4914,t4915,t4917,t4918,t4919,t4920,t4921,t4924,t4925,t4929,t4930,t4932,t4934,t4935,t4937,t494,t4940,t4942,t4946,t4949,t4950,t4953,t4955,t4957,t4958,t496,t4961,t4962,t4964,t4965,t4967,t497,t4970,t4971,t4972,t4973,t4977,t4979,t498,t4980,t4983,t4984,t4985,t4987,t4988,t499,t4990,t4992,t4995,t4996,t5,t50,t500,t5001,t501,t5010,t5014,t5020,t5025,t5026,t5030,t5032,t5034,t5035,t5036,t5038,t5039,t504,t5041,t5042,t5043,t5044,t5046,t5047,t5048,t505,t5054,t5055,t5056,t5059,t5060,t5061,t5062,t5063,t5064,t5065,t5066,t5067,t5069,t5070,t5071,t5072,t5073,t5074,t5075,t5079,t5080,t5081,t5082,t5084,t5085,t5086,t5087,t509,t5091,t5094,t5095,t5097,t5099,t51,t510,t5100,t5101,t5105,t5108,t5109,t511,t5116,t5117,t512,t5120,t5121,t5122,t5125,t5127,t5131,t5133,t5136,t514,t5141,t5143,t5144,t5145,t5146,t5147,t5148,t5149,t515,t5150,t5151,t5153,t5156,t5158,t516,t5161,t5163,t5164,t5166,t5168,t5169,t517,t5170,t5174,t5176,t5179,t518,t5180,t5181,t5185,t5187,t5189,t5190,t5191,t5193,t5200,t5203,t5207,t5208,t5209,t5210,t5213,t5215,t5219,t5221,t5223,t5224,t5225,t5229,t523,t5231,t5235,t5239,t524,t5241,t5242,t5243,t5244,t5246,t5247,t5250,t5252,t5253,t5257,t5258,t5259,t5263,t5265,t5266,t5269,t527,t5277,t5278,t5279,t528,t5280,t5284,t5288,t5289,t529,t5290,t5291,t5292,t5293,t5294,t5295,t5296,t5298,t53,t530,t5300,t5301,t5302,t5303,t5304,t5305,t5306,t5307,t5308,t5309,t531,t5310,t5312,t5317,t5319,t5322,t5326,t5328,t5329,t5331,t5332,t5334,t5340,t5341,t5342,t5343,t5344,t5345,t5348,t5349,t535,t5350,t5353,t5354,t5355,t5356,t5357,t5358,t5359,t536,t5360,t5364,t5365,t5366,t5369,t5371,t5372,t5375,t5376,t5377,t5380,t5382,t5384,t5385,t5388,t5389,t5390,t5392,t5393,t5394,t5397,t5398,t5399,t54,t5401,t5402,t5403,t5405,t5406,t5407,t5408,t5410,t5411,t5412,t5413,t5416,t5417,t5418,t5419,t5420,t5421,t5422,t5423,t5424,t5425,t5426,t5429,t5430,t5433,t5435,t5436,t5439,t5441,t5442,t5445,t5446,t5447,t5449,t5450,t5452,t5453,t5454,t5455,t5457,t5459,t5460,t5461,t5465,t5467,t5469,t5472,t5473,t5474,t5475,t5478,t5480,t5482,t5486,t5490,t5492,t5493,t5494,t5495,t5497,t5498,t5499,t55,t5500,t5501,t5504,t5505,t5506,t5507,t5508,t5510,t5512,t5513,t5514,t5517,t5518,t5519,t5522,t5526,t5527,t5528,t5529,t5532,t5533,t5534,t5536,t5537,t5539,t5543,t5544,t5545,t5546,t5547,t5549,t5550,t5551,t5552,t5553,t5557,t5559,t556,t5561,t5564,t5565,t5567,t5569,t557,t5570,t5572,t5573,t5575,t5576,t5578,t5579,t558,t5581,t5582,t5583,t5584,t5586,t5587,t5588,t5589,t5590,t5591,t5592,t5595,t5598,t5599,t56,t560,t5600,t5601,t5602,t5603,t5604,t5607,t5608,t5609,t5612,t5613,t5614,t5615,t5616,t5617,t5619,t562,t5620,t5621,t5622,t5627,t5628,t5629,t5630,t5631,t5634,t5635,t5636,t5637,t5639,t5641,t5642,t5644,t5646,t5647,t5648,t565,t5651,t5652,t5656,t5657,t5658,t5659,t566,t5661,t5663,t5664,t5665,t5670,t5671,t5674,t5675,t5676,t5678,t5679,t5681,t5682,t5683,t5684,t5685,t5686,t569,t5690,t5692,t5696,t5697,t5698,t5699,t57,t5701,t5703,t5704,t5705,t5710,t5711,t5715,t5716,t5719,t5720,t5722,t5724,t5725,t5726,t5729,t5730,t5732,t5733,t5734,t5735,t5736,t5737,t5741,t5745,t5747,t5749,t5753,t5755,t5756,t5757,t5759,t5761,t5762,t5763,t5764,t5766,t5767,t5770,t5771,t5773,t5774,t5775,t5776,t5777,t5778,t5781,t5783,t5784,t5786,t5797,t58,t5800,t5801,t5803,t5804,t5805,t5806,t5807,t5808,t5809,t5810,t5811,t5814,t5815,t5816,t5817,t5822,t5823,t5824,t5831,t5832,t5833,t5835,t5836,t5837,t5840,t5841,t5842,t5843,t5845,t5847,t5850,t5851,t5854,t5859,t5860,t5861,t5862,t5865,t5866,t5868,t5870,t5871,t5873,t5876,t5878,t5879,t5882,t5883,t5884,t5886,t5888,t5890,t5891,t5893,t5895,t5896,t5897,t5899,t5901,t5903,t5905,t5906,t5907,t5908,t5909,t5910,t5911,t5913,t5916,t5917,t5919,t5923,t5924,t5930,t5931,t5933,t5934,t5935,t5936,t5937,t594,t5942,t5944,t5946,t5947,t5949,t595,t5950,t5952,t5953,t5954,t5955,t5956,t5959,t596,t5961,t5962,t5963,t5964,t5965,t5966,t5967,t5969,t5971,t5973,t5974,t5975,t5976,t5977,t5978,t5979,t598,t5980,t5982,t5983,t5985,t5987,t5988,t5989,t599,t5990,t5991,t5992,t5995,t5998,t5999,t6,t60,t600,t6000,t6001,t6002,t6003,t6004,t6005,t6006,t6007,t6008,t6009,t6010,t6016,t6017,t6019,t6020,t6021,t6022,t6025,t6026,t6027,t6029,t6030,t6033,t6036,t6038,t6039,t6042,t6043,t6044,t6046,t6047,t6048,t605,t6051,t6052,t6054,t6055,t6056,t6058,t606,t6060,t6061,t6062,t6063,t6066,t6067,t6068,t6069,t6070,t6071,t6072,t6073,t6076,t6078,t608,t6081,t6082,t6086,t6087,t6089,t609,t6091,t6092,t6093,t6094,t6096,t6097,t61,t610,t6101,t6106,t6109,t611,t6111,t6112,t6114,t6115,t6116,t6117,t6119,t6120,t6124,t6125,t6126,t6127,t6128,t6129,t6130,t6131,t6132,t6134,t6135,t6136,t6138,t6139,t614,t6140,t6141,t6142,t6145,t6146,t6147,t6149,t6150,t6151,t6152,t6153,t6154,t6156,t6157,t6160,t6161,t6162,t6163,t6164,t6166,t6167,t6168,t6169,t6175,t6176,t6178,t6179,t6180,t6182,t6183,t6184,t6185,t6186,t6187,t6188,t6191,t6192,t6193,t6195,t6196,t62,t6201,t6203,t6204,t6207,t6211,t6213,t6214,t6216,t6218,t6219,t6222,t6224,t6225,t6226,t6229,t6231,t6234,t6235,t6236,t6237,t6241,t6242,t6244,t6248,t6252,t6253,t6254,t6255,t6256,t6257,t6258,t6261,t6262,t6263,t6264,t6265,t6266,t6267,t6268,t6269,t6270,t6272,t6274,t6275,t6277,t6278,t6293,t6294,t6296,t6298,t6299,t63,t6300,t6302,t6303,t6305,t6306,t6307,t6308,t6309,t6312,t6313,t6316,t6317,t6319,t6321,t6323,t6327,t6328,t6332,t6333,t6335,t6337,t6339,t634,t6340,t6342,t6344,t6346,t6349,t635,t6350,t6352,t6353,t6354,t6355,t6356,t6357,t6358,t636,t6360,t6363,t6364,t6365,t6366,t6368,t6369,t637,t6370,t6372,t6373,t6375,t6376,t6377,t6378,t6379,t638,t6383,t6385,t6386,t6388,t6389,t639,t6390,t6391,t6395,t6398,t640,t6400,t6401,t6403,t6404,t6405,t6407,t641,t6411,t6412,t6417,t6418,t6421,t6422,t6423,t6424,t6425,t6426,t6427,t6429,t6434,t6435,t6436,t6437,t6438,t6440,t6441,t6442,t6443,t6445,t6446,t6447,t6448,t6449,t6451,t6452,t6454,t6455,t6456,t6457,t6460,t6461,t6462,t6469,t647,t6470,t6473,t6475,t6481,t6483,t6484,t6485,t6486,t6487,t6488,t649,t6490,t6491,t6492,t6493,t6494,t6497,t6499,t650,t6500,t6501,t6502,t6505,t6509,t651,t6510,t6513,t6516,t6517,t652,t6520,t6521,t6522,t6523,t6525,t6526,t6527,t6528,t6529,t653,t6530,t6531,t6532,t6533,t6534,t6537,t6538,t6539,t6540,t6541,t6542,t6543,t6544,t6545,t6547,t6548,t6549,t6557,t6558,t6560,t6561,t6562,t6563,t6564,t657,t6570,t6574,t6575,t6576,t6579,t658,t6580,t6582,t6583,t6585,t6586,t6588,t6589,t659,t6592,t6594,t6595,t6596,t6597,t6599,t660,t6600,t6602,t6603,t6604,t6606,t6607,t6608,t6609,t661,t6610,t6611,t6612,t6613,t6614,t6616,t6618,t6619,t6621,t6624,t6625,t6628,t6629,t663,t6632,t6634,t6635,t6637,t6638,t6639,t664,t6640,t6642,t6644,t6645,t6646,t6647,t6648,t6649,t6650,t6651,t6655,t6657,t6658,t6659,t6662,t6664,t6665,t6667,t6668,t6669,t667,t6670,t6673,t6674,t6675,t6676,t6678,t6679,t6680,t6681,t6682,t6685,t6686,t6687,t6689,t6690,t6692,t6693,t6695,t6696,t6697,t6699,t670,t6700,t6701,t6702,t6703,t6704,t6705,t6706,t6707,t6710,t6711,t6712,t6715,t6716,t6719,t6721,t6722,t6725,t6726,t6727,t6732,t6733,t6734,t6736,t6738,t6739,t6740,t6741,t6742,t6744,t6746,t6747,t6750,t6754,t6755,t6757,t6758,t6759,t676,t6760,t6763,t6764,t6766,t6767,t677,t6770,t6771,t6772,t6775,t6776,t6779,t678,t6783,t6784,t6786,t6790,t6792,t6793,t6796,t6797,t6799,t680,t6800,t6805,t6806,t6807,t6808,t6809,t681,t6810,t6813,t6817,t6821,t6822,t6823,t6824,t6826,t6829,t683,t6830,t6831,t6834,t6838,t6839,t684,t6840,t6841,t6842,t6843,t6845,t6849,t685,t6853,t6856,t6857,t6859,t686,t6860,t6862,t6863,t6866,t6867,t687,t6870,t6871,t6872,t6874,t6875,t6877,t6878,t688,t6880,t6884,t6885,t6887,t6889,t6890,t6891,t6896,t6897,t6898,t690,t6901,t6902,t6903,t6904,t6905,t6906,t6908,t6909,t691,t6910,t6911,t6914,t692,t6924,t6925,t6927,t6928,t6929,t693,t6930,t6931,t6932,t6933,t6934,t6935,t6937,t6938,t6939,t6940,t6941,t6942,t6944,t6946,t6947,t6948,t6949,t6956,t6959,t696,t6960,t6961,t6965,t6966,t6974,t6975,t6976,t6977,t6978,t6979,t6981,t6982,t6983,t6984,t6987,t6989,t6990,t6991,t6998,t6999,t7,t700,t7001,t7002,t7003,t7010,t7011,t7012,t7013,t7016,t7017,t7018,t7019,t702,t7020,t7021,t7022,t7023,t7024,t7025,t7026,t7027,t7028,t703,t7031,t7032,t7033,t7034,t7035,t7039,t7042,t7043,t7044,t7048,t7049,t7050,t7051,t7052,t7054,t7055,t7056,t7057,t7059,t7060,t7061,t7062,t7063,t7064,t7065,t7066,t7069,t7074,t7075,t7078,t7080,t7081,t7083,t7086,t7088,t7090,t7093,t7094,t7097,t7100,t7101,t7102,t7104,t7107,t7108,t7109,t7110,t7111,t7113,t7115,t7117,t7118,t7119,t7122,t7123,t7124,t7125,t7127,t7128,t7129,t7130,t7131,t7132,t7134,t7135,t7136,t7137,t7138,t7141,t7143,t7144,t7146,t7147,t7152,t7153,t7155,t7156,t7163,t7165,t7166,t7168,t7170,t7173,t7174,t7176,t7178,t7180,t7182,t7185,t7186,t7188,t7189,t7190,t7191,t7192,t7193,t7194,t7198,t7199,t7200,t7201,t7203,t7205,t7206,t7207,t7208,t7209,t7210,t7212,t7213,t7216,t7220,t7221,t7222,t7223,t7224,t7225,t7226,t7227,t7228,t7229,t7230,t7231,t7232,t7233,t7238,t7239,t7241,t7246,t7250,t7251,t7253,t7254,t7256,t7257,t7258,t7259,t7260,t7263,t7265,t7266,t7267,t7268,t7272,t7276,t7278,t728,t7282,t7283,t7284,t7285,t7286,t7288,t7289,t7292,t7297,t7298,t7299,t7300,t7301,t7302,t7303,t7304,t7305,t7306,t7307,t7308,t7309,t7311,t7313,t7315,t7316,t7318,t7319,t7320,t7323,t7327,t7329,t7330,t7331,t7332,t7333,t7334,t7335,t7336,t7337,t7340,t7342,t7343,t7344,t7345,t7346,t7348,t7349,t735,t7357,t7358,t736,t7361,t7362,t7363,t7365,t7366,t7367,t7368,t7369,t7370,t7371,t7372,t7373,t7378,t738,t7384,t7385,t7393,t7394,t7395,t7396,t7397,t7398,t7399,t740,t7400,t7401,t7402,t7403,t7405,t7407,t7408,t7409,t7411,t7412,t7413,t7414,t7415,t7416,t7417,t7419,t7420,t7422,t7423,t7425,t7428,t7429,t7430,t7431,t7432,t7433,t7434,t7438,t7441,t7442,t7443,t7446,t7447,t7449,t7450,t7451,t7452,t7457,t746,t7460,t7461,t7463,t7464,t7465,t7466,t7467,t7469,t747,t7470,t7471,t7473,t7474,t7475,t7477,t7478,t7479,t748,t7480,t7481,t7494,t7500,t7505,t7507,t7511,t7513,t7516,t7518,t7519,t752,t7524,t7525,t7526,t7529,t7530,t7532,t7534,t7535,t7536,t7537,t754,t7541,t7542,t7547,t7549,t7550,t7554,t7555,t7557,t7559,t756,t7564,t7566,t7571,t7575,t7578,t7579,t758,t7589,t759,t7590,t7594,t7595,t7596,t7597,t7598,t7599,t7600,t7601,t7602,t7607,t7608,t7620,t7621,t7634,t7636,t7644,t7649,t7651,t7652,t7655,t7656,t7657,t7658,t7659,t766,t7660,t7661,t7663,t7664,t7667,t7672,t7673,t7674,t7675,t7678,t768,t7686,t7687,t7690,t772,t7721,t7722,t7725,t7735,t7751,t7756,t7757,t7764,t7765,t7769,t7788,t7790,t7793,t7795,t7802,t7807,t781,t7810,t782,t7825,t7827,t7833,t7872,t7877,t7897,t7902,t7904,t7914,t7924,t793,t7961,t7962,t7966,t7971,t7976,t798,t7983,t7999,t8,t8002,t8021,t8038,t8046,t8050,t8051,t8052,t8090,t8096,t8117,t8126,t8129,t8130,t8182,t8184,t8202,t8206,t8231,t8232,t8239,t826,t827,t828,t829,t832,t833,t834,t836,t837,t838,t839,t84,t85,t850,t852,t86,t861,t864,t868,t87,t879,t884,t885,t888,t889,t890,t891,t892,t893,t894,t897,t898,t9,t90,t900,t901,t902,t904,t905,t906,t907,t911,t912,t913,t914,t915,t916,t917,t918,t92,t929,t930,t931,t933,t934,t936,t938,t940,t943,t944,t945,t947,t949,t950,t951,t953,t956,t957,t966,t967,t968,t969,t97,t972,t973,t974,t976,t98,t981,t982,t984,t986,t988,t99,t992,t993,t994,t997,t999});
end
function tau = ft_13(ct)
[dq1,dq2,dq3,dq4,dq5,dq6,t10,t1001,t1002,t1003,t1004,t1005,t1006,t1007,t1009,t101,t1010,t1023,t1024,t1025,t1026,t1027,t1030,t1032,t1033,t1034,t1035,t1037,t1038,t1039,t1041,t1046,t105,t1053,t106,t1063,t1068,t107,t1073,t1074,t1075,t1076,t1077,t1078,t1079,t108,t1080,t1081,t1083,t1084,t1086,t1087,t1089,t109,t1090,t1092,t1095,t1096,t1097,t1098,t11,t110,t111,t1115,t1117,t1118,t112,t1120,t1122,t1123,t1127,t1128,t1129,t113,t1130,t1131,t1132,t1133,t114,t1149,t1150,t1153,t1156,t1157,t1158,t1159,t1162,t1163,t1166,t1170,t1171,t1172,t1173,t1174,t1179,t1180,t1182,t1183,t1186,t1188,t1189,t1193,t1194,t1195,t1196,t1198,t1199,t12,t1201,t1203,t1204,t1205,t1207,t1208,t1210,t1211,t1212,t1215,t1218,t1219,t1220,t1221,t1222,t1227,t1228,t1229,t123,t1230,t1231,t1234,t1235,t1239,t124,t1241,t1242,t1243,t1244,t1245,t1247,t125,t1250,t1251,t1252,t1253,t1254,t1256,t126,t1263,t1266,t127,t1274,t128,t1284,t1285,t1287,t129,t1291,t1293,t1295,t1298,t1299,t13,t130,t1300,t1301,t1308,t1309,t1313,t1317,t1318,t1319,t1320,t1323,t1325,t1326,t1327,t1329,t1331,t1332,t1333,t1334,t1339,t1343,t1344,t1345,t1346,t1347,t1349,t1351,t1352,t1354,t1357,t1358,t1359,t1360,t1361,t1364,t1365,t1366,t1368,t1369,t1371,t1373,t1375,t1376,t1377,t1378,t1379,t1380,t1383,t1385,t1386,t1387,t1388,t1389,t1390,t1392,t1393,t1394,t1395,t1397,t1398,t140,t1405,t1406,t141,t1411,t1412,t1415,t1416,t1417,t1419,t1420,t1422,t1423,t1424,t1426,t1427,t1429,t143,t1430,t1432,t1433,t1434,t1435,t1439,t1440,t1441,t1442,t1443,t1445,t1446,t1450,t1452,t1453,t1456,t1457,t1459,t1460,t1462,t1464,t1465,t1466,t1467,t1468,t1469,t1470,t1473,t1477,t1479,t1480,t1481,t1482,t1484,t1488,t1490,t1491,t1492,t1493,t1494,t1495,t1496,t1500,t1505,t1507,t1508,t1511,t1513,t1516,t1517,t1518,t1519,t1522,t1523,t1524,t1525,t1526,t1528,t1541,t1542,t1543,t1545,t1546,t1547,t1548,t1549,t1552,t1553,t1555,t1556,t1557,t1571,t1572,t1573,t1576,t1577,t1578,t1579,t1581,t1583,t1584,t1585,t1586,t1587,t1592,t1594,t1595,t1596,t1609,t1613,t1615,t1619,t1620,t163,t1637,t1639,t164,t1641,t1642,t1643,t1644,t1645,t1646,t1656,t1659,t166,t1660,t1661,t1662,t1663,t1664,t1666,t1669,t1670,t1671,t1672,t1673,t1675,t1676,t1678,t1679,t1680,t1681,t1684,t1685,t1686,t1687,t1690,t1691,t1692,t1694,t1696,t1697,t1701,t1702,t1703,t1706,t1707,t1710,t1711,t1713,t1716,t1717,t1719,t1720,t1726,t1727,t1730,t1732,t1735,t1739,t1744,t1745,t1749,t1750,t1751,t1752,t1753,t1754,t1755,t1756,t1758,t1759,t1760,t1761,t1762,t1763,t1764,t1768,t1771,t1772,t1773,t1776,t1778,t1779,t178,t1785,t1787,t1796,t1799,t18,t1800,t1801,t1803,t1804,t1806,t1815,t1816,t1818,t1819,t182,t1820,t1821,t1823,t1824,t1825,t1826,t1827,t1828,t1829,t183,t1832,t1833,t1835,t1836,t1837,t1839,t1840,t1841,t1842,t1844,t1845,t1847,t1848,t185,t1850,t1851,t1853,t1854,t1856,t1857,t186,t1860,t1865,t1866,t1868,t1869,t187,t1874,t1876,t1877,t1878,t1879,t1882,t1883,t189,t1895,t1896,t1898,t1899,t19,t1900,t1901,t1902,t1903,t1904,t1905,t1906,t1908,t1909,t191,t1911,t1913,t1914,t1917,t1919,t1920,t1921,t1922,t1925,t1926,t1928,t193,t1930,t1931,t1933,t1936,t1937,t194,t1942,t1943,t1944,t1947,t1949,t195,t1958,t1959,t1962,t1964,t1993,t1994,t1995,t1996,t1997,t1998,t2,t20,t200,t2000,t2001,t2002,t2003,t2004,t2006,t2009,t2012,t2013,t2014,t2015,t2016,t2017,t2018,t202,t2023,t2024,t2027,t2028,t2029,t203,t2034,t2036,t2038,t2039,t204,t2043,t2044,t2045,t2053,t2054,t2055,t2056,t2059,t2061,t2067,t2068,t2069,t2072,t2074,t2075,t2078,t2079,t208,t2083,t2084,t2085,t2086,t2087,t2088,t2089,t2090,t2094,t2096,t2097,t21,t210,t2103,t2107,t2109,t211,t2110,t2111,t2112,t2115,t2116,t2117,t2118,t212,t2120,t2124,t2125,t2126,t2127,t2129,t2132,t2133,t2134,t2136,t2138,t214,t2140,t2141,t2147,t2148,t215,t2151,t2152,t2157,t216,t2161,t2168,t2171,t2178,t2179,t2185,t2193,t22,t2200,t2201,t2202,t2203,t2205,t2206,t2207,t2208,t2212,t2216,t2217,t2219,t2221,t2222,t2223,t2224,t2225,t2227,t2228,t2229,t2231,t2234,t2235,t2236,t2237,t2238,t224,t2245,t2246,t2247,t2248,t2250,t2254,t2259,t2276,t228,t2280,t2283,t2284,t2285,t2287,t229,t2290,t2292,t2293,t2295,t230,t2308,t231,t2314,t2318,t2319,t2320,t2322,t2323,t2324,t2325,t2326,t2327,t2343,t2347,t2348,t2353,t2358,t2362,t2363,t2364,t2373,t2375,t2379,t2383,t2387,t2394,t2395,t2397,t2398,t2400,t2401,t2403,t2404,t2405,t2409,t2411,t2412,t2413,t2414,t2415,t2417,t2419,t2421,t2422,t2423,t2426,t2430,t2431,t2432,t2433,t2437,t2438,t2439,t244,t2440,t245,t2450,t2451,t2452,t2453,t2455,t2456,t2457,t246,t2464,t2466,t2467,t2469,t247,t2471,t2472,t2473,t2474,t2477,t2478,t2479,t248,t2480,t2481,t2482,t2483,t2484,t2485,t2486,t2487,t2488,t249,t2491,t2499,t250,t2504,t2507,t2508,t251,t252,t2524,t2525,t2527,t2529,t253,t2531,t2536,t2543,t2546,t255,t2551,t2552,t2553,t2555,t2559,t2560,t2565,t2566,t2568,t2569,t2571,t2574,t2578,t2580,t2582,t2583,t2585,t2586,t2588,t2591,t2593,t2594,t2598,t260,t2601,t2603,t2604,t2605,t2608,t2609,t261,t2610,t2611,t2612,t2614,t2615,t262,t2622,t2625,t2628,t2629,t263,t2632,t2634,t2641,t2644,t2645,t2648,t2649,t265,t2651,t2655,t2657,t2659,t2660,t2661,t2662,t2663,t267,t2672,t2679,t2692,t2694,t2695,t2700,t2701,t2703,t2705,t2725,t2726,t2727,t2729,t2730,t2732,t2733,t2734,t2735,t2738,t2739,t2740,t2741,t2743,t2747,t2748,t2752,t2753,t2756,t2760,t2763,t2764,t2765,t2767,t2769,t2772,t2784,t2785,t2792,t2794,t2795,t2796,t28,t2801,t2803,t2804,t2806,t2809,t2811,t2812,t2813,t2815,t2817,t2819,t2820,t2821,t2822,t2825,t2828,t2829,t2830,t2832,t2833,t2836,t2839,t2843,t2844,t2848,t2850,t2852,t2854,t2856,t2861,t2862,t2863,t2864,t2866,t2869,t2877,t2878,t2880,t2887,t2888,t2890,t2892,t2899,t29,t2900,t2901,t2903,t2904,t2905,t2906,t2910,t2911,t2912,t2917,t2919,t2921,t2922,t2923,t2925,t2927,t2928,t2931,t2932,t2933,t2934,t2938,t2939,t2940,t2943,t2949,t295,t2951,t2952,t2953,t2954,t2956,t2957,t2959,t296,t2960,t2964,t2965,t2968,t297,t2970,t2973,t2975,t2977,t298,t2981,t2988,t2990,t2991,t2992,t2993,t2996,t3,t3002,t3004,t3006,t3007,t3008,t3010,t3011,t3012,t3013,t3016,t3018,t3019,t3025,t3026,t303,t3030,t3033,t3037,t3039,t304,t3040,t3043,t3045,t3046,t3047,t3049,t305,t3050,t3056,t3058,t3059,t3060,t3065,t3066,t3067,t3068,t3070,t3071,t3072,t3073,t3074,t3075,t3077,t3078,t3079,t308,t3085,t3087,t3088,t309,t3091,t3092,t3095,t3098,t3099,t3100,t3101,t3104,t3106,t3109,t311,t3110,t3111,t3119,t312,t3125,t3129,t313,t3130,t3131,t3136,t3138,t3139,t3144,t3147,t3149,t3150,t3152,t3159,t3170,t3173,t3174,t3177,t3186,t3187,t3192,t3193,t3194,t3195,t3198,t3200,t3203,t3206,t3207,t3208,t3209,t3210,t3211,t3212,t3213,t3214,t3215,t3217,t3219,t3220,t3222,t3223,t3224,t3225,t3226,t3227,t3228,t3231,t3232,t3233,t3234,t3235,t3236,t3237,t3238,t3239,t3242,t3247,t3249,t3250,t3253,t3254,t3255,t3256,t3258,t3260,t3262,t3265,t3269,t3270,t3271,t3273,t3274,t3275,t3280,t3283,t3284,t3286,t3287,t329,t3296,t3297,t3298,t330,t3303,t3305,t3307,t3308,t331,t3316,t332,t3323,t3324,t3326,t3327,t3328,t3329,t3330,t3331,t3332,t3333,t3334,t3335,t3336,t334,t3342,t3345,t3346,t3348,t3353,t3359,t336,t3361,t3363,t3364,t3365,t3366,t337,t3377,t3378,t3379,t338,t3384,t3386,t3387,t339,t3394,t3395,t3396,t3397,t3399,t3402,t3405,t341,t3410,t3411,t3412,t3413,t3416,t3419,t342,t3421,t3422,t3424,t3425,t3426,t3430,t3435,t3436,t3438,t3439,t344,t3440,t3442,t3443,t3444,t3445,t3446,t3449,t3454,t3458,t346,t3463,t3467,t3470,t3471,t3472,t3474,t3475,t3476,t3477,t348,t3480,t3481,t3483,t3484,t3485,t3488,t349,t3491,t3492,t3496,t3498,t350,t3502,t3504,t3506,t3507,t3508,t3511,t3513,t3519,t352,t3520,t3522,t3523,t3526,t3527,t3529,t353,t3531,t3532,t3533,t3535,t3538,t354,t3542,t3543,t3544,t3545,t3548,t3549,t355,t3552,t3553,t3554,t3559,t356,t3565,t3566,t3567,t3568,t357,t3575,t3578,t358,t3586,t3587,t3588,t3590,t3591,t3592,t3593,t3596,t3598,t3599,t360,t3600,t3601,t3602,t3603,t3604,t3608,t3609,t3610,t3612,t3613,t3614,t3617,t3620,t3621,t3623,t3626,t3627,t3628,t3629,t3630,t3633,t3638,t3639,t3640,t3641,t3645,t3646,t3648,t3652,t3653,t3655,t3656,t3657,t3658,t3663,t3667,t3668,t3670,t3671,t3674,t3675,t3676,t3677,t3679,t3680,t3681,t3682,t3683,t3684,t3687,t3689,t369,t3690,t3691,t3692,t3694,t3697,t3698,t370,t3700,t3701,t3702,t3703,t3704,t3705,t3708,t3709,t3710,t3711,t3712,t3713,t3714,t3715,t3717,t3719,t372,t3720,t3721,t3722,t3725,t3726,t3727,t3728,t3729,t3730,t3733,t3734,t3735,t3736,t3737,t3738,t3739,t374,t3740,t3741,t3744,t3745,t3747,t3748,t3750,t3751,t3752,t3754,t3755,t3756,t3757,t3759,t3764,t3766,t3767,t3769,t3770,t3772,t3774,t3775,t3776,t3777,t3778,t3780,t3781,t3782,t3785,t3787,t3789,t3792,t3793,t3794,t3796,t3798,t3806,t3807,t3808,t3809,t3812,t3813,t3814,t3820,t3821,t3822,t3824,t3825,t3826,t3829,t3831,t3837,t3838,t3839,t384,t3840,t3841,t3852,t3854,t3856,t3857,t386,t3860,t3861,t3862,t3863,t3864,t3868,t387,t3872,t3874,t3875,t3876,t3882,t3884,t3885,t3887,t3888,t3889,t389,t3892,t3894,t3896,t3897,t3898,t3899,t3900,t3901,t3902,t3903,t3904,t3906,t3908,t3909,t3912,t3913,t3916,t3918,t3919,t3920,t3921,t3922,t3923,t3926,t3930,t3931,t3932,t3935,t3936,t3939,t3941,t3944,t3945,t3946,t3948,t3949,t3950,t3953,t3956,t3959,t3964,t3965,t3967,t3968,t397,t3970,t3972,t3977,t3981,t3982,t3985,t3989,t3990,t3993,t3994,t3998,t4,t4000,t4001,t4005,t4006,t4007,t4009,t401,t4011,t4013,t4014,t4016,t4018,t4019,t402,t4025,t4026,t4029,t4031,t4032,t4033,t4034,t4035,t4036,t4037,t404,t4043,t4044,t4046,t4047,t4048,t405,t4055,t4056,t4057,t4059,t4060,t4061,t4062,t4063,t4066,t4067,t4068,t4070,t4074,t4075,t4078,t4079,t408,t4080,t4081,t4083,t4084,t4085,t4088,t4089,t4090,t4091,t4092,t4095,t4097,t4099,t4103,t4104,t4105,t4109,t4115,t4118,t4119,t4121,t4123,t4125,t4129,t413,t4131,t4132,t4134,t4137,t4138,t414,t4140,t4142,t4143,t4145,t4147,t4148,t4149,t415,t4150,t4152,t4154,t4159,t4162,t4165,t4168,t4172,t4175,t4176,t4178,t418,t4183,t4185,t4188,t4190,t4192,t4195,t4198,t4199,t4200,t4202,t4203,t4204,t4208,t421,t4210,t4211,t4212,t4216,t4217,t4218,t4219,t4220,t4221,t4222,t4223,t4224,t4225,t4226,t4230,t4231,t4232,t4233,t4238,t4241,t4243,t4244,t4245,t4246,t4247,t4248,t4249,t425,t4250,t4252,t4258,t4260,t4261,t4262,t4263,t4264,t4265,t4271,t4276,t4277,t4278,t4280,t4282,t4284,t4286,t4287,t4292,t4294,t4295,t4301,t4305,t4308,t4309,t4310,t4311,t4313,t4316,t4317,t4319,t432,t4320,t4323,t4324,t4325,t4327,t4329,t4330,t4331,t4332,t4333,t4334,t4335,t4336,t434,t4341,t4343,t4344,t4345,t4347,t435,t4350,t4352,t4354,t436,t4361,t4362,t4365,t4367,t4368,t4369,t437,t4370,t4371,t4374,t4375,t4377,t4379,t4380,t4381,t4384,t4385,t4387,t4388,t4389,t439,t4390,t4391,t4399,t440,t4403,t4405,t4406,t4407,t4408,t4409,t441,t4410,t4415,t4416,t4417,t4418,t4419,t4420,t4423,t4426,t4428,t4429,t443,t4430,t4435,t4439,t444,t4442,t4444,t4448,t4449,t4452,t4454,t4455,t4456,t4457,t4459,t4466,t4469,t4471,t4473,t4474,t4475,t4476,t4477,t4478,t4479,t4484,t4493,t4495,t4496,t4499,t4503,t4505,t4507,t4508,t4511,t4512,t4514,t4515,t4517,t4518,t4519,t4520,t4521,t4526,t4528,t4529,t4532,t4533,t4535,t4536,t4538,t4539,t4540,t4541,t4542,t4545,t4546,t4547,t4549,t4550,t4551,t4554,t4556,t4557,t4559,t4562,t4564,t4565,t4566,t4568,t4569,t4570,t4571,t4573,t4574,t4575,t4578,t4579,t4581,t4582,t4584,t4589,t4590,t4592,t4594,t4595,t4597,t460,t4601,t4603,t4604,t4606,t4608,t4609,t4610,t4611,t4612,t4614,t4615,t4617,t4618,t4619,t4620,t4621,t4623,t4625,t4629,t463,t4631,t4633,t4636,t4639,t4640,t4641,t4644,t4646,t4647,t4648,t4649,t4650,t4652,t4653,t4655,t4656,t4658,t4661,t4667,t4668,t4669,t4670,t4671,t4672,t4673,t4674,t4675,t4676,t4679,t4683,t4685,t4686,t4691,t4692,t4694,t4695,t4697,t4698,t4699,t4702,t4704,t4710,t4712,t4718,t4720,t4722,t4726,t4729,t4731,t4733,t4735,t4736,t4737,t4738,t4739,t4740,t4742,t4743,t4744,t4747,t4749,t475,t4751,t4753,t4754,t4756,t4757,t4759,t4762,t4763,t4764,t4765,t4766,t4768,t4770,t4772,t4773,t4774,t4775,t4776,t4777,t4778,t478,t4780,t4782,t4784,t4785,t4786,t4787,t4789,t4791,t4792,t4793,t4794,t4795,t4797,t4798,t4799,t48,t4801,t4802,t4804,t4805,t4807,t4811,t4812,t4813,t4814,t4815,t4816,t4817,t4818,t4819,t4820,t4822,t4823,t4824,t4826,t4828,t4829,t4830,t4831,t4832,t4833,t4838,t4840,t4841,t4844,t4847,t4849,t4850,t4851,t4852,t4855,t4856,t4857,t4858,t4859,t4860,t4861,t4863,t4868,t4869,t4872,t4873,t4875,t4876,t4879,t488,t4880,t4883,t4885,t4887,t4888,t4889,t4892,t4895,t4896,t4898,t49,t490,t4903,t4905,t4907,t4909,t4910,t4912,t4914,t4915,t4917,t4918,t4919,t4920,t4921,t4924,t4925,t4929,t4930,t4932,t4934,t4935,t4937,t494,t4940,t4942,t4946,t4949,t4950,t4953,t4955,t4957,t4958,t496,t4961,t4962,t4964,t4965,t4967,t497,t4970,t4971,t4972,t4973,t4977,t4979,t498,t4980,t4983,t4984,t4985,t4987,t4988,t499,t4990,t4992,t4995,t4996,t5,t50,t500,t5001,t501,t5010,t5014,t5020,t5025,t5026,t5030,t5032,t5034,t5035,t5036,t5038,t5039,t504,t5041,t5042,t5043,t5044,t5046,t5047,t5048,t505,t5054,t5055,t5056,t5059,t5060,t5061,t5062,t5063,t5064,t5065,t5066,t5067,t5069,t5070,t5071,t5072,t5073,t5074,t5075,t5079,t5080,t5081,t5082,t5084,t5085,t5086,t5087,t509,t5091,t5094,t5095,t5097,t5099,t51,t510,t5100,t5101,t5105,t5108,t5109,t511,t5116,t5117,t512,t5120,t5121,t5122,t5125,t5127,t5131,t5133,t5136,t514,t5141,t5143,t5144,t5145,t5146,t5147,t5148,t5149,t515,t5150,t5151,t5153,t5156,t5158,t516,t5161,t5163,t5164,t5166,t5168,t5169,t517,t5170,t5174,t5176,t5179,t518,t5180,t5181,t5185,t5187,t5189,t5190,t5191,t5193,t5200,t5203,t5207,t5208,t5209,t5210,t5213,t5215,t5219,t5221,t5223,t5224,t5225,t5229,t523,t5231,t5235,t5239,t524,t5241,t5242,t5243,t5244,t5246,t5247,t5250,t5252,t5253,t5257,t5258,t5259,t5263,t5265,t5266,t5269,t527,t5277,t5278,t5279,t528,t5280,t5284,t5288,t5289,t529,t5290,t5291,t5292,t5293,t5294,t5295,t5296,t5298,t53,t530,t5300,t5301,t5302,t5303,t5304,t5305,t5306,t5307,t5308,t5309,t531,t5310,t5312,t5317,t5319,t5322,t5326,t5328,t5329,t5331,t5332,t5334,t5340,t5341,t5342,t5343,t5344,t5345,t5348,t5349,t535,t5350,t5353,t5354,t5355,t5356,t5357,t5358,t5359,t536,t5360,t5364,t5365,t5366,t5369,t5371,t5372,t5375,t5376,t5377,t5380,t5382,t5384,t5385,t5388,t5389,t5390,t5392,t5393,t5394,t5397,t5398,t5399,t54,t5401,t5402,t5403,t5405,t5406,t5407,t5408,t5410,t5411,t5412,t5413,t5416,t5417,t5418,t5419,t5420,t5421,t5422,t5423,t5424,t5425,t5426,t5429,t5430,t5433,t5435,t5436,t5439,t5441,t5442,t5445,t5446,t5447,t5449,t5450,t5452,t5453,t5454,t5455,t5457,t5459,t5460,t5461,t5465,t5467,t5469,t5472,t5473,t5474,t5475,t5478,t5480,t5482,t5486,t5490,t5492,t5493,t5494,t5495,t5497,t5498,t5499,t55,t5500,t5501,t5504,t5505,t5506,t5507,t5508,t5510,t5512,t5513,t5514,t5517,t5518,t5519,t5522,t5526,t5527,t5528,t5529,t5532,t5533,t5534,t5536,t5537,t5539,t5543,t5544,t5545,t5546,t5547,t5549,t5550,t5551,t5552,t5553,t5557,t5559,t556,t5561,t5564,t5565,t5567,t5569,t557,t5570,t5572,t5573,t5575,t5576,t5578,t5579,t558,t5581,t5582,t5583,t5584,t5586,t5587,t5588,t5589,t5590,t5591,t5592,t5595,t5598,t5599,t56,t560,t5600,t5601,t5602,t5603,t5604,t5607,t5608,t5609,t5612,t5613,t5614,t5615,t5616,t5617,t5619,t562,t5620,t5621,t5622,t5627,t5628,t5629,t5630,t5631,t5634,t5635,t5636,t5637,t5639,t5641,t5642,t5644,t5646,t5647,t5648,t565,t5651,t5652,t5656,t5657,t5658,t5659,t566,t5661,t5663,t5664,t5665,t5670,t5671,t5674,t5675,t5676,t5678,t5679,t5681,t5682,t5683,t5684,t5685,t5686,t569,t5690,t5692,t5696,t5697,t5698,t5699,t57,t5701,t5703,t5704,t5705,t5710,t5711,t5715,t5716,t5719,t5720,t5722,t5724,t5725,t5726,t5729,t5730,t5732,t5733,t5734,t5735,t5736,t5737,t5741,t5745,t5747,t5749,t5753,t5755,t5756,t5757,t5759,t5761,t5762,t5763,t5764,t5766,t5767,t5770,t5771,t5773,t5774,t5775,t5776,t5777,t5778,t5781,t5783,t5784,t5786,t5797,t58,t5800,t5801,t5803,t5804,t5805,t5806,t5807,t5808,t5809,t5810,t5811,t5814,t5815,t5816,t5817,t5822,t5823,t5824,t5831,t5832,t5833,t5835,t5836,t5837,t5840,t5841,t5842,t5843,t5845,t5847,t5850,t5851,t5854,t5859,t5860,t5861,t5862,t5865,t5866,t5868,t5870,t5871,t5873,t5876,t5878,t5879,t5882,t5883,t5884,t5886,t5888,t5890,t5891,t5893,t5895,t5896,t5897,t5899,t5901,t5903,t5905,t5906,t5907,t5908,t5909,t5910,t5911,t5913,t5916,t5917,t5919,t5923,t5924,t5930,t5931,t5933,t5934,t5935,t5936,t5937,t594,t5942,t5944,t5946,t5947,t5949,t595,t5950,t5952,t5953,t5954,t5955,t5956,t5959,t596,t5961,t5962,t5963,t5964,t5965,t5966,t5967,t5969,t5971,t5973,t5974,t5975,t5976,t5977,t5978,t5979,t598,t5980,t5982,t5983,t5985,t5987,t5988,t5989,t599,t5990,t5991,t5992,t5995,t5998,t5999,t6,t60,t600,t6000,t6001,t6002,t6003,t6004,t6005,t6006,t6007,t6008,t6009,t6010,t6016,t6017,t6019,t6020,t6021,t6022,t6025,t6026,t6027,t6029,t6030,t6033,t6036,t6038,t6039,t6042,t6043,t6044,t6046,t6047,t6048,t605,t6051,t6052,t6054,t6055,t6056,t6058,t606,t6060,t6061,t6062,t6063,t6066,t6067,t6068,t6069,t6070,t6071,t6072,t6073,t6076,t6078,t608,t6081,t6082,t6086,t6087,t6089,t609,t6091,t6092,t6093,t6094,t6096,t6097,t61,t610,t6101,t6106,t6109,t611,t6111,t6112,t6114,t6115,t6116,t6117,t6119,t6120,t6124,t6125,t6126,t6127,t6128,t6129,t6130,t6131,t6132,t6134,t6135,t6136,t6138,t6139,t614,t6140,t6141,t6142,t6145,t6146,t6147,t6149,t6150,t6151,t6152,t6153,t6154,t6156,t6157,t6160,t6161,t6162,t6163,t6164,t6166,t6167,t6168,t6169,t6175,t6176,t6178,t6179,t6180,t6182,t6183,t6184,t6185,t6186,t6187,t6188,t6191,t6192,t6193,t6195,t6196,t62,t6201,t6203,t6204,t6207,t6211,t6213,t6214,t6216,t6218,t6219,t6222,t6224,t6225,t6226,t6229,t6231,t6234,t6235,t6236,t6237,t6241,t6242,t6244,t6248,t6252,t6253,t6254,t6255,t6256,t6257,t6258,t6261,t6262,t6263,t6264,t6265,t6266,t6267,t6268,t6269,t6270,t6272,t6274,t6275,t6277,t6278,t6293,t6294,t6296,t6298,t6299,t63,t6300,t6302,t6303,t6305,t6306,t6307,t6308,t6309,t6312,t6313,t6316,t6317,t6319,t6321,t6323,t6327,t6328,t6332,t6333,t6335,t6337,t6339,t634,t6340,t6342,t6344,t6346,t6349,t635,t6350,t6352,t6353,t6354,t6355,t6356,t6357,t6358,t636,t6360,t6363,t6364,t6365,t6366,t6368,t6369,t637,t6370,t6372,t6373,t6375,t6376,t6377,t6378,t6379,t638,t6383,t6385,t6386,t6388,t6389,t639,t6390,t6391,t6395,t6398,t640,t6400,t6401,t6403,t6404,t6405,t6407,t641,t6411,t6412,t6417,t6418,t6421,t6422,t6423,t6424,t6425,t6426,t6427,t6429,t6434,t6435,t6436,t6437,t6438,t6440,t6441,t6442,t6443,t6445,t6446,t6447,t6448,t6449,t6451,t6452,t6454,t6455,t6456,t6457,t6460,t6461,t6462,t6469,t647,t6470,t6473,t6475,t6481,t6483,t6484,t6485,t6486,t6487,t6488,t649,t6490,t6491,t6492,t6493,t6494,t6497,t6499,t650,t6500,t6501,t6502,t6505,t6509,t651,t6510,t6513,t6516,t6517,t652,t6520,t6521,t6522,t6523,t6525,t6526,t6527,t6528,t6529,t653,t6530,t6531,t6532,t6533,t6534,t6537,t6538,t6539,t6540,t6541,t6542,t6543,t6544,t6545,t6547,t6548,t6549,t6557,t6558,t6560,t6561,t6562,t6563,t6564,t657,t6570,t6574,t6575,t6576,t6579,t658,t6580,t6582,t6583,t6585,t6586,t6588,t6589,t659,t6592,t6594,t6595,t6596,t6597,t6599,t660,t6600,t6602,t6603,t6604,t6606,t6607,t6608,t6609,t661,t6610,t6611,t6612,t6613,t6614,t6616,t6618,t6619,t6621,t6624,t6625,t6628,t6629,t663,t6632,t6634,t6635,t6637,t6638,t6639,t664,t6640,t6642,t6644,t6645,t6646,t6647,t6648,t6649,t6650,t6651,t6655,t6657,t6658,t6659,t6662,t6664,t6665,t6667,t6668,t6669,t667,t6670,t6673,t6674,t6675,t6676,t6678,t6679,t6680,t6681,t6682,t6685,t6686,t6687,t6689,t6690,t6692,t6693,t6695,t6696,t6697,t6699,t670,t6700,t6701,t6702,t6703,t6704,t6705,t6706,t6707,t6710,t6711,t6712,t6715,t6716,t6719,t6721,t6722,t6725,t6726,t6727,t6732,t6733,t6734,t6736,t6738,t6739,t6740,t6741,t6742,t6744,t6746,t6747,t6750,t6754,t6755,t6757,t6758,t6759,t676,t6760,t6763,t6764,t6766,t6767,t677,t6770,t6771,t6772,t6775,t6776,t6779,t678,t6783,t6784,t6786,t6790,t6792,t6793,t6796,t6797,t6799,t680,t6800,t6805,t6806,t6807,t6808,t6809,t681,t6810,t6813,t6817,t6821,t6822,t6823,t6824,t6826,t6829,t683,t6830,t6831,t6834,t6838,t6839,t684,t6840,t6841,t6842,t6843,t6845,t6849,t685,t6853,t6856,t6857,t6859,t686,t6860,t6862,t6863,t6866,t6867,t687,t6870,t6871,t6872,t6874,t6875,t6877,t6878,t688,t6880,t6884,t6885,t6887,t6889,t6890,t6891,t6896,t6897,t6898,t690,t6901,t6902,t6903,t6904,t6905,t6906,t6908,t6909,t691,t6910,t6911,t6914,t692,t6924,t6925,t6927,t6928,t6929,t693,t6930,t6931,t6932,t6933,t6934,t6935,t6937,t6938,t6939,t6940,t6941,t6942,t6944,t6946,t6947,t6948,t6949,t6956,t6959,t696,t6960,t6961,t6965,t6966,t6974,t6975,t6976,t6977,t6978,t6979,t6981,t6982,t6983,t6984,t6987,t6989,t6990,t6991,t6998,t6999,t7,t700,t7001,t7002,t7003,t7010,t7011,t7012,t7013,t7016,t7017,t7018,t7019,t702,t7020,t7021,t7022,t7023,t7024,t7025,t7026,t7027,t7028,t703,t7031,t7032,t7033,t7034,t7035,t7039,t7042,t7043,t7044,t7048,t7049,t7050,t7051,t7052,t7054,t7055,t7056,t7057,t7059,t7060,t7061,t7062,t7063,t7064,t7065,t7066,t7069,t7074,t7075,t7078,t7080,t7081,t7083,t7086,t7088,t7090,t7093,t7094,t7097,t7100,t7101,t7102,t7104,t7107,t7108,t7109,t7110,t7111,t7113,t7115,t7117,t7118,t7119,t7122,t7123,t7124,t7125,t7127,t7128,t7129,t7130,t7131,t7132,t7134,t7135,t7136,t7137,t7138,t7141,t7143,t7144,t7146,t7147,t7152,t7153,t7155,t7156,t7163,t7165,t7166,t7168,t7170,t7173,t7174,t7176,t7178,t7180,t7182,t7185,t7186,t7188,t7189,t7190,t7191,t7192,t7193,t7194,t7198,t7199,t7200,t7201,t7203,t7205,t7206,t7207,t7208,t7209,t7210,t7212,t7213,t7216,t7220,t7221,t7222,t7223,t7224,t7225,t7226,t7227,t7228,t7229,t7230,t7231,t7232,t7233,t7238,t7239,t7241,t7246,t7250,t7251,t7253,t7254,t7256,t7257,t7258,t7259,t7260,t7263,t7265,t7266,t7267,t7268,t7272,t7276,t7278,t728,t7282,t7283,t7284,t7285,t7286,t7288,t7289,t7292,t7297,t7298,t7299,t7300,t7301,t7302,t7303,t7304,t7305,t7306,t7307,t7308,t7309,t7311,t7313,t7315,t7316,t7318,t7319,t7320,t7323,t7327,t7329,t7330,t7331,t7332,t7333,t7334,t7335,t7336,t7337,t7340,t7342,t7343,t7344,t7345,t7346,t7348,t7349,t735,t7357,t7358,t736,t7361,t7362,t7363,t7365,t7366,t7367,t7368,t7369,t7370,t7371,t7372,t7373,t7378,t738,t7384,t7385,t7393,t7394,t7395,t7396,t7397,t7398,t7399,t740,t7400,t7401,t7402,t7403,t7405,t7407,t7408,t7409,t7411,t7412,t7413,t7414,t7415,t7416,t7417,t7419,t7420,t7422,t7423,t7425,t7428,t7429,t7430,t7431,t7432,t7433,t7434,t7438,t7441,t7442,t7443,t7446,t7447,t7449,t7450,t7451,t7452,t7457,t746,t7460,t7461,t7463,t7464,t7465,t7466,t7467,t7469,t747,t7470,t7471,t7473,t7474,t7475,t7477,t7478,t7479,t748,t7480,t7481,t7494,t7500,t7505,t7507,t7511,t7513,t7516,t7518,t7519,t752,t7524,t7525,t7526,t7529,t7530,t7532,t7534,t7535,t7536,t7537,t754,t7541,t7542,t7547,t7549,t7550,t7554,t7555,t7557,t7559,t756,t7564,t7566,t7571,t7575,t7578,t7579,t758,t7589,t759,t7590,t7594,t7595,t7596,t7597,t7598,t7599,t7600,t7601,t7602,t7607,t7608,t7620,t7621,t7634,t7636,t7644,t7649,t7651,t7652,t7655,t7656,t7657,t7658,t7659,t766,t7660,t7661,t7663,t7664,t7667,t7672,t7673,t7674,t7675,t7678,t768,t7686,t7687,t7690,t772,t7721,t7722,t7725,t7735,t7751,t7756,t7757,t7764,t7765,t7769,t7788,t7790,t7793,t7795,t7802,t7807,t781,t7810,t782,t7825,t7827,t7833,t7872,t7877,t7897,t7902,t7904,t7914,t7924,t793,t7961,t7962,t7966,t7971,t7976,t798,t7983,t7999,t8,t8002,t8021,t8038,t8046,t8050,t8051,t8052,t8090,t8096,t8117,t8126,t8129,t8130,t8182,t8184,t8202,t8206,t8231,t8232,t8239,t826,t827,t828,t829,t832,t833,t834,t836,t837,t838,t839,t84,t85,t850,t852,t86,t861,t864,t868,t87,t879,t884,t885,t888,t889,t890,t891,t892,t893,t894,t897,t898,t9,t90,t900,t901,t902,t904,t905,t906,t907,t911,t912,t913,t914,t915,t916,t917,t918,t92,t929,t930,t931,t933,t934,t936,t938,t940,t943,t944,t945,t947,t949,t950,t951,t953,t956,t957,t966,t967,t968,t969,t97,t972,t973,t974,t976,t98,t981,t982,t984,t986,t988,t99,t992,t993,t994,t997,t999] = ct{:};
t7350 = t4.*t49.*t7340;
t7351 = t7349.*3.0;
t7355 = -t7349;
t7376 = t690.*t7340;
t7377 = t7373.*3.0;
t7386 = t1252.*t7340;
t7387 = t1253.*t7340;
t7388 = t7384.*3.0;
t7389 = t7385.*3.0;
t7418 = t6733+t6890+t6896;
t7435 = t4.*t7431;
t7436 = t10.*t7431;
t7437 = t4.*t7432;
t7476 = t6813+t7080+t7093;
t7486 = t6874+t7081+t7094;
t7489 = -t8.*t9.*(t6874+t7086+t3756.*(t3923-t6597));
t7490 = -t2.*t3.*(-t6862+t7059+t3710.*(t3626-t6712));
t7491 = t2.*t9.*(-t6862+t7059+t3710.*(t3626-t6712));
t7493 = t3.*t8.*(t6874+t7086+t3756.*(t3923-t6597));
t7495 = -t3.*t48.*(-t6862+t7059+t3710.*(t3626-t6712));
t7498 = t3.*t53.*(t6874+t7086+t3756.*(t3923-t6597));
t7504 = t4.*t7500;
t7515 = -t687.*(t6874+t7086+t3756.*(t3923-t6597));
t7517 = t4.*t7511;
t7522 = t4.*t7505;
t7527 = -t1251.*(-t6862+t7059+t3710.*(t3626-t6712));
t7540 = -t1703.*(t6874+t7086+t3756.*(t3923-t6597));
t7544 = t1661.*(-t6862+t7059+t3710.*(t3626-t6712));
t7568 = -t3754.*(-t6862+t7059+t3710.*(t3626-t6712));
t7570 = t3060.*(t6874+t7086+t3756.*(t3923-t6597));
t7573 = t6944+t7226+t7272;
t7574 = t6956+t7246+t7256;
t7606 = t9.*t7601;
t7615 = t3.*t4.*t7601;
t7639 = t690.*t7601;
t7662 = t690.*(t6739+t6747-t6779-t6810+t12.*t690.*(t97-t1942).*1.35e-3+t12.*t690.*(t1387-t3956)).*(-1.0./2.0);
t7665 = (t690.*(t6739+t6747-t6779-t6810+t12.*t690.*(t97-t1942).*1.35e-3+t12.*t690.*(t1387-t3956)))./2.0;
t7666 = t690.*(t5454+t6721+t6822+t6823+t2028.*(t1387-t3956)+t6456.*(t97-t1942)).*(-1.0./2.0);
t7682 = t9.*t7674;
t7684 = t3.*t4.*t7674;
t7697 = t690.*t7674;
t7701 = t6738+t6746+t6867+t6875+t6878+t6891;
t7728 = t7136+t7170+t7173+t7174;
t7736 = t9.*t7735;
t7738 = t3.*t4.*t7735;
t7760 = t690.*t7735;
t7762 = t6838+t6857+t6866+t6872+t6965+t6984;
t7767 = t6725+t6783+t6977+t6990+t7033+t7035;
t7771 = t6727+t6793+t6983+t6991+t7023+t7034;
t7773 = t3709.*(t6800+t6805-t6877-t6908+t6.*t690.*(t1552-t4983).*1.0675e-2+t12.*t3709.*(t1387-t3956)).*(-1.0./2.0);
t7774 = t3755.*(t6796-t6808-t6889+t6897+t6909+t12.*t690.*(t1928-t4165).*1.35e-3).*(-1.0./2.0);
t7775 = (t3709.*(t6800+t6805-t6877-t6908+t6.*t690.*(t1552-t4983).*1.0675e-2+t12.*t3709.*(t1387-t3956)))./2.0;
t7786 = t6758+t6807+t6931+t6941+t7083+t7100;
t7791 = t6792+t6809+t6982+t7003+t7018+t7022;
t7792 = t6766+t6817+t6928+t6939+t7056+t7119;
t7811 = t3.*t8.*(t6792+t6809-t6979+t6982+t7022+t7025);
t7812 = -t2.*t3.*(t7250+t7263+t6821.*(t1552-t4983)+t6740.*(t3242-t6692));
t7817 = t3755.*(t6842+t6856+t6860-t6872-t6961+t12.*t690.*(t3923-t6597)).*(-1.0./2.0);
t7818 = t6759+t6871+t6932+t6942+t7069+t7111;
t7822 = (t3709.*(-t6841+t6863+t6870-t6934+t12.*t3709.*(t97-t1942).*1.35e-3+t6.*t690.*(t3626-t6712)))./2.0;
t7824 = t3709.*(t6834-t6843+t6863+t6870-t6959+t1664.*(t3626-t6712));
t7826 = -t2.*t3.*(t6767+t6887+t6930-t7039+t3756.*(t1761-t5472)+t3757.*(t3626-t6712));
t7840 = t1250.*(t6792+t6809-t6979+t6982+t7022+t7025);
t7844 = t688.*(t7250+t7263+t6821.*(t1552-t4983)+t6740.*(t3242-t6692));
t7845 = -t688.*(t6767+t6887+t6930-t7039+t3756.*(t1761-t5472)+t3757.*(t3626-t6712));
t7867 = t6758+t6807+t7012+t7028+t7168+t7178;
t7871 = -t3709.*(t6767+t6887+t6930-t7039+t3756.*(t1761-t5472)+t3757.*(t3626-t6712));
t7888 = t6925+t6975+t7013+t7032+t7078+t7115;
t7891 = -t3.*t8.*(t6927+t6938-t7001-t7108+t12.*t3755.*(t1928-t4165).*1.35e-3+t12.*t3755.*(t3923-t6597));
t7900 = t6831+t6901+t7134+t7143+t7152+t7163;
t7903 = t6853+t6904+t7146+t7147+t7155+t7156;
t7908 = -t2.*t3.*(t6829-t6885-t7144-t7153+t6821.*(t193-t2663)+t6151.*(t3626-t6712));
t7909 = -t688.*(t6946+t6948-t6987-t7075+t6.*t3709.*(t1552-t4983).*1.0675e-2+t6.*t3709.*(t3626-t6712));
t7910 = t1250.*(t6927+t6938-t7001-t7108+t12.*t3755.*(t1928-t4165).*1.35e-3+t12.*t3755.*(t3923-t6597));
t7918 = t688.*(t6829-t6885-t7144-t7153+t6821.*(t193-t2663)+t6151.*(t3626-t6712));
t7920 = t3755.*(t6927+t6938-t7001-t7108+t12.*t3755.*(t1928-t4165).*1.35e-3+t12.*t3755.*(t3923-t6597));
t7928 = t6840+t6902+t7186+t7194+t7199+t7208;
t7935 = -t2.*t3.*(t6826+t6880-t7180-t7182-t7216+t6797.*(t1552-t4983));
t8035 = t3.*(-t7450+t3755.*(t6874+t7086+t3756.*(t3923-t6597))+t3709.*(-t6862+t7059+t3710.*(t3626-t6712))).*(-1.0./2.0);
t8037 = t4.*t9.*(-t7450+t3755.*(t6874+t7086+t3756.*(t3923-t6597))+t3709.*(-t6862+t7059+t3710.*(t3626-t6712))).*(-1.0./2.0);
t8097 = dq2.*t8096;
t8131 = t187+t332+t355+t518+t888+t918+t1037+t1084+t1186+t1188+t1293+t1377+t1385+t1493+t1571+t1691+t1759+t1823+t1944+t2379+t2645+t2801+t2864+t2959+t3125+t3206+t3286+t3342+t3387+t3412+t3504+t3601+t3921+t3949+t4210+t4325+t4367+t4369+t4455+t4532+t4542+t4731+t4859+t4872+t4909+t4924+t5116+t5164+t5207+t5243+t5425+t5490+t5559+t5569+t5634+t5674+t5704+t5800+t5806+t5842+t5931+t5992+t6066+t6175+t6203+t6264+t6398+t6637;
t8183 = dq2.*t8182;
t8233 = dq1.*t8232;
t8234 = t1866+t2524+t2644+t2649+t2763+t2927+t2991+t3138+t3303+t3332+t3484+t3508+t3554+t3575+t3670+t3737+t3778+t3781+t3785+t3948+t4066+t4067+t4154+t4175+t4262+t4263+t4368+t4375+t4566+t4569+t4619+t4623+t4668+t4702+t4739+t4768+t4813+t4964+t4967+t5014+t5071+t5073+t5074+t5149+t5170+t5176+t5219+t5246+t5332+t5357+t5385+t5397+t5455+t5495+t5507+t5518+t5549+t5550+t5592+t5600+t5644+t5703+t5726+t5734+t5845+t5861+t5866+t5870+t5907+t5916+t5980+t5982+t6004+t6005+t6048+t6086+t6127+t6147+t6149+t6162+t6163+t6187+t6192+t6229+t6308+t6376+t6379+t6412+t6425+t6426+t6454+t6462+t6499+t6500+t6501+t6520+t6527+t6539+t6582+t6588+t6595+t6616+t6664+t6699+t7793;
t8237 = t229+t334+t967+t984+t993+t1024+t1133+t1204+t1207+t1219+t1228+t1317+t1364+t1375+t1427+t1433+t1477+t1508+t1513+t1637+t1639+t1701+t1853+t1901+t1902+t1920+t1993+t2013+t2055+t2059+t2083+t2085+t2140+t2202+t2283+t2415+t2430+t2431+t2466+t2628+t2729+t2740+t2965+t3010+t3131+t3192+t3231+t3232+t3236+t3265+t3296+t3324+t3410+t3590+t3638+t3639+t3648+t3674+t3681+t3682+t3721+t3722+t3727+t3857+t3898+t3930+t3959+t4075+t4150+t4278+t4308+t4381+t4417+t4474+t4475+t4476+t4520+t4545+t4565+t4718+t4736+t4792+t4873+t4887+t4892+t4972+t5086+t5125+t5141+t5241+t5280+t5289+t5308+t5341+t5353+t5392+t5399+t5401+t5402+t5423+t5457+t5499+t5575+t5656+t5657+t5671+t5711+t5745+t5773+t5774+t5775+t5847+t5871+t5884+t5901+t5961+t5973+t5998+t6016+t6027+t6047+t6067+t6069+t6087+t6119+t6125+t6211+t6236+t6252+t6254+t6261+t6309+t6346+t6372+t6388+t6427+t6448+t6455+t6470+t6485+t6491+t6589+t6592+t6639+t6647+t6650+t6697+t6734+t6744+t6750;
t8238 = t255+t344+t349+t434+t435+t657+t838+t902+t929+t931+t938+t947+t953+t976+t1027+t1079+t1092+t1120+t1153+t1201+t1203+t1227+t1285+t1291+t1357+t1395+t1397+t1420+t1422+t1429+t1464+t1595+t1694+t1726+t1730+t1752+t1764+t1799+t1835+t1908+t2000+t2147+t2234+t2319+t2364+t2437+t2438+t2471+t2499+t2566+t2735+t2765+t2803+t2812+t2813+t2828+t2973+t3065+t3067+t3095+t3119+t3273+t3275+t3305+t3402+t3458+t3483+t3526+t3527+t3532+t3623+t3700+t3701+t3704+t3712+t3759+t3782+t3787+t3821+t3822+t3989+t3990+t4043+t4059+t4104+t4115+t4118+t4172+t4192+t4327+t4415+t4439+t4505+t4511+t4541+t4549+t4564+t4578+t4601+t4667+t4720+t4735+t4791+t4819+t4863+t4905+t4907+t4935+t4937+t4977+t5001+t5020+t5043+t5065+t5108+t5109+t5127+t5174+t5239+t5284+t5319+t5429+t5430+t5459+t5469+t5500+t5505+t5506+t5591+t5652+t5659+t5661+t5737+t5786+t5811+t5814+t5841+t5851+t5854+t5862+t5868+t5882+t5991+t6046+t6078+t6096+t6124+t6142+t6154+t6166+t6222+t6274+t6306+t6316+t6350+t6373+t6375+t6492+t6494+t6502+t6606+t6613+t6700+t6754;
t8240 = t752+t914+t944+t1344+t1359+t1368+t1380+t1389+t1424+t1445+t1517+t1547+t1556+t1576+t1641+t1645+t1727+t1739+t1750+t1760+t1771+t1776+t1847+t1899+t1903+t1914+t1936+t1994+t2006+t2009+t2044+t2075+t2079+t2084+t2089+t2107+t2110+t2203+t2219+t2323+t2413+t2552+t2641+t2747+t2919+t2968+t2981+t3280+t3334+t3523+t3544+t3548+t3687+t3736+t3789+t3926+t3944+t3965+t4068+t4221+t4260+t4362+t4365+t4388+t4466+t4512+t4639+t4683+t4695+t4740+t4762+t4763+t4812+t4832+t4910+t4912+t4962+t4985+t5042+t5067+t5080+t5151+t5169+t5185+t5189+t5247+t5263+t5354+t5359+t5494+t5512+t5519+t5599+t5616+t5636+t5641+t5651+t5696+t5697+t5716+t5733+t5761+t5815+t5843+t5859+t5873+t5888+t5909+t5934+t5942+t5954+t5988+t6001+t6002+t6030+t6072+t6076+t6081+t6111+t6114+t6164+t6185+t6226+t6267+t6294+t6298+t6300+t6305+t6332+t6333+t6354+t6370+t6378+t6389+t6411+t6417+t6429+t6438+t6446+t6451+t6483+t6488+t6510+t6516+t6525+t6529+t6541+t6547+t6561+t6574+t6579+t6583+t6594+t6624+t6642+t6667+t6673+t6681+t6685+t6689+t6693+t6703+t6715+t6772;
t8243 = t141+t143+t636+t683+t685+t691+t693+t884+t1095+t1096+t1132+t1198+t1211+t1222+t1284+t1295+t1325+t1345+t1346+t1368+t1492+t1494+t1495+t1524+t1576+t1673+t1745+t1753+t1771+t1779+t1796+t1800+t1801+t1832+t1833+t1836+t1844+t1896+t1911+t1936+t2001+t2117+t2118+t2133+t2136+t2206+t2295+t2325+t2469+t2479+t2559+t2583+t2585+t2593+t2822+t2863+t2933+t2934+t2956+t3077+t3213+t3214+t3399+t3424+t3496+t3621+t3653+t3683+t3684+t3705+t3725+t3726+t3769+t3839+t3840+t3939+t3941+t3977+t4061+t4078+t4109+t4149+t4258+t4352+t4354+t4408+t4456+t4521+t4568+t4589+t4612+t4617+t4621+t4686+t4691+t4722+t4776+t4777+t4795+t4799+t4826+t4855+t4856+t4955+t4957+t4958+t5054+t5069+t5081+t5097+t5121+t5122+t5210+t5231+t5257+t5322+t5343+t5344+t5407+t5408+t5410+t5421+t5439+t5486+t5517+t5533+t5551+t5570+t5572+t5589+t5590+t5690+t5692+t5741+t5766+t5770+t5781+t5833+t5835+t5886+t5890+t5944+t5947+t5979+t5985+t6008+t6020+t6021+t6039+t6097+t6129+t6131+t6135+t6191+t6207+t6219+t6224+t6241+t6253+t6255+t6275+t6293+t6319+t6321+t6323+t6337+t6421+t6422+t6437+t6440+t6484+t6493+t6521+t6522+t6532+t6537+t6544+t6545+t6558+t6585+t6599+t6609+t6614+t6619+t6628+t6649+t6651+t6658+t6668+t6669+t6674+t6679+t6687+t6704+t6710+t6711;
et1 = t249+t308+t352+t490+t514+t614+t658+t754+t915+t956+t967+t968+t993+t1115+t1129+t1150+t1204+t1219+t1228+t1229+t1317+t1318+t1331+t1351+t1364+t1390+t1405+t1426+t1427+t1441+t1470+t1508+t1513+t1581+t1583+t1615+t1637+t1639+t1669+t1701+t1707+t1716+t1778+t1853+t1901+t1902+t1917+t1920+t1922+t1993+t2013+t2059+t2083+t2140+t2202+t2216+t2245+t2283+t2415+t2430+t2453+t2481+t2525+t2701+t2725+t2740+t2923+t2965+t3010+t3011+t3049+t3092+t3109+t3131+t3198+t3231+t3232+t3265+t3269+t3296+t3298+t3324+t3590+t3591+t3620+t3638+t3645+t3648+t3681+t3682+t3694+t3721+t3722+t3727+t3741+t3744+t3748+t3774+t3798+t3806+t3857+t3930+t3959+t4001+t4025+t4031+t4032+t4057+t4074+t4075+t4088+t4176+t4178+t4216+t4224+t4246+t4278+t4381+t4469+t4474+t4503+t4517+t4520+t4565+t4608+t4699+t4718+t4736+t4744+t4753+t4789+t4792+t4793+t4815+t4828+t4873+t4887+t4888+t4892+t4965+t4972+t4990+t4992+t5034+t5125+t5141+t5213+t5221+t5253+t5280+t5308+t5348+t5353+t5369+t5380+t5392+t5399+t5401+t5402+t5457+t5460+t5473+t5499+t5544+t5575+t5578+t5604+t5607+t5656+t5657+t5670+t5671+t5682+t5711+t5725+t5745+t5773+t5774+t5810+t5847+t5871+t5884+t5901+t5903+t5919+t5973+t6027+t6036+t6047+t6067+t6069+t6087+t6094+t6119+t6125+t6193+t6211+t6236+t6252+t6254;
et2 = t6256+t6261+t6309+t6339+t6346+t6372+t6388+t6427+t6448+t6455+t6470+t6485+t6491+t6589+t6592+t6607+t6639+t6647+t6650+t6697+t6742+t6744+t6750;
t8245 = et1+et2;
t7195 = t7188.*3.0;
t7196 = t7189.*3.0;
t7197 = t7190.*3.0;
t7211 = t7203.*3.0;
t7249 = t7238.*3.0;
t7252 = -t7241;
t7269 = t7258.*3.0;
t7270 = t7259.*3.0;
t7271 = t7260.*3.0;
t7290 = t7283.*3.0;
t7293 = -t7288;
t7294 = t7289.*3.0;
t7295 = -t7289;
t7310 = t7308.*3.0;
t7321 = -t7319;
t7322 = t7318.*3.0;
t7324 = -t7318;
t7354 = t7350.*3.0;
t7356 = -t7351;
t7359 = -t7350;
t7383 = t7376.*3.0;
t7390 = t7386.*3.0;
t7391 = t7387.*3.0;
t7424 = (t4.*t49.*t7418)./2.0;
t7427 = t690.*t7418;
t7439 = (t1252.*t7418)./2.0;
t7440 = (t1253.*t7418)./2.0;
t7453 = t7124+t7308;
t7520 = (t1703.*t7476)./2.0;
t7531 = (t2027.*t7476)./2.0;
t7543 = t7258+t7376;
t7545 = t7260+t7373;
t7552 = (t3060.*t7476)./2.0;
t7556 = (t1703.*t7486)./2.0;
t7562 = (t2027.*t7486)./2.0;
t7572 = (t3060.*t7486)./2.0;
t7580 = t2.*t3.*t7573;
t7581 = t2.*t9.*t7573;
t7582 = t3.*t8.*t7573;
t7583 = t2.*t3.*t7574;
t7584 = t3.*t8.*t7574;
t7585 = t8.*t9.*t7574;
t7586 = t3.*t48.*t7573;
t7593 = t3.*t53.*t7574;
t7603 = t687.*t7574;
t7604 = t688.*t7574;
t7605 = t688.*t7573;
t7610 = t1250.*t7574;
t7612 = t1250.*t7573;
t7613 = t1251.*t7573;
t7618 = t1703.*t7574;
t7625 = t1661.*t7573;
t7626 = t1662.*t7573;
t7629 = t2027.*t7574;
t7638 = t3060.*t7574;
t7640 = t3755.*t7574;
t7641 = t3709.*t7573;
t7642 = t3754.*t7573;
t7643 = t3755.*t7573;
t7645 = t3709.*t7574;
t7692 = t7057+t7101+t7102+t7110;
t7698 = t7054+t7090+t7107+t7135;
t7718 = t1250.*(t7060-t7088+t7104+t3710.*(t3923-t6597));
t7719 = (t690.*t7701)./2.0;
t7732 = t9.*t7728;
t7734 = t3.*t4.*t7728;
t7744 = -t7738;
t7749 = t690.*t7728;
t7770 = t3.*t8.*t7762;
t7777 = t1250.*t7762;
t7783 = t6784+t6806+t6981+t7002+t7017+t7021;
t7799 = t7227+t7253+t7265+t7284;
t7800 = t7228+t7254+t7266+t7285;
t7805 = -t2.*t3.*(t6784+t6806-t6978+t6981+t7021+t7024);
t7808 = t3755.*t7762;
t7815 = t6759+t6871+t6924+t6933+t7074+t7113;
t7823 = t6767+t6887+t6929+t6940+t7055+t7118;
t7828 = (t3709.*t7767)./2.0;
t7834 = (t3755.*t7771)./2.0;
t7836 = t688.*(t6784+t6806-t6978+t6981+t7021+t7024);
t7851 = t7044+t7259+t7292+t7387;
t7853 = (t3755.*t7786)./2.0;
t7856 = (t3755.*t7791)./2.0;
t7864 = (t3709.*t7792)./2.0;
t7865 = t3755.*(t7257+t7267+t6824.*(t1928-t4165)+t6741.*(t3923-t6597));
t7873 = t9.*t7867;
t7876 = t3.*t4.*t7867;
t7878 = (t3755.*t7818)./2.0;
t7884 = t690.*t7867;
t7890 = t6937+t6974+t6989+t7031+t7117+t7125;
t7892 = t2.*t3.*t7888;
t7905 = t688.*t7888;
t7906 = t3.*t8.*t7900;
t7911 = t3.*t8.*t7903;
t7917 = t1250.*t7900;
t7919 = t3709.*t7888;
t7921 = t1250.*t7903;
t7926 = t3755.*t7900;
t7929 = t3755.*t7903;
t7932 = t6839+t6884+t7185+t7191+t7207+t7231;
t7933 = t6830+t6898+t7192+t7193+t7198+t7232;
t7934 = t3.*t8.*t7928;
t7940 = t1250.*t7928;
t7944 = t3755.*t7928;
t7949 = t2.*t7299.*(t7238-t7278-t7385+t3755.*(t166+t298+t2276-t2308)).*(-3.0./2.0);
t7960 = t6976+t7268+t7276+t7573;
t7973 = ((t7238-t7278-t7385+t3755.*(t166+t298+t2276-t2308)).*(t191.*(6.0./5.0)+t305+t425+t478+t505-t781-t793-t861-t879+t1308+t12.*t84.*(3.0./1.0e+1)-t48.*t128.*(3.0./1.0e+1)))./2.0;
t7989 = t7363.*(t7188+t7233-t7283-t7386).*(-1.0./2.0);
t7990 = (t7363.*(t7188+t7233-t7283-t7386))./2.0;
t7994 = (t7372.*(t7188+t7233-t7283-t7386))./2.0;
t8003 = t7415.*(t7238-t7278-t7385+t3755.*(t166+t298+t2276-t2308)).*(-1.0./2.0);
t8019 = t7419.*(t7188+t7233-t7283-t7386).*(-1.0./2.0);
t8022 = t7432+t7490+t7493;
t8028 = t3.*(t7435+t1250.*(t6874+t7086+t3756.*(t3923-t6597))+t688.*(-t6862+t7059+t3710.*(t3626-t6712))).*(-1.0./2.0);
t8029 = (t3.*(t7435+t1250.*(t6874+t7086+t3756.*(t3923-t6597))+t688.*(-t6862+t7059+t3710.*(t3626-t6712))))./2.0;
t8031 = (t4.*t49.*(t7435+t1250.*(t6874+t7086+t3756.*(t3923-t6597))+t688.*(-t6862+t7059+t3710.*(t3626-t6712))))./2.0;
t8032 = t1252.*(t7435+t1250.*(t6874+t7086+t3756.*(t3923-t6597))+t688.*(-t6862+t7059+t3710.*(t3626-t6712))).*(-1.0./2.0);
t8033 = (t1252.*(t7435+t1250.*(t6874+t7086+t3756.*(t3923-t6597))+t688.*(-t6862+t7059+t3710.*(t3626-t6712))))./2.0;
t8036 = t10.*t8035;
t8137 = t3.*t4.*(t7443-t7667+t3709.*(t6784+t6806-t6978+t6981+t7021+t7024)+t3755.*(t6792+t6809-t6979+t6982+t7022+t7025)+t2027.*(t6874+t7086+t3756.*(t3923-t6597))+t1662.*(-t6862+t7059+t3710.*(t3626-t6712))).*(-1.0./2.0);
t8235 = dq1.*t8234;
t8241 = dq1.*t8240;
t8244 = dq1.*t8243;
t8246 = dq1.*t8245;
et3 = t358+t444+t523+t535+t696+t933+t997+t1001+t1007+t1077+t1205+t1242+t1266+t1347+t1360+t1379+t1419+t1462+t1507+t1516+t1523+t1545+t1546+t1587+t1596+t1643+t1644+t1646+t1656+t1660+t1684+t1751+t1773+t1825+t1837+t1854+t1865+t1906+t1921+t1931+t1937+t1996+t2012+t2015+t2016+t2043+t2045+t2088+t2109+t2129+t2152+t2193+t2221+t2314+t2322+t2327+t2343+t2414+t2480+t2553+t2560+t2648+t2748+t2854+t2899+t2925+t2975+t2988+t2990+t3007+t3039+t3136+t3139+t3144+t3262+t3330+t3333+t3485+t3519+t3543+t3545+t3549+t3587+t3593+t3792+t3809+t3862+t3872+t3892+t3922+t3945+t3964+t4044+t4080+t4095+t4203+t4220+t4261+t4286+t4316+t4374+t4387+t4508+t4515+t4618+t4636+t4646+t4669+t4675+t4679+t4738+t4764+t4765+t4766+t4830+t4844+t4915+t4970+t4996+t5041+t5072+t5079+t5133+t5148+t5150+t5179+t5180+t5181+t5266+t5269+t5350+t5356+t5358+t5398+t5478+t5508+t5564+t5587+t5614+t5615+t5635+t5639+t5642+t5658+t5663+t5675+t5698+t5699+t5710+t5715+t5763+t5764+t5809+t5850+t5860+t5883+t5908+t5935+t5936+t5950+t5955+t5977+t5983+t6003+t6071+t6073+t6082+t6092+t6093+t6106+t6112+t6116+t6126+t6152+t6167+t6168+t6184+t6234+t6248+t6266+t6299+t6303+t6349+t6364+t6377+t6391+t6395+t6401+t6407+t6418+t6423+t6436+t6445+t6452+t6490+t6505+t6517+t6528+t6540+t6548;
et4 = t6560+t6575+t6580+t6596+t6604+t6610+t6611+t6621+t6625+t6645+t6659+t6676+t6680+t6682+t6686+t6690+t6696+t6702+t6716;
t8247 = et3+et4;
et5 = t595+t598+t641+t677+t686+t702+t827+t972+t988+t1002+t1003+t1030+t1078+t1158+t1174+t1179+t1195+t1210+t1215+t1221+t1241+t1247+t1415+t1432+t1443+t1459+t1465+t1466+t1468+t1469+t1480+t1511+t1572+t1659+t1675+t1680+t1685+t1687+t1706+t1710+t1713+t1719+t1732+t1744+t1758+t1762+t1768+t1818+t1819+t1821+t1841+t1845+t1856+t1857+t1882+t1900+t1905+t1909+t1913+t1943+t2029+t2034+t2061+t2090+t2116+t2120+t2134+t2200+t2207+t2228+t2235+t2318+t2326+t2353+t2363+t2488+t2504+t2546+t2582+t2632+t2784+t2887+t2931+t2932+t3130+t3170+t3177+t3203+t3208+t3210+t3212+t3316+t3425+t3498+t3513+t3559+t3596+t3657+t3690+t3708+t3772+t3793+t3796+t3825+t3837+t3838+t3908+t3931+t3935+t3936+t4060+t4062+t4083+t4125+t4131+t4199+t4241+t4264+t4344+t4345+t4347+t4350+t4380+t4459+t4529+t4535+t4570+t4590+t4620+t4625+t4629+t4673+t4676+t4685+t4692+t4749+t4772+t4774+t4851+t4861+t4885+t4895+t4896+t4929+t4953+t5025+t5035+t5038+t5055+t5056+t5070+t5091+t5105+t5200+t5209+t5225+t5258+t5259+t5288+t5294+t5317+t5329+t5390+t5405+t5418+t5435+t5452+t5453+t5474+t5480+t5492+t5514+t5527+t5528+t5534+t5552+t5553+t5565+t5567+t5586+t5613+t5621+t5664+t5681+t5685+t5686+t5755+t5767+t5771+t5777+t5783+t5784+t5797+t5840+t5895+t5899+t5917+t5923+t5924+t5937;
et6 = t5946+t5949+t5978+t6006+t6007+t6019+t6022+t6056+t6062+t6089+t6101+t6128+t6132+t6140+t6146+t6169+t6183+t6195+t6204+t6213+t6214+t6218+t6225+t6231+t6242+t6244+t6307+t6312+t6327+t6328+t6335+t6344+t6353+t6355+t6369+t6383+t6385+t6457+t6469+t6473+t6486+t6497+t6509+t6513+t6530+t6538+t6542+t6543+t6557+t6602+t6608+t6612+t6618+t6629+t6632+t6634+t6644+t6648+t6662+t6670+t6675+t6678+t6701+t6705+t6706+t6707+t6755;
t8249 = et5+et6;
t7296 = -t7294;
t7325 = -t7322;
t7360 = -t7354;
t7445 = -t7439;
t7455 = t7132+t7310;
t7551 = t7269+t7383;
t7553 = t7271+t7377;
t7611 = -t7603;
t7668 = t8.*t6903.*t7543.*(3.0./2.0);
t7669 = t2.*t6903.*t7545.*(3.0./2.0);
t7676 = (t6999.*t7545)./2.0;
t7677 = (t7011.*t7543)./2.0;
t7688 = t8.*t7062.*t7543.*(3.0./2.0);
t7689 = t2.*t7062.*t7545.*(3.0./2.0);
t7702 = t2.*t3.*t7692;
t7704 = (t7201.*t7545)./2.0;
t7706 = (t7210.*t7545)./2.0;
t7707 = (t7206.*t7543)./2.0;
t7708 = t688.*t7692;
t7709 = t7543.*(t200.*(3.0./1.0e+1)+t208.*(6.0./5.0)-t303-t415-t747-t1313+t12.*t105.*(3.0./1.0e+1)+t9.*t748).*(-1.0./2.0);
t7720 = -t7719;
t7723 = t3709.*t7692;
t7739 = (t7332.*t7545)./2.0;
t7741 = (t7337.*t7545)./2.0;
t7742 = (t7336.*t7543)./2.0;
t7743 = (t7543.*(t304+t372+t405+t418-t566-t782+t6278+t6461))./2.0;
t7753 = (t7345.*t7545)./2.0;
t7755 = (t7344.*t7543)./2.0;
t7813 = t2.*t3.*t7800;
t7814 = t3.*t8.*t7799;
t7829 = t3.*t8.*t7815;
t7838 = t688.*t7800;
t7841 = t1250.*t7799;
t7846 = t1250.*t7815;
t7850 = t7042+t7189+t7320+t7359;
t7852 = (t3709.*t7783)./2.0;
t7858 = -t7853;
t7859 = t3709.*t7800;
t7861 = t3755.*t7799;
t7863 = t7043+t7203+t7324+t7355;
t7866 = t7052+t7270+t7293+t7391;
t7875 = t3755.*t7815;
t7879 = -t7878;
t7880 = (t3709.*t7823)./2.0;
t7882 = t7190+t7251+t7295+t7384;
t7896 = t3.*t8.*t7890;
t7912 = t1250.*t7890;
t7923 = t3755.*t7890;
t7937 = t3.*t8.*t7932;
t7938 = t2.*t3.*t7933;
t7941 = t688.*t7933;
t7942 = t1250.*t7932;
t7946 = t3755.*t7932;
t7947 = t3709.*t7933;
t7951 = t8.*t7299.*t7851.*(3.0./2.0);
t7954 = (t2.*t7299.*(t7249-t7282-t7389+t3755.*(t166+t298+t2276-t2308).*3.0))./2.0;
t7963 = t2.*t3.*t7960;
t7965 = t3.*t8.*t7960;
t7968 = t688.*t7960;
t7970 = t1250.*t7960;
t7974 = (t7372.*t7851)./2.0;
t7979 = t3709.*t7960;
t7981 = ((t7249-t7282-t7389+t3755.*(t166+t298+t2276-t2308).*3.0).*(t191.*(2.0./5.0)+t297+t413+t463+t504-t766-t850-t868+t1046+t1300+(t12.*t84)./1.0e+1-(t48.*t128)./1.0e+1))./2.0;
t7982 = t3755.*t7960;
t7993 = t7362.*(t7195+t7239-t7290-t7390).*(-1.0./2.0);
t7997 = t7370.*(t7195+t7239-t7290-t7390).*(-1.0./2.0);
t8004 = t7414.*(t7249-t7282-t7389+t3755.*(t166+t298+t2276-t2308).*3.0).*(-1.0./2.0);
t8007 = (t7419.*t7851)./2.0;
t8020 = t7416.*(t7195+t7239-t7290-t7390).*(-1.0./2.0);
t8023 = (t4.*t9.*t8022)./2.0;
t8024 = (t1252.*t8022)./2.0;
t8025 = (t1253.*t8022)./2.0;
t8040 = t7511+t7584+t7589;
t8041 = t3.*t48.*(-t7580+t9.*(-t6799+t7137+t6786.*(t1552-t4983))+t3.*t8.*(t6947+t6849.*(t1552-t4983)+t6740.*(t3923-t6597))).*(-1.0./2.0);
t8043 = t1250.*(-t7580+t9.*(-t6799+t7137+t6786.*(t1552-t4983))+t3.*t8.*(t6947+t6849.*(t1552-t4983)+t6740.*(t3923-t6597))).*(-1.0./2.0);
t8045 = t1661.*(-t7580+t9.*(-t6799+t7137+t6786.*(t1552-t4983))+t3.*t8.*(t6947+t6849.*(t1552-t4983)+t6740.*(t3923-t6597))).*(-1.0./2.0);
t8054 = t3754.*(-t7580+t9.*(-t6799+t7137+t6786.*(t1552-t4983))+t3.*t8.*(t6947+t6849.*(t1552-t4983)+t6740.*(t3923-t6597))).*(-1.0./2.0);
t8055 = t3755.*(-t7580+t9.*(-t6799+t7137+t6786.*(t1552-t4983))+t3.*t8.*(t6947+t6849.*(t1552-t4983)+t6740.*(t3923-t6597))).*(-1.0./2.0);
t8056 = t2.*t3.*(t7610+t688.*(t6949+t6821.*(t1928-t4165)+t6741.*(t3626-t6712))+t3.*t4.*(t6813+t7165+t6760.*(t1928-t4165))).*(-1.0./2.0);
t8058 = t8.*t9.*(t7610+t688.*(t6949+t6821.*(t1928-t4165)+t6741.*(t3626-t6712))+t3.*t4.*(t6813+t7165+t6760.*(t1928-t4165))).*(-1.0./2.0);
t8059 = t2.*t9.*(t7522+t7605+t1250.*(t6947+t6849.*(t1552-t4983)+t6740.*(t3923-t6597))).*(-1.0./2.0);
t8060 = t3.*t8.*(t7522+t7605+t1250.*(t6947+t6849.*(t1552-t4983)+t6740.*(t3923-t6597))).*(-1.0./2.0);
t8061 = (t2.*t9.*(t7522+t7605+t1250.*(t6947+t6849.*(t1552-t4983)+t6740.*(t3923-t6597))))./2.0;
t8062 = t1703.*(t7610+t688.*(t6949+t6821.*(t1928-t4165)+t6741.*(t3626-t6712))+t3.*t4.*(t6813+t7165+t6760.*(t1928-t4165))).*(-1.0./2.0);
t8063 = t1661.*(t7522+t7605+t1250.*(t6947+t6849.*(t1552-t4983)+t6740.*(t3923-t6597))).*(-1.0./2.0);
t8065 = (t1661.*(t7522+t7605+t1250.*(t6947+t6849.*(t1552-t4983)+t6740.*(t3923-t6597))))./2.0;
t8066 = (t1662.*(t7522+t7605+t1250.*(t6947+t6849.*(t1552-t4983)+t6740.*(t3923-t6597))))./2.0;
t8068 = (t2027.*(t7610+t688.*(t6949+t6821.*(t1928-t4165)+t6741.*(t3626-t6712))+t3.*t4.*(t6813+t7165+t6760.*(t1928-t4165))))./2.0;
t8069 = t3709.*(t7610+t688.*(t6949+t6821.*(t1928-t4165)+t6741.*(t3626-t6712))+t3.*t4.*(t6813+t7165+t6760.*(t1928-t4165))).*(-1.0./2.0);
t8070 = t3755.*(t7522+t7605+t1250.*(t6947+t6849.*(t1552-t4983)+t6740.*(t3923-t6597))).*(-1.0./2.0);
t8071 = (t3755.*(t7522+t7605+t1250.*(t6947+t6849.*(t1552-t4983)+t6740.*(t3923-t6597))))./2.0;
t8072 = t7555+t7640+t7656;
t8073 = t7554+t7641+t7657;
t8099 = t7661+t7805+t7811;
t8101 = (t690.*(t7682-t7770+t2.*t3.*(t6834-t6843+t6863+t6870-t6959+t1664.*(t3626-t6712))))./2.0;
t8118 = t7790+t7891+t7892;
t8120 = t7788+t7905+t7910;
t8132 = t7436+t7515+t7527+t7664+t7836+t7840;
t8140 = t7452+t7568+t7570+t7697+t7808+t7824;
t8185 = t7505+t7581+t7594+t7872+t7904+t7906;
t8189 = (t1250.*(t7585+t7590+t7873+t7908+t7911-t3.*(t6813+t7165+t6760.*(t1928-t4165))))./2.0;
t8190 = t7504+t7586+t7597+t7877+t7914+t7917;
t8192 = (t3755.*(t7585+t7590+t7873+t7908+t7911-t3.*(t6813+t7165+t6760.*(t1928-t4165))))./2.0;
t8194 = t7517+t7593+t7596+t7876+t7918+t7921;
t8199 = t7566+t7638+t7649+t7827+t7919+t7920;
t8216 = t2.*t3.*(t7625+t7634+t7924-t7926+t690.*(t6766+t6817+t7016-t7130+t6760.*(t189-t2612)+t6790.*(t1552-t4983))+t1252.*(-t6799+t7137+t6786.*(t1552-t4983))).*(-1.0./2.0);
t8218 = t3.*t8.*(-t7618-t7884+t7929+t3709.*(t6829-t6885-t7144-t7153+t6821.*(t193-t2663)+t6151.*(t3626-t6712))+t1252.*(t6813+t7165+t6760.*(t1928-t4165))+t1661.*(t6949+t6821.*(t1928-t4165)+t6741.*(t3626-t6712))).*(-1.0./2.0);
t8219 = (t3.*t8.*(-t7618-t7884+t7929+t3709.*(t6829-t6885-t7144-t7153+t6821.*(t193-t2663)+t6151.*(t3626-t6712))+t1252.*(t6813+t7165+t6760.*(t1928-t4165))+t1661.*(t6949+t6821.*(t1928-t4165)+t6741.*(t3626-t6712))))./2.0;
t8221 = t688.*(t7625+t7634+t7924-t7926+t690.*(t6766+t6817+t7016-t7130+t6760.*(t189-t2612)+t6790.*(t1552-t4983))+t1252.*(-t6799+t7137+t6786.*(t1552-t4983))).*(-1.0./2.0);
t8222 = t1250.*(-t7618-t7884+t7929+t3709.*(t6829-t6885-t7144-t7153+t6821.*(t193-t2663)+t6151.*(t3626-t6712))+t1252.*(t6813+t7165+t6760.*(t1928-t4165))+t1661.*(t6949+t6821.*(t1928-t4165)+t6741.*(t3626-t6712))).*(-1.0./2.0);
t8236 = -t8235;
t8242 = -t8241;
t8248 = dq1.*t8247;
t8250 = dq1.*t8249;
t7670 = (t8.*t6903.*t7551)./2.0;
t7671 = (t2.*t6903.*t7553)./2.0;
t7679 = -t7676;
t7680 = -t7677;
t7681 = (t6998.*t7553)./2.0;
t7683 = (t7010.*t7551)./2.0;
t7691 = -t7688;
t7693 = -t7689;
t7695 = (t8.*t7062.*t7551)./2.0;
t7696 = (t2.*t7062.*t7553)./2.0;
t7703 = t7200.*t7553;
t7710 = -t7706;
t7712 = -t7707;
t7713 = t7551.*(t208.*(2.0./5.0)-t295-t402-t736+t772+t1274+(t12.*t105)./1.0e+1-(t12.*t200)./1.0e+1);
t7714 = (t7209.*t7553)./2.0;
t7715 = (t7205.*t7551)./2.0;
t7745 = (t7331.*t7553)./2.0;
t7746 = (t7333.*t7553)./2.0;
t7747 = (t7330.*t7551)./2.0;
t7748 = -t7742;
t7752 = (t7551.*(t296+t369+t397+t404-t562-t768+t6277+t6460))./2.0;
t7758 = (t7343.*t7553)./2.0;
t7759 = (t7342.*t7551)./2.0;
t7835 = -t7829;
t7862 = t7050+t7196+t7321+t7360;
t7870 = t7051+t7211+t7325+t7356;
t7885 = t7197+t7252+t7296+t7388;
t7950 = t8.*t7299.*t7850.*(3.0./2.0);
t7955 = t2.*t7299.*t7863.*(3.0./2.0);
t7956 = (t8.*t7299.*t7866)./2.0;
t7972 = (t7363.*t7850)./2.0;
t7984 = (t7370.*t7866)./2.0;
t7985 = t7863.*(t304+t372+t405+t418-t566+t740+t748-t782+t1309+t1505-t12.*t101.*(3.0./1.0e+1)-t12.*t106.*(3.0./1.0e+1)).*(-1.0./2.0);
t7992 = t7882.*(t304+t372+t405+t418-t566+t740+t748-t782+t1309+t1505-t12.*t101.*(3.0./1.0e+1)-t12.*t106.*(3.0./1.0e+1)).*(-1.0./2.0);
t7995 = (t7882.*(t304+t372+t405+t418-t566+t740+t748-t782+t1309+t1505-t12.*t101.*(3.0./1.0e+1)-t12.*t106.*(3.0./1.0e+1)))./2.0;
t8000 = (t7882.*(t191.*(6.0./5.0)+t305+t425+t478+t505-t781-t793-t861-t879+t1308+t12.*t84.*(3.0./1.0e+1)-t48.*t128.*(3.0./1.0e+1)))./2.0;
t8005 = (t7419.*t7850)./2.0;
t8008 = (t7415.*t7863)./2.0;
t8009 = -t8007;
t8012 = (t7416.*t7866)./2.0;
t8015 = (t7415.*t7882)./2.0;
t8026 = -t8024;
t8042 = (t3.*t53.*t8040)./2.0;
t8044 = (t688.*t8040)./2.0;
t8047 = (t1703.*t8040)./2.0;
t8053 = (t3060.*t8040)./2.0;
t8057 = (t3709.*t8040)./2.0;
t8074 = (t8.*t8072)./2.0;
t8075 = (t2.*t8073)./2.0;
t8077 = (t2.*t3.*t8072)./2.0;
t8080 = (t3.*t8.*t8073)./2.0;
t8081 = t2.*t9.*t8073.*(-1.0./2.0);
t8082 = (t3.*t48.*t8073)./2.0;
t8083 = (t3.*t53.*t8072)./2.0;
t8085 = (t687.*t8072)./2.0;
t8086 = (t688.*t8072)./2.0;
t8087 = (t1250.*t8073)./2.0;
t8088 = (t1251.*t8073)./2.0;
t8092 = t3.*t4.*(t7606-t7702+t3.*t8.*(t7060-t7088+t7104+t3710.*(t3923-t6597))).*(-1.0./2.0);
t8093 = t7615+t7708+t7718;
t8104 = t7732+t7812+t7814;
t8107 = t1250.*(-t7813+t9.*(t7138-t7166+t7176+t6757.*(t1928-t4165))+t3.*t8.*(t7257+t7267+t6824.*(t1928-t4165)+t6741.*(t3923-t6597))).*(-1.0./2.0);
t8108 = t7734+t7841+t7844;
t8113 = (t3.*t8.*(t7838+t1250.*(t7257+t7267+t6824.*(t1928-t4165)+t6741.*(t3923-t6597))+t3.*t4.*(t7138-t7166+t7176+t6757.*(t1928-t4165))))./2.0;
t8115 = t7751+t7859+t7865;
t8121 = (t3755.*t8118)./2.0;
t8123 = t7810+t7909+t7912;
t8125 = (t3709.*(t7896+t9.*(t6800+t6805+t6935-t6960-t6966+t6570.*(t1552-t4983))+t2.*t3.*(t6946+t6948-t6987-t7075+t6.*t3709.*(t1552-t4983).*1.0675e-2+t6.*t3709.*(t3626-t6712))))./2.0;
t8127 = t7795+t7935+t7937;
t8133 = (t690.*t8132)./2.0;
t8141 = (t9.*t8140)./2.0;
t8144 = t7437+t7495+t7498+t7744+t7845+t7846;
t8149 = t7500+t7583+t7598+t7962+t7963;
t8152 = t688.*(t7511+t7582+t7961-t7965+t2.*t3.*(t6947+t6849.*(t1552-t4983)+t6740.*(t3923-t6597))).*(-1.0./2.0);
t8154 = t7451+t7540+t7544+t7760+t7871+t7875;
t8157 = t3709.*(t7511+t7582+t7961-t7965+t2.*t3.*(t6947+t6849.*(t1552-t4983)+t6740.*(t3923-t6597))).*(-1.0./2.0);
t8161 = t7522+t7604+t7620+t7968+t7971;
t8165 = (t2.*t3.*(t7608+t7612-t7970+t688.*(t6947+t6949+t6821.*(t1928-t4165)+t6849.*(t1552-t4983)+t6741.*(t3626-t6712)+t6740.*(t3923-t6597))+t3.*t4.*(t6813+t7165+t6760.*(t1928-t4165))))./2.0;
t8166 = t3709.*(t7608+t7612-t7970+t688.*(t6947+t6949+t6821.*(t1928-t4165)+t6849.*(t1552-t4983)+t6741.*(t3626-t6712)+t6740.*(t3923-t6597))+t3.*t4.*(t6813+t7165+t6760.*(t1928-t4165))).*(-1.0./2.0);
t8168 = (t3709.*(t7608+t7612-t7970+t688.*(t6947+t6949+t6821.*(t1928-t4165)+t6849.*(t1552-t4983)+t6741.*(t3626-t6712)+t6740.*(t3923-t6597))+t3.*t4.*(t6813+t7165+t6760.*(t1928-t4165))))./2.0;
t8170 = t7554+t7645+t7651+t7979+t7983;
t8175 = (t8.*(-t7643+t7976+t7982+t690.*(t6813+t7165+t6760.*(t1928-t4165))+t3709.*(t6947+t6849.*(t1552-t4983)+t6740.*(t3923-t6597))))./2.0;
t8177 = t2.*t3.*(-t7643+t7976+t7982+t690.*(t6813+t7165+t6760.*(t1928-t4165))+t3709.*(t6947+t6849.*(t1552-t4983)+t6740.*(t3923-t6597))).*(-1.0./2.0);
t8178 = (t2.*t3.*(-t7643+t7976+t7982+t690.*(t6813+t7165+t6760.*(t1928-t4165))+t3709.*(t6947+t6849.*(t1552-t4983)+t6740.*(t3923-t6597))))./2.0;
t8181 = (t688.*(-t7643+t7976+t7982+t690.*(t6813+t7165+t6760.*(t1928-t4165))+t3709.*(t6947+t6849.*(t1552-t4983)+t6740.*(t3923-t6597))))./2.0;
t8187 = (t688.*t8185)./2.0;
t8191 = (t3709.*t8185)./2.0;
t8193 = -t8192;
t8195 = (t2.*t3.*t8190)./2.0;
t8197 = (t3.*t8.*t8194)./2.0;
t8200 = (t3709.*t8190)./2.0;
t8203 = (t3755.*t8194)./2.0;
t8204 = (t2.*t8199)./2.0;
t8205 = (t3.*t8.*t8199)./2.0;
t8209 = t8.*(t7559+t7642+t7644-t7923+t3709.*(t6946+t6948-t6987-t7075+t6.*t3709.*(t1552-t4983).*1.0675e-2+t6.*t3709.*(t3626-t6712))+t690.*(t6800+t6805+t6935-t6960-t6966+t6570.*(t1552-t4983))).*(-1.0./2.0);
t8211 = (t2.*t3.*(t7559+t7642+t7644-t7923+t3709.*(t6946+t6948-t6987-t7075+t6.*t3709.*(t1552-t4983).*1.0675e-2+t6.*t3709.*(t3626-t6712))+t690.*(t6800+t6805+t6935-t6960-t6966+t6570.*(t1552-t4983))))./2.0;
t8212 = t7516+t7611+t7621+t7807+t7940+t7941;
t8217 = (t3709.*(t7607-t7613+t7942+t688.*(t6826+t6880-t7180-t7182-t7216+t6797.*(t1552-t4983))+t10.*t7505+t3.*t4.*(t6725+t6783+t6977+t7035-t7048+t7122)))./2.0;
t8224 = t7536+t7629+t7636+t7833+t7944+t7947;
t8227 = (t8.*(t7626+t7825+t7946+t3709.*(t6826+t6880-t7180-t7182-t7216+t6797.*(t1552-t4983))+t2027.*(t6947+t6849.*(t1552-t4983)+t6740.*(t3923-t6597))+t4.*t49.*(-t6799+t7137+t6786.*(t1552-t4983))))./2.0;
t8228 = t688.*(t7626+t7825+t7946+t3709.*(t6826+t6880-t7180-t7182-t7216+t6797.*(t1552-t4983))+t2027.*(t6947+t6849.*(t1552-t4983)+t6740.*(t3923-t6597))+t4.*t49.*(-t6799+t7137+t6786.*(t1552-t4983))).*(-1.0./2.0);
t7711 = t7703./2.0;
t7716 = t7713.*(-1.0./2.0);
t7750 = -t7747;
t7953 = (t8.*t7299.*t7862)./2.0;
t7957 = (t2.*t7299.*t7870)./2.0;
t7958 = -t7956;
t7975 = (t7362.*t7862)./2.0;
t7987 = t7870.*(t296+t369+t397+t404-t562+t728+t738-t768+t1301+t1500-(t12.*t101)./1.0e+1-(t12.*t106)./1.0e+1).*(-1.0./2.0);
t7988 = (t7870.*(t296+t369+t397+t404-t562+t728+t738-t768+t1301+t1500-(t12.*t101)./1.0e+1-(t12.*t106)./1.0e+1))./2.0;
t7998 = t7885.*(t296+t369+t397+t404-t562+t728+t738-t768+t1301+t1500-(t12.*t101)./1.0e+1-(t12.*t106)./1.0e+1).*(-1.0./2.0);
t8001 = t7885.*(t191.*(2.0./5.0)+t297+t413+t463+t504-t766-t850-t868+t1046+t1300+(t12.*t84)./1.0e+1-(t48.*t128)./1.0e+1).*(-1.0./2.0);
t8006 = (t7416.*t7862)./2.0;
t8010 = (t7414.*t7870)./2.0;
t8011 = -t8008;
t8014 = -t8012;
t8016 = (t7414.*t7885)./2.0;
t8017 = -t8015;
t8076 = -t8075;
t8078 = t9.*t8074;
t8079 = t9.*t8075;
t8084 = -t8083;
t8089 = -t8087;
t8094 = (t9.*t8093)./2.0;
t8105 = (t688.*t8104)./2.0;
t8110 = (t2.*t3.*t8108)./2.0;
t8122 = -t8121;
t8134 = -t8133;
t8136 = t7431+t7489+t7491+t7736+t7826+t7835;
t8145 = (t9.*t8144)./2.0;
t8147 = (t690.*t8144)./2.0;
t8151 = (t1250.*t8149)./2.0;
t8155 = (t3755.*t8149)./2.0;
t8158 = (t9.*t8154)./2.0;
t8159 = (t3.*t4.*t8154)./2.0;
t8163 = (t3.*t8.*t8161)./2.0;
t8167 = (t3755.*t8161)./2.0;
t8172 = (t2.*t8170)./2.0;
t8174 = (t3.*t8.*t8170)./2.0;
t8180 = (t1250.*t8170)./2.0;
t8188 = -t8187;
t8196 = -t8195;
t8198 = -t8197;
t8201 = -t8200;
t8220 = (t3755.*t8212)./2.0;
t8226 = (t2.*t8224)./2.0;
t8229 = (t1250.*t8224)./2.0;
t7978 = -t7975;
t8013 = -t8010;
t8018 = -t8016;
t8106 = -t8105;
t8112 = -t8110;
t8138 = (t3.*t4.*t8136)./2.0;
t8142 = (t690.*t8136)./2.0;
t8146 = -t8145;
t8148 = -t8147;
t8153 = -t8151;
t8156 = -t8155;
t8160 = -t8159;
t8169 = -t8167;
t8176 = -t8174;
t8230 = -t8229;
t8253 = t499+t511+t558+t599+t608+t759+t966+t1074+t1090+t1171+t1218+t1299+t1319+t1333+t1365+t1877+t1998+t2347+t2421+t2455+t2604+t2609+t2660+t2753+t2794+t2904+t2922+t2952+t3008+t3087+t3110+t3173+t3222+t3226+t3327+t3476+t3506+t3535+t3628+t3739+t3750+t3812+t3897+t3912+t4006+t4085+t4225+t4230+t4232+t4323+t4330+t4518+t4653+t4698+t4743+t4785+t4801+t4946+t4988+t5026+t5060+t5145+t5301+t5340+t5543+t5602+t5619+t5628+t5801+t5824+t5952+t5963+t6156+t6180+t6365+t7440+t7571+t7572+t7665+t7745+t7752+t7817+t7822+t8004+t8014+t8086+t8089+t8180+t8181;
t8257 = t164+t178+t330+t350+t516+t640+t652+t832+t905+t911+t949+t974+t1038+t1087+t1173+t1434+t1457+t1690+t1879+t2423+t2508+t2591+t2695+t2912+t2940+t3228+t3250+t3287+t3346+t3602+t3613+t3692+t3826+t3900+t4129+t4138+t4546+t4841+t4925+t4932+t5117+t5168+t5279+t5394+t5537+t5584+t5756+t5807+t5976+t5999+t6265+t7300+t7305+t7357+t7409+t7670+t7671+t7681+t7683+t7953+t7957+t7997+t8001+t8035+t8078+t8081+t8158+t8216+t8219+t8226+t8227;
